simulink model "simulator_prototype_v2"  (R2021b)
(part 10 of 13)

t6667 = ct{1873};
t6668 = ct{1874};
t6669 = ct{1875};
t667 = ct{1876};
t6671 = ct{1877};
t6672 = ct{1878};
t6673 = ct{1879};
t6678 = ct{1880};
t6679 = ct{1881};
t668 = ct{1882};
t6680 = ct{1883};
t6681 = ct{1884};
t6687 = ct{1885};
t6688 = ct{1886};
t669 = ct{1887};
t6690 = ct{1888};
t6692 = ct{1889};
t6693 = ct{1890};
t670 = ct{1891};
t6714 = ct{1892};
t6715 = ct{1893};
t6731 = ct{1894};
t6732 = ct{1895};
t674 = ct{1896};
t6745 = ct{1897};
t6747 = ct{1898};
t6750 = ct{1899};
t6751 = ct{1900};
t677 = ct{1901};
t6788 = ct{1902};
t6789 = ct{1903};
t6804 = ct{1904};
t6808 = ct{1905};
t6810 = ct{1906};
t6811 = ct{1907};
t682 = ct{1908};
t6831 = ct{1909};
t6833 = ct{1910};
t684 = ct{1911};
t685 = ct{1912};
t6858 = ct{1913};
t6859 = ct{1914};
t686 = ct{1915};
t6860 = ct{1916};
t6861 = ct{1917};
t6868 = ct{1918};
t6869 = ct{1919};
t687 = ct{1920};
t6877 = ct{1921};
t6881 = ct{1922};
t6882 = ct{1923};
t6883 = ct{1924};
t6894 = ct{1925};
t6896 = ct{1926};
t6897 = ct{1927};
t6901 = ct{1928};
t6902 = ct{1929};
t6903 = ct{1930};
t6905 = ct{1931};
t6906 = ct{1932};
t6913 = ct{1933};
t6916 = ct{1934};
t6918 = ct{1935};
t6919 = ct{1936};
t6920 = ct{1937};
t6921 = ct{1938};
t6922 = ct{1939};
t6923 = ct{1940};
t6924 = ct{1941};
t6941 = ct{1942};
t6962 = ct{1943};
t6963 = ct{1944};
t6965 = ct{1945};
t6966 = ct{1946};
t6968 = ct{1947};
t6974 = ct{1948};
t6976 = ct{1949};
t6978 = ct{1950};
t6979 = ct{1951};
t6980 = ct{1952};
t6981 = ct{1953};
t6984 = ct{1954};
t6987 = ct{1955};
t6994 = ct{1956};
t7003 = ct{1957};
t7005 = ct{1958};
t7007 = ct{1959};
t7010 = ct{1960};
t7011 = ct{1961};
t7014 = ct{1962};
t7016 = ct{1963};
t7019 = ct{1964};
t7020 = ct{1965};
t7021 = ct{1966};
t7028 = ct{1967};
t7029 = ct{1968};
t7035 = ct{1969};
t7041 = ct{1970};
t7042 = ct{1971};
t7043 = ct{1972};
t7054 = ct{1973};
t7055 = ct{1974};
t7057 = ct{1975};
t7059 = ct{1976};
t707 = ct{1977};
t708 = ct{1978};
t7080 = ct{1979};
t7083 = ct{1980};
t7086 = ct{1981};
t7088 = ct{1982};
t7092 = ct{1983};
t7095 = ct{1984};
t7098 = ct{1985};
t71 = ct{1986};
t710 = ct{1987};
t7100 = ct{1988};
t7101 = ct{1989};
t7120 = ct{1990};
t7123 = ct{1991};
t7126 = ct{1992};
t7127 = ct{1993};
t7134 = ct{1994};
t7137 = ct{1995};
t7138 = ct{1996};
t7148 = ct{1997};
t715 = ct{1998};
t7150 = ct{1999};
t7159 = ct{2000};
t716 = ct{2001};
t7160 = ct{2002};
t7162 = ct{2003};
t7164 = ct{2004};
t7166 = ct{2005};
t7168 = ct{2006};
t7169 = ct{2007};
t7170 = ct{2008};
t7171 = ct{2009};
t7195 = ct{2010};
t7197 = ct{2011};
t7199 = ct{2012};
t7203 = ct{2013};
t7204 = ct{2014};
t7205 = ct{2015};
t7208 = ct{2016};
t721 = ct{2017};
t7210 = ct{2018};
t7211 = ct{2019};
t7212 = ct{2020};
t7213 = ct{2021};
t722 = ct{2022};
t7223 = ct{2023};
t7225 = ct{2024};
t7232 = ct{2025};
t7233 = ct{2026};
t724 = ct{2027};
t7246 = ct{2028};
t725 = ct{2029};
t7253 = ct{2030};
t7256 = ct{2031};
t7260 = ct{2032};
t7277 = ct{2033};
t7278 = ct{2034};
t7281 = ct{2035};
t7283 = ct{2036};
t7286 = ct{2037};
t7287 = ct{2038};
t7292 = ct{2039};
t7294 = ct{2040};
t7297 = ct{2041};
t7298 = ct{2042};
t73 = ct{2043};
t7300 = ct{2044};
t7301 = ct{2045};
t7304 = ct{2046};
t7309 = ct{2047};
t7310 = ct{2048};
t7311 = ct{2049};
t7315 = ct{2050};
t7319 = ct{2051};
t7322 = ct{2052};
t7323 = ct{2053};
t7335 = ct{2054};
t7337 = ct{2055};
t7339 = ct{2056};
t7340 = ct{2057};
t7344 = ct{2058};
t7345 = ct{2059};
t7348 = ct{2060};
t7349 = ct{2061};
t7358 = ct{2062};
t7360 = ct{2063};
t7364 = ct{2064};
t7365 = ct{2065};
t7366 = ct{2066};
t7376 = ct{2067};
t7379 = ct{2068};
t7380 = ct{2069};
t7385 = ct{2070};
t7387 = ct{2071};
t7388 = ct{2072};
t7401 = ct{2073};
t7402 = ct{2074};
t7403 = ct{2075};
t7404 = ct{2076};
t7405 = ct{2077};
t7406 = ct{2078};
t7410 = ct{2079};
t7411 = ct{2080};
t7412 = ct{2081};
t7413 = ct{2082};
t7416 = ct{2083};
t7417 = ct{2084};
t7435 = ct{2085};
t7436 = ct{2086};
t7458 = ct{2087};
t7459 = ct{2088};
t7468 = ct{2089};
t7479 = ct{2090};
t749 = ct{2091};
t7501 = ct{2092};
t7514 = ct{2093};
t7531 = ct{2094};
t7553 = ct{2095};
t7554 = ct{2096};
t7555 = ct{2097};
t7560 = ct{2098};
t7561 = ct{2099};
t762 = ct{2100};
t7624 = ct{2101};
t7626 = ct{2102};
t7641 = ct{2103};
t7658 = ct{2104};
t7659 = ct{2105};
t768 = ct{2106};
t7692 = ct{2107};
t7737 = ct{2108};
t777 = ct{2109};
t7784 = ct{2110};
t7789 = ct{2111};
t7790 = ct{2112};
t7827 = ct{2113};
t7828 = ct{2114};
t792 = ct{2115};
t793 = ct{2116};
t8 = ct{2117};
t801 = ct{2118};
t802 = ct{2119};
t808 = ct{2120};
t813 = ct{2121};
t819 = ct{2122};
t821 = ct{2123};
t850 = ct{2124};
t855 = ct{2125};
t874 = ct{2126};
t878 = ct{2127};
t9 = ct{2128};
t941 = ct{2129};
t948 = ct{2130};
t951 = ct{2131};
t97 = ct{2132};
t5423 = t3732+t3736+t4184+t4191;
t5428 = -t5427;
t5430 = t5427./2.0;
t5492 = -t5490;
t5496 = t5490./2.0;
t5547 = t5546./2.0;
t5582 = -t5580;
t5584 = t5580./2.0;
t5643 = -t5642;
t5671 = -t5669;
t5715 = -t5713;
t5767 = t4356+t5365;
t5771 = t4358+t5367;
t5791 = t4406+t5380;
t5820 = -t5819;
t5859 = t56+t73+t5856;
t5860 = t71+t97+t5856;
t5870 = -t5869;
t5882 = -t5881;
t5957 = -t5956;
t5958 = t329+t346+t5911;
t5962 = t354+t387+t5911;
t5977 = -t5976;
t5987 = -t5986;
t6010 = -t6009;
t6032 = t4727+t5706;
t6085 = -t6083;
t6086 = t6083./2.0;
t6088 = t6084./2.0;
t6108 = t4364+t5232+t5236;
t6112 = t6111./2.0;
t6121 = t6120./2.0;
t6139 = -t6137;
t6141 = t6140./2.0;
t6147 = -t6099.*(t1477-t2502);
t6149 = t6145./2.0;
t6150 = t3055.*t6100;
t6151 = t6099.*(t1477-t2502);
t6194 = t6193./2.0;
t6198 = -t6197;
t6200 = t6197./2.0;
t6202 = t6199./2.0;
t6218 = -t6215;
t6238 = -t6237;
t6253 = -t6251;
t6264 = t188.*t6242.*8.595599785252598e-1;
t6266 = -t6263;
t6268 = t50.*t189.*t6242.*9.543032792050485e-17;
t6280 = t640+t668+t669+t677+t1604+t1605+t1607+t1628+t2302+t2670+t2680+t2693+t2700+t3283+t3298+t3314+t3610+t3617+t3624+t3637+t4081+t4082;
t6289 = -t6287;
t6297 = t5856.*(t2694-t2701+t3036-t3043).*(t1513+t1879+t2598+t2820+t2834+t3117+t3118).*3.633675e-3;
t6302 = t201.*t6276.*6.246723209935546e-3;
t6319 = -t6318;
t6321 = t50.*t202.*t6276.*6.935255936130809e-19;
t6326 = t4019.*t6099;
t6330 = -t6100.*(t3242-t3554);
t6332 = t4031.*t6099;
t6333 = t4026.*t6100;
t6341 = t6337.*(-1.0./2.0);
t6344 = t6337./2.0;
t6346 = t6338./2.0;
t6357 = -t6356;
t6359 = t682+t715+t716+t725+t1741+t1742+t1750+t1754+t2401+t2697+t2712+t2715+t2721+t3334+t3346+t3367+t3656+t3660+t3664+t3678+t4135+t4136;
t6361 = t6360./2.0;
t6368 = -t6367;
t6371 = t3396.*t6244;
t6409 = (t5911.*(t2674-t2676+t3022-t3027).*(t1488+t1874+t2519+t2740+t2747+t3096+t3097))./2.0;
t6415 = -t6413;
t6427 = -t6384.*(t1477-t2502);
t6429 = t3055.*t6387;
t6433 = t6384.*(t1477-t2502).*(-1.0./2.0);
t6435 = (t6384.*(t1477-t2502))./2.0;
t6466 = -t6465;
t6467 = t6464./2.0;
t6469 = (t3217.*t6406)./2.0;
t6472 = -t6470;
t6489 = t4952+t4957+t4958+t4963;
t6490 = t4953+t4955+t4959+t4961;
t6493 = (t3502.*t6406)./2.0;
t6529 = t4019.*t6384;
t6532 = -t6387.*(t3242-t3554);
t6534 = t4026.*t6387;
t6535 = t6387.*(t3242-t3554);
t6536 = t4031.*t6384;
t6539 = (t3910.*t6406)./2.0;
t6548 = t4573.*t6244;
t6551 = -t6244.*(t3563-t4051);
t6567 = -t6566;
t6568 = t6566./2.0;
t6575 = t6573./2.0;
t6584 = t3690+t3699+t4854+t4857+t4860+t4870;
t6586 = t3696+t3697+t4852+t4859+t4864+t4866;
t6597 = -t6593;
t6647 = t5045+t6267;
t6664 = t6663./2.0;
t6670 = -t6669;
t6674 = t3771+t3784+t4973+t4976+t4984+t4994;
t6675 = t3774+t3777+t4970+t4979+t4987+t4989;
t6676 = t3774+t3779+t4965+t4979+t4987+t4992;
t6677 = t3772+t3788+t4971+t4974+t4985+t4997;
t6682 = t5062+t6310;
t6691 = -t6690;
t6696 = t5117+t5121+t5128+t5137;
t6697 = t5109+t5124+t5131+t5136;
t6698 = t5116+t5118+t5129+t5139;
t6699 = t5112+t5124+t5131+t5133;
t6704 = t21.*t2363.*t6681;
t6716 = t3003.*t6681;
t6733 = t3055.*t6681;
t6734 = -t6681.*(t1477-t2502);
t6735 = t6681.*(t1477-t2502).*(-1.0./2.0);
t6806 = -t21.*t6681.*(t1896-t3239);
t6807 = t21.*t3547.*t6681;
t6815 = -t6811;
t6829 = t5231+t5233+t5237+t5238;
t6836 = (t5857.*t5911)./2.0;
t6839 = (t5856.*t5946)./2.0;
t6870 = -t6869;
t6871 = t4019.*t6681;
t6872 = -t6681.*(t3242-t3554);
t6873 = t4026.*t6681;
t6874 = t6681.*(t3242-t3554);
t6875 = t4031.*t6681;
t6878 = -t6877;
t6879 = t3217.*(-t5231+t5235+t4604.*(t2813-t2835+t12.*(t1456-t2355).*1.02e-6+t17.*(t1456-t2355).*9.0e-8)+t4163.*(t3563-t4051)).*(-1.0./2.0);
t6880 = (t3217.*(-t5231+t5235+t4604.*(t2813-t2835+t12.*(t1456-t2355).*1.02e-6+t17.*(t1456-t2355).*9.0e-8)+t4163.*(t3563-t4051)))./2.0;
t6899 = t3502.*(-t5231+t5235+t4604.*(t2813-t2835+t12.*(t1456-t2355).*1.02e-6+t17.*(t1456-t2355).*9.0e-8)+t4163.*(t3563-t4051)).*(-1.0./2.0);
t6900 = (t3502.*(-t5231+t5235+t4604.*(t2813-t2835+t12.*(t1456-t2355).*1.02e-6+t17.*(t1456-t2355).*9.0e-8)+t4163.*(t3563-t4051)))./2.0;
t6904 = -t6903;
t6915 = t4361+t4368+t4935+t4936+t5031+t5032;
t6917 = t3908+t4321+t5021+t5023+t5056+t5057;
t6925 = t3910.*(-t5231+t5235+t4604.*(t2813-t2835+t12.*(t1456-t2355).*1.02e-6+t17.*(t1456-t2355).*9.0e-8)+t4163.*(t3563-t4051)).*(-1.0./2.0);
t6926 = (t3910.*(-t5231+t5235+t4604.*(t2813-t2835+t12.*(t1456-t2355).*1.02e-6+t17.*(t1456-t2355).*9.0e-8)+t4163.*(t3563-t4051)))./2.0;
t6942 = t3991.*(-t5231+t5235+t4604.*(t2813-t2835+t12.*(t1456-t2355).*1.02e-6+t17.*(t1456-t2355).*9.0e-8)+t4163.*(t3563-t4051)).*(-1.0./2.0);
t6969 = -t6968;
t6990 = t3848+t3850+t5156+t5169+t5184+t5188;
t6991 = t3845+t3857+t5162+t5164+t5183+t5192;
t6992 = t3843+t3862+t5163+t5167+t5182+t5189;
t6993 = t3850+t3855+t5159+t5169+t5184+t5187;
t6997 = t4872.*t6681;
t6998 = -t6681.*(t4165+t27.*(t1959-t3313+t38.*t1022.*(t855-t878).*2.196325630278387e-1));
t7008 = (t3217.*t6963)./2.0;
t7040 = (t3502.*t6963)./2.0;
t7058 = -t7057;
t7067 = -t3395.*(t3846-t5169-t5184+t5185+t3055.*(t2337+t12.*(t1456-t2355)).*9.3e-7+t4553.*(t3242-t3554).*9.3e-7);
t7070 = -t3396.*(t3840+t3862-t5164+t5167-t5183+t5189);
t7073 = t3395.*(t3846-t5169-t5184+t5185+t3055.*(t2337+t12.*(t1456-t2355)).*9.3e-7+t4553.*(t3242-t3554).*9.3e-7).*(-1.0./2.0);
t7075 = t3396.*(t3840+t3862-t5164+t5167-t5183+t5189);
t7090 = (t3910.*t6963)./2.0;
t7181 = -t4573.*(t3840+t3862-t5164+t5167-t5183+t5189);
t7184 = -t4577.*(t3846-t5169-t5184+t5185+t3055.*(t2337+t12.*(t1456-t2355)).*9.3e-7+t4553.*(t3242-t3554).*9.3e-7);
t7188 = -t4604.*(t3846-t5169-t5184+t5185+t3055.*(t2337+t12.*(t1456-t2355)).*9.3e-7+t4553.*(t3242-t3554).*9.3e-7);
t7191 = (t3563-t4051).*(t3840+t3862-t5164+t5167-t5183+t5189);
t7196 = t7195./2.0;
t7209 = -t7208;
t7214 = -t7212;
t7224 = -t7223;
t7226 = -t7225;
t7265 = t5856.*(t4853.*(t1896-t3239).*7.26735e-3+t2363.*(t684+t685-t710+t724+t1686-t1690+t1700+t1701+t2371+t2698+t2707-t2716+t2719+t3329-t3337-t3351-t3641+t3643+t3655-t3659+t4114+t4115).*7.26735e-3).*(-1.0./2.0);
t7271 = t5911.*(t4814.*(t1861-t3221)+t2297.*(t642+t643-t667+t674+t1587+t1606+t1608+t1609+t2295+t2671+t2683+t2684-t2695+t3279+t3297-t3303+t3597+t3603+t3609-t3614+t4053+t4054)).*(-1.0./2.0);
t7279 = t7278./2.0;
t7291 = t4345+t5051+t5151+t5152+t5661+t5663;
t7307 = t3489+t3498+t3783+t3785+t4692+t4694+t4698+t4700+t4967+t4977+t4991+t4993;
t7308 = t3492+t3495+t3775+t3794+t4691+t4696+t4697+t4702+t4969+t4972+t4986+t4998;
t7377 = t7376.*(-1.0./2.0);
t7378 = t7376./2.0;
t7382 = t3706+t3709+t3844+t3863+t4889+t4901+t4908+t4914+t5154+t5158+t5186+t5193;
t7383 = t3705+t3710+t3851+t3856+t4888+t4898+t4907+t4913+t5153+t5166+t5190+t5191;
t7389 = -t7388;
et244 = t3704+t3707-t3863+t4904+t4912-t5154+t5155-t5186+t3370.*(t1477-t2502).*9.3e-7+t4031.*(t3512-t4006).*9.0e-8+t12.*t3980.*(t3242-t3554).*9.0e-8;
et245 = t17.*t3980.*(t3242-t3554).*9.3e-7;
t7394 = -t3395.*(et244+et245);
t7395 = -t3396.*(t3703+t3708-t3856+t4903+t4911-t5153+t5161-t5190+t12.*t4887+t3370.*(t1477-t2502).*9.0e-8+t4031.*(t3512-t4006).*1.02e-6+t17.*t3980.*(t3242-t3554).*9.0e-8);
et246 = t3704+t3707-t3863+t4904+t4912-t5154+t5155-t5186+t3370.*(t1477-t2502).*9.3e-7+t4031.*(t3512-t4006).*9.0e-8+t12.*t3980.*(t3242-t3554).*9.0e-8;
et247 = t17.*t3980.*(t3242-t3554).*9.3e-7;
t7396 = t3395.*(et246+et247).*(-1.0./2.0);
t7397 = t3396.*(t3703+t3708-t3856+t4903+t4911-t5153+t5161-t5190+t12.*t4887+t3370.*(t1477-t2502).*9.0e-8+t4031.*(t3512-t4006).*1.02e-6+t17.*t3980.*(t3242-t3554).*9.0e-8);
t7407 = t5983+t6148+t6578;
t7422 = -t4573.*(t3703+t3708-t3856+t4903+t4911-t5153+t5161-t5190+t12.*t4887+t3370.*(t1477-t2502).*9.0e-8+t4031.*(t3512-t4006).*1.02e-6+t17.*t3980.*(t3242-t3554).*9.0e-8);
et248 = t3704+t3707-t3863+t4904+t4912-t5154+t5155-t5186+t3370.*(t1477-t2502).*9.3e-7+t4031.*(t3512-t4006).*9.0e-8+t12.*t3980.*(t3242-t3554).*9.0e-8;
et249 = t17.*t3980.*(t3242-t3554).*9.3e-7;
t7423 = -t4577.*(et248+et249);
et250 = t3704+t3707-t3863+t4904+t4912-t5154+t5155-t5186+t3370.*(t1477-t2502).*9.3e-7+t4031.*(t3512-t4006).*9.0e-8+t12.*t3980.*(t3242-t3554).*9.0e-8;
et251 = t17.*t3980.*(t3242-t3554).*9.3e-7;
t7424 = -t4604.*(et250+et251);
t7425 = (t3563-t4051).*(t3703+t3708-t3856+t4903+t4911-t5153+t5161-t5190+t12.*t4887+t3370.*(t1477-t2502).*9.0e-8+t4031.*(t3512-t4006).*1.02e-6+t17.*t3980.*(t3242-t3554).*9.0e-8);
t7432 = t6035+t6325+t6668;
t7433 = t6038+t6331+t6667;
t7437 = -t7436;
t7462 = t5012+t5254+t6254+t7137;
t7471 = t3055.*t7468;
t7473 = t5033+t5281+t6294+t7169;
t7477 = t3541+t3549+t3552+t3558+t5123+t5125+t5130+t5138+t5441+t5442+t5444+t5448;
t7478 = t3545+t3546+t3551+t3561+t5120+t5127+t5134+t5135+t5440+t5443+t5445+t5446;
t7481 = t6196+t6430+t6901;
t7482 = t2307.*(-t6196+t6428+t3055.*(-t4494-t4495+t4799+t4823+t3976.*(t2694-t2701+t3036-t3043).*4.0e-8+t3980.*(t2694-t2701+t3036-t3043).*2.4e-7)).*(-1.0./2.0);
t7483 = -t7468.*(t3242-t3554);
t7484 = t4026.*t7468;
t7485 = t7468.*(t3242-t3554);
t7520 = t3713+t3752+t3795+t3796+t5206+t5216+t5221+t5222+t5501+t5512+t5516+t5517;
t7521 = t3728+t3738+t3786+t3802+t5207+t5211+t5220+t5223+t5506+t5507+t5513+t5520;
t7532 = t7531./2.0;
et252 = t3395;
et253 = -t3728+t3729+t3782+t3800+t5208-t5220+t5503+t5504-t5513-t5520+t4553.*(t1005+t20.*(t1941-t3315+t39.*t1022.*(t855-t878).*2.196325630278387e-1)).*9.0e-8+t4151.*(t3512-t4006).*9.0e-8;
et254 = -1.0;
t7533 = et252.*et253.*et254;
et255 = t3395;
et256 = -t3728+t3729+t3782+t3800+t5208-t5220+t5503+t5504-t5513-t5520+t4553.*(t1005+t20.*(t1941-t3315+t39.*t1022.*(t855-t878).*2.196325630278387e-1)).*9.0e-8+t4151.*(t3512-t4006).*9.0e-8;
t7534 = et255.*et256;
t7535 = -t3396.*(-t3713+t3747+t3791+t3793+t5212-t5221+t5500+t5510-t5516-t5517+t4553.*(t1005+t20.*(t1941-t3315+t39.*t1022.*(t855-t878).*2.196325630278387e-1)).*1.02e-6+t4151.*(t3512-t4006).*1.02e-6);
et257 = t3396.*(-t3713+t3747+t3791+t3793+t5212-t5221+t5500+t5510-t5516-t5517+t4553.*(t1005+t20.*(t1941-t3315+t39.*t1022.*(t855-t878).*2.196325630278387e-1)).*1.02e-6+t4151.*(t3512-t4006).*1.02e-6);
et258 = -1.0./2.0;
t7538 = et257.*et258;
t7539 = t6286+t6530+t6981;
t7556 = -t7554;
t7562 = t3503.*(t6287+t4031.*(t4795+t4801+t4808+t3976.*(t2694-t2701+t3036-t3043).*5.7e-7)+t4026.*(-t4494-t4495+t4799+t4823+t3976.*(t2694-t2701+t3036-t3043).*4.0e-8+t3980.*(t2694-t2701+t3036-t3043).*2.4e-7)).*(-1.0./2.0);
t7569 = -t4573.*(-t3713+t3747+t3791+t3793+t5212-t5221+t5500+t5510-t5516-t5517+t4553.*(t1005+t20.*(t1941-t3315+t39.*t1022.*(t855-t878).*2.196325630278387e-1)).*1.02e-6+t4151.*(t3512-t4006).*1.02e-6);
et259 = t4577;
et260 = -t3728+t3729+t3782+t3800+t5208-t5220+t5503+t5504-t5513-t5520+t4553.*(t1005+t20.*(t1941-t3315+t39.*t1022.*(t855-t878).*2.196325630278387e-1)).*9.0e-8+t4151.*(t3512-t4006).*9.0e-8;
et261 = -1.0;
t7570 = et259.*et260.*et261;
t7571 = t4573.*(-t3713+t3747+t3791+t3793+t5212-t5221+t5500+t5510-t5516-t5517+t4553.*(t1005+t20.*(t1941-t3315+t39.*t1022.*(t855-t878).*2.196325630278387e-1)).*1.02e-6+t4151.*(t3512-t4006).*1.02e-6);
et262 = t4577;
et263 = -t3728+t3729+t3782+t3800+t5208-t5220+t5503+t5504-t5513-t5520+t4553.*(t1005+t20.*(t1941-t3315+t39.*t1022.*(t855-t878).*2.196325630278387e-1)).*9.0e-8+t4151.*(t3512-t4006).*9.0e-8;
t7572 = et262.*et263;
et264 = t4604;
et265 = -t3728+t3729+t3782+t3800+t5208-t5220+t5503+t5504-t5513-t5520+t4553.*(t1005+t20.*(t1941-t3315+t39.*t1022.*(t855-t878).*2.196325630278387e-1)).*9.0e-8+t4151.*(t3512-t4006).*9.0e-8;
et266 = -1.0;
t7573 = et264.*et265.*et266;
et267 = t3563-t4051;
et268 = -t3713+t3747+t3791+t3793+t5212-t5221+t5500+t5510-t5516-t5517+t4553.*(t1005+t20.*(t1941-t3315+t39.*t1022.*(t855-t878).*2.196325630278387e-1)).*1.02e-6+t4151.*(t3512-t4006).*1.02e-6;
t7574 = et267.*et268;
t7590 = t5509+t5511+t5515+t5521+t5600+t5601+t5605+t5611;
t7591 = t5505+t5514+t5518+t5519+t5597+t5606+t5608+t5609;
t7592 = -t3395.*(t5508-t5515+t5598+t5599-t5605-t5611+t4920.*(t3985+t12.*(t1861-t3221)).*9.3e-7+t4915.*(t3512-t4006).*9.0e-8);
t7593 = -t3396.*(t5502-t5518+t5596+t5602-t5608-t5609+t4920.*(t3985+t12.*(t1861-t3221)).*9.0e-8+t4915.*(t3512-t4006).*1.02e-6);
t7594 = t3395.*(t5508-t5515+t5598+t5599-t5605-t5611+t4920.*(t3985+t12.*(t1861-t3221)).*9.3e-7+t4915.*(t3512-t4006).*9.0e-8).*(-1.0./2.0);
t7595 = t3396.*(t5502-t5518+t5596+t5602-t5608-t5609+t4920.*(t3985+t12.*(t1861-t3221)).*9.0e-8+t4915.*(t3512-t4006).*1.02e-6);
t7612 = (t5946.*t7479)./2.0;
t7614 = (t5949.*t7479)./2.0;
t7620 = -t4573.*(t5502-t5518+t5596+t5602-t5608-t5609+t4920.*(t3985+t12.*(t1861-t3221)).*9.0e-8+t4915.*(t3512-t4006).*1.02e-6);
t7621 = -t4577.*(t5508-t5515+t5598+t5599-t5605-t5611+t4920.*(t3985+t12.*(t1861-t3221)).*9.3e-7+t4915.*(t3512-t4006).*9.0e-8);
t7622 = t4573.*(t5502-t5518+t5596+t5602-t5608-t5609+t4920.*(t3985+t12.*(t1861-t3221)).*9.0e-8+t4915.*(t3512-t4006).*1.02e-6);
t7623 = t4577.*(t5508-t5515+t5598+t5599-t5605-t5611+t4920.*(t3985+t12.*(t1861-t3221)).*9.3e-7+t4915.*(t3512-t4006).*9.0e-8);
t7625 = -t4604.*(t5508-t5515+t5598+t5599-t5605-t5611+t4920.*(t3985+t12.*(t1861-t3221)).*9.3e-7+t4915.*(t3512-t4006).*9.0e-8);
t7627 = (t3563-t4051).*(t5502-t5518+t5596+t5602-t5608-t5609+t4920.*(t3985+t12.*(t1861-t3221)).*9.0e-8+t4915.*(t3512-t4006).*1.02e-6);
t7643 = t3824+t3830+t3832+t3833+t5472+t5473+t5475+t5478+t5623+t5625+t5630+t5635;
t7644 = t3826+t3827+t3828+t3835+t5470+t5474+t5476+t5477+t5619+t5629+t5633+t5634;
t7685 = t7479.*(t4853.*(t1896-t3239).*7.26735e-3+t2363.*(t684+t685-t710+t724+t1686-t1690+t1700+t1701+t2371+t2698+t2707-t2716+t2719+t3329-t3337-t3351-t3641+t3643+t3655-t3659+t4114+t4115).*7.26735e-3).*(-1.0./2.0);
t7686 = (t7479.*(t4853.*(t1896-t3239).*7.26735e-3+t2363.*(t684+t685-t710+t724+t1686-t1690+t1700+t1701+t2371+t2698+t2707-t2716+t2719+t3329-t3337-t3351-t3641+t3643+t3655-t3659+t4114+t4115).*7.26735e-3))./2.0;
t7715 = t5863+t5971+t6034+t6216+t6411+t6604;
t7804 = t6113+t6211+t6285+t6487+t6714+t6921;
t7805 = t6114+t6213+t6288+t6488+t6715+t6922;
t7839 = ((t1861-t3221).*(-t6135+t6402-t7020+t7208+t7337+t21.*t6681.*(t1896-t3239)))./2.0;
t7841 = ((t2674-t2676+t3022-t3027).*(-t6135+t6402-t7020+t7208+t7337+t21.*t6681.*(t1896-t3239)))./2.0;
et269 = -t7387+t7553+t6058.*(t1005+t20.*(t1941-t3315+t39.*t1022.*(t855-t878).*2.196325630278387e-1))+t6681.*(t4165+t27.*(t1959-t3313+t38.*t1022.*(t855-t878).*2.196325630278387e-1))+t7292.*(t1896-t3239);
et270 = t4874.*(t3435-t3448+t4615+t4619+t3976.*(t1896-t3239).*5.7e-7+t3980.*(t1896-t3239).*4.0e-8);
t7919 = t3216.*(et269+et270).*(-1.0./2.0);
et271 = -t7387+t7553+t6058.*(t1005+t20.*(t1941-t3315+t39.*t1022.*(t855-t878).*2.196325630278387e-1))+t6681.*(t4165+t27.*(t1959-t3313+t38.*t1022.*(t855-t878).*2.196325630278387e-1))+t7292.*(t1896-t3239);
et272 = t4874.*(t3435-t3448+t4615+t4619+t3976.*(t1896-t3239).*5.7e-7+t3980.*(t1896-t3239).*4.0e-8);
t7920 = (t3216.*(et271+et272))./2.0;
et273 = -t7387+t7553+t6058.*(t1005+t20.*(t1941-t3315+t39.*t1022.*(t855-t878).*2.196325630278387e-1))+t6681.*(t4165+t27.*(t1959-t3313+t38.*t1022.*(t855-t878).*2.196325630278387e-1))+t7292.*(t1896-t3239);
et274 = t4874.*(t3435-t3448+t4615+t4619+t3976.*(t1896-t3239).*5.7e-7+t3980.*(t1896-t3239).*4.0e-8);
t7922 = ((et273+et274).*(t1861-t3221))./2.0;
t7938 = t6199+t6422+t6896+t7385+t7435+t7641;
t7946 = t6414+t6659+t7101+t7402+t7458+t7658;
t5409 = t50.*t189.*t5377.*9.543032792050485e-17;
t5417 = t2297.*t5377;
t5432 = t50.*t202.*t5398.*6.935255936130809e-19;
t5454 = t2363.*t5398.*7.26735e-3;
t5969 = t3934.*t5377.*(t1513+t1879+t2598+t2820+t2834+t3117+t3118).*(-3.633675e-3);
t5970 = t3934.*t5377.*(t1513+t1879+t2598+t2820+t2834+t3117+t3118).*3.633675e-3;
t5994 = t3910.*t5423.*(t1488+t1874+t2519+t2740+t2747+t3096+t3097).*(-1.0./2.0);
t5995 = (t3910.*t5423.*(t1488+t1874+t2519+t2740+t2747+t3096+t3097))./2.0;
t6087 = -t6086;
t6122 = -t6121;
t6152 = -t6149;
t6153 = t6151.*(-1.0./2.0);
t6156 = t6150./2.0;
t6160 = t5767.*(t2694-t2701+t3036-t3043).*(t1513+t1879+t2598+t2820+t2834+t3117+t3118).*3.633675e-3;
t6163 = t3934.*t5771.*(t1513+t1879+t2598+t2820+t2834+t3117+t3118).*(-3.633675e-3);
t6176 = t3910.*t5791.*(t1488+t1874+t2519+t2740+t2747+t3096+t3097).*(-1.0./2.0);
t6177 = t3934.*t3951.*t5859.*3.633675e-3;
t6178 = (t3910.*t5791.*(t1488+t1874+t2519+t2740+t2747+t3096+t3097))./2.0;
t6181 = t3934.*t3951.*t5860.*3.633675e-3;
t6188 = t3934.*t4018.*t5859.*3.633675e-3;
t6189 = t3934.*t4018.*t5860.*3.633675e-3;
t6195 = -t6194;
t6201 = -t6200;
t6204 = -t6202;
t6209 = t3934.*t4187.*t5859.*3.633675e-3;
t6210 = t3934.*t4187.*t5860.*3.633675e-3;
t6265 = -t6264;
t6269 = -t6268;
t6295 = (t3910.*t3925.*t5958)./2.0;
t6298 = -t6297;
t6299 = (t3910.*t3925.*t5962)./2.0;
t6309 = (t3910.*t3975.*t5958)./2.0;
t6312 = (t3910.*t3975.*t5962)./2.0;
t6322 = -t6321;
t6323 = t5859.*(t2694-t2701+t3036-t3043).*(t1513+t1879+t2598+t2820+t2834+t3117+t3118).*3.633675e-3;
t6328 = -t6326;
t6355 = (t3910.*t4146.*t5958)./2.0;
t6358 = (t3910.*t4146.*t5962)./2.0;
t6362 = -t6361;
t6363 = t2297.*t6280;
t6364 = t2307.*t6280;
t6365 = t2338.*t6280;
t6372 = -t6371;
t6373 = t6371./2.0;
t6391 = t2363.*t6359.*7.26735e-3;
t6392 = t2388.*t6359.*7.26735e-3;
t6393 = t2419.*t6359.*7.26735e-3;
t6410 = -t6409;
t6421 = (t5958.*(t2674-t2676+t3022-t3027).*(t1488+t1874+t2519+t2740+t2747+t3096+t3097))./2.0;
t6434 = -t6429;
t6436 = t6429./2.0;
t6449 = (t5369.*t5859)./2.0;
t6452 = (t5369.*t5860)./2.0;
t6458 = (t5373.*t5859)./2.0;
t6459 = (t5373.*t5860)./2.0;
t6468 = -t6467;
t6494 = -t6493;
t6499 = (t5423.*t5859)./2.0;
t6500 = (t5423.*t5860)./2.0;
t6504 = (t5275.*t5958)./2.0;
t6506 = (t5275.*t5962)./2.0;
t6521 = (t5317.*t5958)./2.0;
t6522 = (t5317.*t5962)./2.0;
t6540 = -t6539;
t6545 = (t5377.*t5958)./2.0;
t6546 = (t5377.*t5962)./2.0;
t6552 = t3395.*t6489;
t6553 = t3396.*t6490;
t6583 = t3693+t3695+t4851+t4858+t4865+t4868;
t6585 = t3692+t3699+t4854+t4856+t4862+t4870;
t6609 = t28.*t3055.*t6584;
t6610 = t22.*t3055.*t6586;
t6616 = t3143.*t6584;
t6617 = t3142.*t6586;
t6626 = t3257.*t6586;
t6627 = -t6584.*(t2527-t3009);
t6629 = t6584.*(t2527-t3009).*(-1.0./2.0);
t6631 = t3395.*t6584;
t6633 = t3396.*t6584;
t6636 = t3395.*t6586;
t6638 = t3396.*t6586;
t6648 = (t5791.*t5859)./2.0;
t6649 = (t5791.*t5860)./2.0;
t6683 = t4573.*t6490;
t6684 = t4577.*t6489;
t6685 = t4604.*t6489;
t6686 = -t6490.*(t3563-t4051);
t6700 = (t5767.*t5946)./2.0;
t6702 = (t5767.*t5949)./2.0;
t6705 = t6704./2.0;
t6706 = (t5771.*t5958)./2.0;
t6708 = (t5771.*t5962)./2.0;
t6717 = t6716./2.0;
t6718 = -t28.*t6584.*(t3242-t3554);
t6719 = t28.*t4026.*t6584;
t6720 = t28.*t6584.*(t3242-t3554);
t6721 = -t22.*t6586.*(t3242-t3554);
t6722 = t22.*t4026.*t6586;
t6723 = t22.*t6586.*(t3242-t3554);
t6724 = t28.*t3055.*t6674;
t6725 = t22.*t3055.*t6675;
t6740 = t3142.*t6675;
t6741 = t3143.*t6674;
t6752 = t3257.*t6675;
t6753 = -t6674.*(t2527-t3009);
t6756 = t6674.*(t2527-t3009);
t6758 = t4289.*t6584;
t6761 = t4290.*t6586;
t6762 = t4291.*t6584;
t6765 = t4292.*t6586;
t6766 = t22.*t3055.*t6699;
t6767 = t28.*t3055.*t6696;
t6772 = t3395.*t6674;
t6773 = t3395.*t6675;
t6774 = t3395.*t6676;
t6775 = t3396.*t6674;
t6776 = t3396.*t6675;
t6777 = t3396.*t6677;
t6791 = t3142.*t6699;
t6794 = t3143.*t6696;
t6801 = t3257.*t6699;
t6802 = -t6696.*(t2527-t3009);
t6805 = t6696.*(t2527-t3009).*(-1.0./2.0);
t6812 = t3395.*t6696;
t6813 = t3395.*t6697;
t6814 = t3395.*t6699;
t6816 = t3396.*t6696;
t6818 = t3396.*t6698;
t6819 = t3396.*t6699;
t6837 = (t5859.*t5904)./2.0;
t6840 = (t5855.*t5958)./2.0;
t6842 = t4573.*t6584;
t6845 = t4577.*t6584;
t6846 = t4573.*t6586;
t6847 = t4577.*t6586;
t6850 = t4604.*t6584;
t6851 = -t6584.*(t3563-t4051);
t6852 = t4604.*t6586;
t6854 = -t6586.*(t3563-t4051);
t6862 = -t28.*t6674.*(t3242-t3554);
t6863 = -t22.*t6675.*(t3242-t3554);
t6864 = t28.*t4026.*t6674;
t6865 = t22.*t4026.*t6675;
t6876 = -t6875;
t6884 = t4289.*t6674;
t6886 = t4290.*t6675;
t6887 = t4291.*t6674;
t6888 = t4292.*t6675;
t6890 = -t22.*t6699.*(t3242-t3554);
t6891 = -t28.*t6696.*(t3242-t3554);
t6892 = t22.*t4026.*t6699;
t6893 = t28.*t4026.*t6696;
t6907 = t4289.*t6696;
t6909 = t4290.*t6699;
t6910 = t4291.*t6696;
t6911 = t4292.*t6699;
t6927 = t4573.*t6674;
t6928 = t4573.*t6675;
t6929 = t4573.*t6677;
t6930 = t4577.*t6674;
t6932 = t4577.*t6675;
t6933 = t4577.*t6676;
t6934 = t4604.*t6674;
t6935 = t4604.*t6675;
t6936 = t4604.*t6676;
t6937 = -t6674.*(t3563-t4051);
t6938 = -t6675.*(t3563-t4051);
t6939 = -t6677.*(t3563-t4051);
t6940 = t6674.*(t3563-t4051);
t6944 = t4573.*t6696;
t6945 = t4573.*t6698;
t6946 = t4573.*t6699;
t6947 = t3951.*t6647.*(t2694-t2701+t3036-t3043).*(-3.633675e-3);
t6948 = t4577.*t6696;
t6949 = t4577.*t6697;
t6951 = t4577.*t6699;
t6952 = t4604.*t6696;
t6953 = t4604.*t6697;
t6954 = t4604.*t6699;
t6955 = -t6696.*(t3563-t4051);
t6956 = -t6698.*(t3563-t4051);
t6957 = -t6699.*(t3563-t4051);
t6958 = t6696.*(t3563-t4051);
t6964 = (t3217.*t6915)./2.0;
t6970 = t4187.*t6647.*(t2694-t2701+t3036-t3043).*(-3.633675e-3);
t6971 = t4187.*t6647.*(t2694-t2701+t3036-t3043).*3.633675e-3;
t6972 = (t3217.*t6917)./2.0;
t6982 = t3925.*t6682.*(t2674-t2676+t3022-t3027).*(-1.0./2.0);
t6983 = (t3925.*t6682.*(t2674-t2676+t3022-t3027))./2.0;
t6985 = (t3502.*t6915)./2.0;
t6995 = (t3502.*t6917)./2.0;
t6999 = t4146.*t6682.*(t2674-t2676+t3022-t3027).*(-1.0./2.0);
t7000 = (t4146.*t6682.*(t2674-t2676+t3022-t3027))./2.0;
t7009 = -t7008;
t7022 = t28.*t3055.*t6992;
t7023 = t22.*t3055.*t6993;
t7030 = (t3910.*t6915)./2.0;
t7032 = t3142.*t6993;
t7033 = t3143.*t6992;
t7044 = t5348.*t6584;
t7045 = t5350.*t6584;
t7046 = t6586.*(t4893-t28.*(t1005+t20.*(t1941-t3315+t39.*t1022.*(t855-t878).*2.196325630278387e-1)));
t7048 = (t3991.*t6915)./2.0;
t7050 = -t6586.*(t4171-t4896);
t7051 = (t3910.*t6917)./2.0;
t7060 = t3257.*t6993;
t7061 = -t6992.*(t2527-t3009);
t7063 = t6992.*(t2527-t3009).*(-1.0./2.0);
t7064 = (t3991.*t6917)./2.0;
t7068 = t3395.*t6992;
t7069 = t3395.*t6993;
t7071 = t3396.*t6992;
t7074 = t3396.*t6993;
t7077 = t7075.*(-1.0./2.0);
t7079 = t7075./2.0;
t7091 = -t7090;
et275 = t3582.*1.33637554986e-4+t3716-t3717+t27.*(t1896-t3239).*4.36041e-5;
et276 = t27.*t28.*(t1896-t3239).*7.26350557185e-5;
t7099 = t6647.*(et275+et276).*(-1.0./2.0);
t7104 = -t28.*t6992.*(t3242-t3554);
t7105 = -t22.*t6993.*(t3242-t3554);
t7106 = t28.*t4026.*t6992;
t7107 = t22.*t4026.*t6993;
t7110 = t6682.*(t3524.*1.838876e-2-t3591+t3592+t16.*(t1861-t3221).*(3.0./5.0e+2)+t16.*t17.*(t1861-t3221).*9.99471e-3).*(-1.0./2.0);
t7111 = t6647.*(t3359-t3670+t22.*(t3242-t3554).*1.33637554986e-4+t28.*(t3242-t3554).*7.26350557185e-5).*(-1.0./2.0);
t7118 = (t5313.*t6682)./2.0;
t7119 = t6675.*(t4893-t28.*(t1005+t20.*(t1941-t3315+t39.*t1022.*(t855-t878).*2.196325630278387e-1)));
t7121 = t5348.*t6674;
t7122 = t5350.*t6674;
t7124 = -t6675.*(t4171-t4896);
t7128 = t4289.*t6992;
t7129 = t4290.*t6993;
t7130 = t4291.*t6992;
t7133 = t4292.*t6993;
tau_c = ft_15({dq1,dq2,dq3,dq4,dq5,dq6,t10,t1005,t1022,t1089,t11,t1104,t1105,t1108,t1115,t1121,t1158,t1159,t1196,t12,t1205,t1210,t1212,t1217,t1218,t123,t1237,t1238,t1288,t1289,t13,t1302,t1303,t1319,t1320,t1336,t1348,t1350,t1351,t1360,t1369,t1378,t1396,t14,t140,t1425,t1435,t1456,t1477,t1488,t15,t1513,t1539,t1554,t1577,t1578,t1586,t1587,t16,t1600,t1606,t1608,t1609,t1629,t1637,t1640,t1641,t1659,t1661,t1666,t1667,t1683,t1686,t1690,t1692,t17,t1700,t1701,t1705,t1712,t1758,t1759,t1775,t1776,t18,t1861,t1874,t1879,t188,t1881,t189,t1896,t19,t1901,t1941,t1959,t1973,t1993,t1994,t20,t201,t202,t2023,t2053,t2060,t2089,t2090,t2098,t2099,t21,t2117,t2120,t2122,t2123,t2139,t2140,t2147,t2152,t2154,t2155,t2159,t2165,t2174,t2183,t2187,t2193,t2194,t2195,t2199,t22,t2203,t2215,t2219,t2222,t2223,t2239,t2240,t2256,t2257,t2292,t2295,t2297,t2303,t2306,t2307,t2308,t2317,t2337,t2338,t2339,t2355,t236,t2361,t2362,t2363,t2367,t2368,t237,t2371,t2378,t238,t2388,t2399,t24,t241,t2414,t2419,t25,t2502,t2510,t2519,t2527,t2530,t2555,t2556,t2572,t2583,t2598,t26,t2605,t2606,t2612,t2613,t2618,t2619,t262,t264,t2651,t2652,t2671,t2674,t2676,t2683,t2684,t2689,t2694,t2695,t2698,t27,t2701,t2707,t2716,t2719,t2740,t2747,t2748,t2749,t2754,t2773,t2781,t2788,t28,t2801,t2804,t2813,t2814,t2820,t2831,t2834,t2835,t2838,t2850,t2851,t29,t2953,t2965,t2966,t2975,t2979,t2990,t2991,t2994,t30,t3009,t3015,t3022,t3027,t3030,t3036,t3043,t3047,t3055,t3057,t3058,t3064,t3068,t3072,t3080,t3096,t3097,t31,t3109,t3117,t3118,t3121,t3122,t3126,t3129,t313,t3131,t3132,t3133,t314,t3145,t3148,t3157,t3158,t3171,t3193,t3194,t3195,t32,t3200,t3201,t3205,t3208,t3209,t321,t3211,t3213,t3216,t3217,t3221,t3235,t3236,t3237,t3238,t3239,t3242,t3276,t3277,t3279,t3290,t3297,t3299,t33,t3303,t3312,t3313,t3315,t3318,t332,t3322,t3324,t3328,t3329,t3337,t3340,t3344,t335,t3351,t3359,t3369,t3370,t3386,t3395,t3396,t34,t3405,t3409,t3415,t3416,t3420,t3423,t3428,t3431,t3432,t3434,t3435,t3446,t3448,t3463,t3468,t3471,t3474,t3480,t3482,t3483,t3488,t3490,t3496,t3499,t35,t350,t3500,t3502,t3503,t3512,t3517,t3524,t3543,t3547,t3554,t3563,t3566,t3582,t3588,t3590,t3591,t3592,t3597,t36,t3603,t3609,t3611,t3614,t3638,t3639,t3640,t3641,t3642,t3643,t3649,t3655,t3658,t3659,t366,t3670,t3688,t3689,t3703,t3704,t3707,t3708,t3712,t3716,t3717,t3739,t3746,t3755,t3765,t3766,t3770,t3781,t3789,t3790,t3792,t3797,t3798,t38,t3801,t3804,t3805,t3808,t3809,t3810,t3817,t3818,t3820,t3821,t3823,t3840,t3846,t3856,t3862,t3863,t3876,t3877,t3878,t3879,t3880,t3890,t3891,t3893,t3895,t3896,t3897,t3898,t39,t3901,t3902,t3903,t3906,t3910,t3913,t3915,t3924,t3925,t3926,t3931,t3934,t3937,t3943,t3951,t3961,t3967,t3968,t3974,t3975,t3976,t3980,t3985,t3991,t3993,t4001,t4006,t4008,t4018,t4019,t4026,t4030,t4031,t4032,t4035,t4039,t4041,t4045,t4047,t4049,t4051,t4053,t4054,t4065,t410,t4100,t4109,t4110,t4114,t4115,t4118,t4144,t4146,t4147,t4153,t4154,t4157,t4158,t4165,t4171,t4172,t4187,t4190,t4193,t4198,t42,t4201,t4205,t4208,t4213,t4215,t4236,t4240,t4244,t4260,t4261,t4263,t4270,t4272,t4273,t4274,t4275,t4281,t4282,t4286,t4287,t4288,t4299,t43,t4300,t4301,t4303,t4308,t4310,t4313,t4314,t4318,t4324,t4325,t4326,t4330,t4332,t4334,t4337,t4339,t4341,t4342,t4343,t4346,t4352,t4359,t4371,t4372,t4373,t4375,t4413,t4415,t4416,t4417,t4458,t4459,t4461,t4464,t4468,t4470,t4476,t4486,t4488,t4489,t4493,t4494,t4495,t4501,t4502,t4504,t4515,t4518,t4520,t4522,t4537,t4545,t4553,t4559,t4562,t4563,t4567,t4570,t4573,t4576,t4577,t4582,t4583,t4594,t46,t4603,t4604,t4606,t4615,t4617,t4618,t4619,t4623,t4634,t4635,t4639,t4644,t4645,t4651,t4652,t4658,t4663,t4665,t4673,t4675,t4676,t4677,t4678,t4680,t4683,t47,t4703,t4704,t4705,t4708,t4709,t4713,t4716,t4719,t4722,t4724,t4725,t4728,t4730,t4741,t4744,t4746,t4751,t4757,t4760,t4761,t4762,t4763,t4795,t4799,t4801,t4808,t4809,t4814,t4823,t4828,t4833,t4835,t4838,t4843,t4844,t4846,t4847,t4850,t4853,t4863,t4867,t4872,t4874,t4876,t4879,t4880,t4887,t4893,t4895,t4896,t4902,t4903,t4904,t4905,t4906,t4911,t4912,t4915,t4920,t4923,t4924,t4925,t4927,t4928,t4950,t4978,t4981,t4982,t4983,t4990,t4995,t4996,t4999,t50,t5001,t5003,t5004,t5005,t5007,t5009,t5010,t5011,t5013,t5014,t5016,t5025,t5026,t5027,t5028,t5034,t5035,t5036,t5037,t5038,t5041,t5042,t5043,t5046,t5049,t5063,t5080,t5082,t5083,t5084,t5085,t5086,t5087,t5088,t5089,t5090,t5091,t5093,t5096,t5097,t5098,t5103,t5105,t5106,t5108,t5113,t5119,t5126,t5141,t5142,t5153,t5154,t5155,t5161,t5164,t5167,t5169,t5183,t5184,t5185,t5186,t5189,t5190,t5194,t5197,t5198,t5199,t5200,t5201,t5202,t5205,t5213,t5214,t5234,t5236,t5240,t5243,t5246,t5247,t5248,t5249,t5251,t5255,t5256,t5257,t5258,t5259,t5262,t5264,t5265,t5275,t5278,t5279,t5280,t5283,t5286,t5287,t5291,t5296,t5297,t5301,t5302,t5303,t5304,t5305,t5306,t5308,t5309,t5312,t5313,t5317,t5328,t5331,t5332,t5333,t5336,t5337,t5340,t5341,t5343,t5344,t5345,t5346,t5348,t5350,t5352,t5353,t5356,t5358,t5359,t5361,t5362,t5363,t5369,t5370,t5372,t5373,t5374,t5376,t5377,t5381,t5382,t5383,t5384,t5385,t5386,t5387,t5389,t5390,t5391,t5392,t5393,t5395,t5399,t5400,t5401,t5402,t5403,t5404,t5405,t5409,t5410,t5411,t5412,t5413,t5415,t5416,t5417,t5419,t5421,t5422,t5423,t5425,t5428,t5430,t5432,t5433,t5434,t5436,t5437,t5438,t5439,t5449,t5451,t5452,t5453,t5454,t5455,t5456,t5457,t5458,t5459,t5460,t5464,t5465,t5466,t5467,t5468,t5480,t5481,t5483,t5486,t5487,t5488,t5489,t5490,t5491,t5492,t5493,t5494,t5495,t5496,t5497,t5499,t5508,t5515,t5523,t5535,t5536,t5537,t5538,t5539,t5542,t5543,t5544,t5545,t5546,t5547,t5548,t5549,t5550,t5551,t5552,t5553,t5554,t5555,t5556,t5557,t5558,t5560,t5563,t5564,t5565,t5567,t5568,t5569,t5570,t5572,t5573,t5574,t5575,t5576,t5577,t5578,t5579,t5580,t5581,t5582,t5583,t5584,t5585,t5586,t5587,t5588,t5589,t5590,t5591,t5592,t5593,t5594,t5598,t5599,t56,t5603,t5604,t5605,t5607,t5611,t5612,t5613,t5614,t5615,t5616,t5618,t5622,t5624,t5626,t5628,t5631,t5632,t5636,t5637,t5638,t5641,t5642,t5643,t5645,t5646,t5647,t5649,t5650,t5651,t5652,t5653,t5655,t5658,t5659,t5669,t5670,t5671,t5672,t5673,t5675,t5677,t5678,t5679,t5680,t5681,t5682,t5683,t5684,t5685,t5686,t5687,t5688,t5689,t5690,t5691,t5694,t5695,t5698,t5699,t5709,t5710,t5711,t5712,t5713,t5714,t5715,t5716,t5717,t5718,t5720,t5721,t5722,t5723,t5724,t5725,t5730,t5731,t5734,t5735,t5738,t5739,t5741,t5742,t5745,t5747,t5751,t5753,t5754,t5756,t5758,t5759,t5760,t5761,t5762,t5763,t5764,t5765,t5766,t5767,t5768,t5769,t5770,t5771,t5772,t5773,t5774,t5775,t5776,t5777,t5778,t5779,t5781,t5782,t5783,t5784,t5787,t5788,t5790,t5791,t5792,t5793,t5794,t5795,t5796,t5798,t5799,t5801,t5802,t5804,t5809,t5810,t5813,t5814,t5816,t5817,t5819,t5820,t5821,t5825,t5826,t5827,t5828,t5829,t5831,t5832,t5833,t5835,t5836,t5837,t5838,t5839,t5840,t5842,t5844,t5845,t5846,t5849,t5851,t5852,t5853,t5855,t5856,t5857,t5858,t5859,t5860,t5864,t5867,t5868,t5869,t5870,t5871,t5872,t5874,t5875,t5876,t5877,t5878,t5879,t5880,t5881,t5882,t5884,t5886,t5888,t5890,t5891,t5892,t5893,t5894,t5896,t5897,t5898,t5899,t5900,t5901,t5902,t5904,t5905,t5906,t5907,t5908,t5909,t5910,t5911,t5912,t5913,t5914,t5915,t5916,t5917,t5918,t5919,t5920,t5922,t5923,t5924,t5925,t5926,t5927,t5928,t5930,t5931,t5933,t5934,t5935,t5937,t5938,t5939,t5941,t5942,t5943,t5945,t5946,t5947,t5948,t5949,t5950,t5951,t5954,t5955,t5956,t5957,t5958,t5959,t5960,t5962,t5963,t5965,t5966,t5967,t5968,t5969,t5970,t5973,t5974,t5975,t5976,t5977,t5978,t5979,t5980,t5981,t5982,t5984,t5985,t5986,t5988,t5990,t5992,t5993,t5994,t5995,t5997,t5999,t60,t6000,t6001,t6004,t6005,t6006,t6007,t6008,t6009,t6010,t6011,t6013,t6014,t6015,t6017,t6018,t6019,t6020,t6021,t6022,t6023,t6024,t6026,t6027,t6028,t6029,t6031,t6032,t6037,t6039,t6041,t6043,t6045,t6046,t6047,t6050,t6052,t6053,t6054,t6055,t6058,t6059,t6060,t6062,t6064,t6065,t6066,t6067,t6074,t6076,t6079,t6080,t6081,t6082,t6083,t6084,t6085,t6086,t6087,t6088,t6091,t6093,t6094,t6095,t6096,t6098,t6100,t6102,t6106,t6107,t6109,t6110,t6111,t6112,t6115,t6116,t6119,t6120,t6121,t6125,t6129,t6131,t6133,t6134,t6135,t6136,t6137,t6138,t6139,t6140,t6141,t6143,t6144,t6145,t6149,t6150,t6151,t6152,t6153,t6156,t6159,t6160,t6162,t6164,t6166,t6168,t6169,t6170,t6171,t6172,t6173,t6174,t6175,t6177,t6178,t6180,t6181,t6183,t6184,t6185,t6186,t6187,t6188,t6189,t6190,t6191,t6192,t6193,t6194,t6195,t6196,t6198,t6200,t6201,t6202,t6205,t6206,t6207,t6208,t6209,t6210,t6217,t6218,t6219,t6223,t6225,t6226,t6227,t6228,t6231,t6232,t6233,t6234,t6237,t6238,t6239,t6240,t6241,t6244,t6250,t6251,t6252,t6253,t6255,t6256,t6257,t6262,t6263,t6265,t6266,t6269,t6270,t6271,t6272,t6275,t6281,t6282,t6283,t6284,t6287,t6289,t6290,t6291,t6292,t6293,t6295,t6297,t6298,t6299,t6302,t6303,t6304,t6306,t6307,t6308,t6309,t6311,t6312,t6313,t6314,t6316,t6317,t6319,t6322,t6323,t6324,t6326,t6327,t6328,t6329,t6330,t6332,t6333,t6334,t6337,t6338,t6339,t6341,t6342,t6343,t6345,t6346,t6347,t6348,t6354,t6355,t6357,t6358,t6360,t6361,t6362,t6363,t6364,t6365,t6366,t6367,t6368,t6369,t6371,t6372,t6373,t6375,t6376,t6377,t6379,t6384,t6391,t6392,t6393,t6394,t6396,t6398,t6402,t6404,t6405,t6407,t6408,t6409,t6410,t6412,t6413,t6415,t6417,t6418,t6419,t642,t6420,t6421,t6423,t6425,t6426,t6427,t6428,t6429,t643,t6431,t6432,t6433,t6434,t6435,t6436,t6438,t6439,t6440,t6441,t6442,t6443,t6444,t6445,t6446,t6447,t6449,t6452,t6455,t6457,t6458,t6459,t6460,t6461,t6462,t6463,t6464,t6465,t6466,t6467,t6468,t6469,t6471,t6472,t6473,t6474,t6475,t6476,t6477,t6478,t6480,t6481,t6482,t6483,t6484,t649,t6490,t6491,t6493,t6496,t6498,t6499,t6500,t6501,t6502,t6503,t6504,t6506,t6508,t6509,t6510,t6511,t6512,t6513,t6514,t6515,t6517,t6518,t6519,t6520,t6521,t6522,t6523,t6524,t6525,t6526,t6527,t6528,t6529,t6531,t6534,t6535,t6536,t6537,t6538,t6539,t6540,t6542,t6544,t6545,t6546,t6547,t6548,t6549,t6550,t6551,t6552,t6553,t6559,t6560,t6561,t6562,t6564,t6565,t6567,t6568,t6569,t6570,t6571,t6572,t6573,t6574,t6575,t6576,t6579,t6580,t6582,t6583,t6584,t6585,t6588,t6589,t6591,t6592,t6593,t6594,t6595,t6596,t6597,t6598,t6599,t6600,t6601,t6602,t6605,t6606,t6607,t6608,t6609,t6610,t6616,t6617,t6622,t6623,t6624,t6625,t6626,t6627,t6629,t6631,t6633,t6636,t6638,t6645,t6646,t6647,t6648,t6649,t6651,t6652,t6654,t6656,t6657,t6658,t6660,t6663,t6664,t6665,t667,t6670,t6671,t6672,t6673,t6674,t6675,t6678,t6679,t6680,t6681,t6682,t6683,t6684,t6685,t6686,t6687,t6688,t6690,t6691,t6692,t6693,t6696,t6699,t670,t6700,t6702,t6704,t6705,t6706,t6708,t6716,t6717,t6719,t6720,t6722,t6723,t6724,t6725,t6731,t6732,t6733,t6734,t674,t6740,t6741,t6745,t6747,t6750,t6751,t6752,t6756,t6758,t6761,t6762,t6765,t6766,t6767,t6772,t6773,t6774,t6775,t6776,t6777,t6788,t6789,t6791,t6794,t6801,t6802,t6804,t6806,t6807,t6808,t6810,t6812,t6813,t6814,t6815,t6816,t6818,t6819,t6831,t6833,t6836,t6837,t6839,t684,t6840,t6842,t6845,t6846,t6847,t685,t6850,t6851,t6852,t6854,t6858,t6859,t686,t6860,t6861,t6862,t6863,t6864,t6865,t6868,t687,t6870,t6871,t6872,t6873,t6874,t6875,t6876,t6877,t6878,t6879,t6880,t6881,t6882,t6883,t6884,t6886,t6887,t6888,t6890,t6891,t6892,t6893,t6894,t6897,t6900,t6902,t6903,t6904,t6905,t6906,t6907,t6909,t6910,t6911,t6913,t6916,t6918,t6919,t6920,t6923,t6924,t6925,t6926,t6927,t6928,t6929,t6930,t6932,t6933,t6934,t6935,t6936,t6938,t6939,t6940,t6941,t6942,t6944,t6945,t6946,t6948,t6949,t6951,t6952,t6953,t6954,t6956,t6957,t6958,t6962,t6964,t6965,t6966,t6968,t6971,t6972,t6974,t6976,t6978,t6979,t6980,t6983,t6984,t6985,t6987,t6992,t6993,t6994,t6995,t6997,t6998,t7000,t7003,t7005,t7007,t7009,t7010,t7011,t7014,t7016,t7019,t7020,t7021,t7022,t7023,t7028,t7029,t7030,t7032,t7033,t7035,t7040,t7041,t7042,t7043,t7044,t7045,t7046,t7048,t7050,t7051,t7054,t7055,t7057,t7059,t7060,t7061,t7063,t7064,t7067,t7068,t7069,t707,t7071,t7073,t7074,t7075,t7079,t708,t7080,t7083,t7086,t7088,t7090,t7092,t7095,t7098,t710,t7100,t7101,t7104,t7105,t7106,t7107,t7111,t7118,t7119,t7120,t7121,t7122,t7123,t7124,t7126,t7127,t7128,t7129,t7130,t7133,t7134,t7138,t7148,t7150,t7159,t7160,t7162,t7164,t7166,t7168,t7170,t7171,t7181,t7184,t7188,t7191,t7195,t7196,t7197,t7199,t7203,t7204,t7205,t7208,t7209,t721,t7210,t7211,t7213,t7214,t722,t7224,t7226,t7232,t7233,t724,t7246,t7253,t7256,t7260,t7265,t7271,t7277,t7278,t7279,t7281,t7283,t7286,t7287,t7291,t7292,t7294,t7297,t7298,t7300,t7301,t7304,t7307,t7308,t7309,t7310,t7311,t7315,t7319,t7322,t7323,t7335,t7337,t7339,t7340,t7344,t7345,t7348,t7349,t7358,t7360,t7364,t7365,t7366,t7376,t7378,t7379,t7380,t7385,t7387,t7388,t7389,t7394,t7396,t7397,t7401,t7402,t7403,t7404,t7405,t7406,t7407,t7410,t7411,t7412,t7413,t7416,t7417,t7422,t7423,t7424,t7425,t7432,t7433,t7436,t7458,t7459,t7462,t7471,t7473,t7477,t7478,t7479,t7482,t7483,t7484,t7485,t749,t7501,t7514,t7531,t7532,t7534,t7535,t7538,t7553,t7554,t7555,t7556,t7560,t7561,t7562,t7571,t7572,t7573,t7574,t7592,t7595,t7612,t7614,t762,t7622,t7623,t7624,t7625,t7626,t7627,t7641,t7643,t7644,t7658,t7659,t768,t7686,t7692,t7715,t7737,t777,t7784,t7789,t7790,t7804,t7805,t7827,t7828,t7839,t7841,t7919,t792,t7920,t7922,t793,t7938,t8,t801,t802,t808,t813,t819,t821,t850,t855,t874,t878,t9,t941,t948,t951});
end
function tau_c = ft_15(ct)
dq1 = ct{1};
dq2 = ct{2};
dq3 = ct{3};
dq4 = ct{4};
dq5 = ct{5};
dq6 = ct{6};
t10 = ct{7};
t1005 = ct{8};
t1022 = ct{9};
t1089 = ct{10};
t11 = ct{11};
t1104 = ct{12};
t1105 = ct{13};
t1108 = ct{14};
t1115 = ct{15};
t1121 = ct{16};
t1158 = ct{17};
t1159 = ct{18};
t1196 = ct{19};
t12 = ct{20};
t1205 = ct{21};
t1210 = ct{22};
t1212 = ct{23};
t1217 = ct{24};
t1218 = ct{25};
t123 = ct{26};
t1237 = ct{27};
t1238 = ct{28};
t1288 = ct{29};
t1289 = ct{30};
t13 = ct{31};
t1302 = ct{32};
t1303 = ct{33};
t1319 = ct{34};
t1320 = ct{35};
t1336 = ct{36};
t1348 = ct{37};
t1350 = ct{38};
t1351 = ct{39};
t1360 = ct{40};
t1369 = ct{41};
t1378 = ct{42};
t1396 = ct{43};
t14 = ct{44};
t140 = ct{45};
t1425 = ct{46};
t1435 = ct{47};
t1456 = ct{48};
t1477 = ct{49};
t1488 = ct{50};
t15 = ct{51};
t1513 = ct{52};
t1539 = ct{53};
t1554 = ct{54};
t1577 = ct{55};
t1578 = ct{56};
t1586 = ct{57};
t1587 = ct{58};
t16 = ct{59};
t1600 = ct{60};
t1606 = ct{61};
t1608 = ct{62};
t1609 = ct{63};
t1629 = ct{64};
t1637 = ct{65};
t1640 = ct{66};
t1641 = ct{67};
t1659 = ct{68};
t1661 = ct{69};
t1666 = ct{70};
t1667 = ct{71};
t1683 = ct{72};
t1686 = ct{73};
t1690 = ct{74};
t1692 = ct{75};
t17 = ct{76};
t1700 = ct{77};
t1701 = ct{78};
t1705 = ct{79};
t1712 = ct{80};
t1758 = ct{81};
t1759 = ct{82};
t1775 = ct{83};
t1776 = ct{84};
t18 = ct{85};
t1861 = ct{86};
t1874 = ct{87};
t1879 = ct{88};
t188 = ct{89};
t1881 = ct{90};
t189 = ct{91};
t1896 = ct{92};
t19 = ct{93};
t1901 = ct{94};
t1941 = ct{95};
t1959 = ct{96};
t1973 = ct{97};
t1993 = ct{98};
t1994 = ct{99};
t20 = ct{100};
t201 = ct{101};
t202 = ct{102};
t2023 = ct{103};
t2053 = ct{104};
t2060 = ct{105};
t2089 = ct{106};
t2090 = ct{107};
t2098 = ct{108};
t2099 = ct{109};
t21 = ct{110};
t2117 = ct{111};
t2120 = ct{112};
t2122 = ct{113};
t2123 = ct{114};
t2139 = ct{115};
t2140 = ct{116};
t2147 = ct{117};
t2152 = ct{118};
t2154 = ct{119};
t2155 = ct{120};
t2159 = ct{121};
t2165 = ct{122};
t2174 = ct{123};
t2183 = ct{124};
t2187 = ct{125};
t2193 = ct{126};
t2194 = ct{127};
t2195 = ct{128};
t2199 = ct{129};
t22 = ct{130};
t2203 = ct{131};
t2215 = ct{132};
t2219 = ct{133};
t2222 = ct{134};
t2223 = ct{135};
t2239 = ct{136};
t2240 = ct{137};
t2256 = ct{138};
t2257 = ct{139};
t2292 = ct{140};
t2295 = ct{141};
t2297 = ct{142};
t2303 = ct{143};
t2306 = ct{144};
t2307 = ct{145};
t2308 = ct{146};
t2317 = ct{147};
t2337 = ct{148};
t2338 = ct{149};
t2339 = ct{150};
t2355 = ct{151};
t236 = ct{152};
t2361 = ct{153};
t2362 = ct{154};
t2363 = ct{155};
t2367 = ct{156};
t2368 = ct{157};
t237 = ct{158};
t2371 = ct{159};
t2378 = ct{160};
t238 = ct{161};
t2388 = ct{162};
t2399 = ct{163};
t24 = ct{164};
t241 = ct{165};
t2414 = ct{166};
t2419 = ct{167};
t25 = ct{168};
t2502 = ct{169};
t2510 = ct{170};
t2519 = ct{171};
t2527 = ct{172};
t2530 = ct{173};
t2555 = ct{174};
t2556 = ct{175};
t2572 = ct{176};
t2583 = ct{177};
t2598 = ct{178};
t26 = ct{179};
t2605 = ct{180};
t2606 = ct{181};
t2612 = ct{182};
t2613 = ct{183};
t2618 = ct{184};
t2619 = ct{185};
t262 = ct{186};
t264 = ct{187};
t2651 = ct{188};
t2652 = ct{189};
t2671 = ct{190};
t2674 = ct{191};
t2676 = ct{192};
t2683 = ct{193};
t2684 = ct{194};
t2689 = ct{195};
t2694 = ct{196};
t2695 = ct{197};
t2698 = ct{198};
t27 = ct{199};
t2701 = ct{200};
t2707 = ct{201};
t2716 = ct{202};
t2719 = ct{203};
t2740 = ct{204};
t2747 = ct{205};
t2748 = ct{206};
t2749 = ct{207};
t2754 = ct{208};
t2773 = ct{209};
t2781 = ct{210};
t2788 = ct{211};
t28 = ct{212};
t2801 = ct{213};
t2804 = ct{214};
t2813 = ct{215};
t2814 = ct{216};
t2820 = ct{217};
t2831 = ct{218};
t2834 = ct{219};
t2835 = ct{220};
t2838 = ct{221};
t2850 = ct{222};
t2851 = ct{223};
t29 = ct{224};
t2953 = ct{225};
t2965 = ct{226};
t2966 = ct{227};
t2975 = ct{228};
t2979 = ct{229};
t2990 = ct{230};
t2991 = ct{231};
t2994 = ct{232};
t30 = ct{233};
t3009 = ct{234};
t3015 = ct{235};
t3022 = ct{236};
t3027 = ct{237};
t3030 = ct{238};
t3036 = ct{239};
t3043 = ct{240};
t3047 = ct{241};
t3055 = ct{242};
t3057 = ct{243};
t3058 = ct{244};
t3064 = ct{245};
t3068 = ct{246};
t3072 = ct{247};
t3080 = ct{248};
t3096 = ct{249};
t3097 = ct{250};
t31 = ct{251};
t3109 = ct{252};
t3117 = ct{253};
t3118 = ct{254};
t3121 = ct{255};
t3122 = ct{256};
t3126 = ct{257};
t3129 = ct{258};
t313 = ct{259};
t3131 = ct{260};
t3132 = ct{261};
t3133 = ct{262};
t314 = ct{263};
t3145 = ct{264};
t3148 = ct{265};
t3157 = ct{266};
t3158 = ct{267};
t3171 = ct{268};
t3193 = ct{269};
t3194 = ct{270};
t3195 = ct{271};
t32 = ct{272};
t3200 = ct{273};
t3201 = ct{274};
t3205 = ct{275};
t3208 = ct{276};
t3209 = ct{277};
t321 = ct{278};
t3211 = ct{279};
t3213 = ct{280};
t3216 = ct{281};
t3217 = ct{282};
t3221 = ct{283};
t3235 = ct{284};
t3236 = ct{285};
t3237 = ct{286};
t3238 = ct{287};
t3239 = ct{288};
t3242 = ct{289};
t3276 = ct{290};
t3277 = ct{291};
t3279 = ct{292};
t3290 = ct{293};
t3297 = ct{294};
t3299 = ct{295};
t33 = ct{296};
t3303 = ct{297};
t3312 = ct{298};
t3313 = ct{299};
t3315 = ct{300};
t3318 = ct{301};
t332 = ct{302};
t3322 = ct{303};
t3324 = ct{304};
t3328 = ct{305};
t3329 = ct{306};
t3337 = ct{307};
t3340 = ct{308};
t3344 = ct{309};
t335 = ct{310};
t3351 = ct{311};
t3359 = ct{312};
t3369 = ct{313};
t3370 = ct{314};
t3386 = ct{315};
t3395 = ct{316};
t3396 = ct{317};
t34 = ct{318};
t3405 = ct{319};
t3409 = ct{320};
t3415 = ct{321};
t3416 = ct{322};
t3420 = ct{323};
t3423 = ct{324};
t3428 = ct{325};
t3431 = ct{326};
t3432 = ct{327};
t3434 = ct{328};
t3435 = ct{329};
t3446 = ct{330};
t3448 = ct{331};
t3463 = ct{332};
t3468 = ct{333};
t3471 = ct{334};
t3474 = ct{335};
t3480 = ct{336};
t3482 = ct{337};
t3483 = ct{338};
t3488 = ct{339};
t3490 = ct{340};
t3496 = ct{341};
t3499 = ct{342};
t35 = ct{343};
t350 = ct{344};
t3500 = ct{345};
t3502 = ct{346};
t3503 = ct{347};
t3512 = ct{348};
t3517 = ct{349};
t3524 = ct{350};
t3543 = ct{351};
t3547 = ct{352};
t3554 = ct{353};
t3563 = ct{354};
t3566 = ct{355};
t3582 = ct{356};
t3588 = ct{357};
t3590 = ct{358};
t3591 = ct{359};
t3592 = ct{360};
t3597 = ct{361};
t36 = ct{362};
t3603 = ct{363};
t3609 = ct{364};
t3611 = ct{365};
t3614 = ct{366};
t3638 = ct{367};
t3639 = ct{368};
t3640 = ct{369};
t3641 = ct{370};
t3642 = ct{371};
t3643 = ct{372};
t3649 = ct{373};
t3655 = ct{374};
t3658 = ct{375};
t3659 = ct{376};
t366 = ct{377};
t3670 = ct{378};
t3688 = ct{379};
t3689 = ct{380};
t3703 = ct{381};
t3704 = ct{382};
t3707 = ct{383};
t3708 = ct{384};
t3712 = ct{385};
t3716 = ct{386};
t3717 = ct{387};
t3739 = ct{388};
t3746 = ct{389};
t3755 = ct{390};
t3765 = ct{391};
t3766 = ct{392};
t3770 = ct{393};
t3781 = ct{394};
t3789 = ct{395};
t3790 = ct{396};
t3792 = ct{397};
t3797 = ct{398};
t3798 = ct{399};
t38 = ct{400};
t3801 = ct{401};
t3804 = ct{402};
t3805 = ct{403};
t3808 = ct{404};
t3809 = ct{405};
t3810 = ct{406};
t3817 = ct{407};
t3818 = ct{408};
t3820 = ct{409};
t3821 = ct{410};
t3823 = ct{411};
t3840 = ct{412};
t3846 = ct{413};
t3856 = ct{414};
t3862 = ct{415};
t3863 = ct{416};
t3876 = ct{417};
t3877 = ct{418};
t3878 = ct{419};
t3879 = ct{420};
t3880 = ct{421};
t3890 = ct{422};
t3891 = ct{423};
t3893 = ct{424};
t3895 = ct{425};
t3896 = ct{426};
t3897 = ct{427};
t3898 = ct{428};
t39 = ct{429};
t3901 = ct{430};
t3902 = ct{431};
t3903 = ct{432};
t3906 = ct{433};
t3910 = ct{434};
t3913 = ct{435};
t3915 = ct{436};
t3924 = ct{437};
t3925 = ct{438};
t3926 = ct{439};
t3931 = ct{440};
t3934 = ct{441};
t3937 = ct{442};
t3943 = ct{443};
t3951 = ct{444};
t3961 = ct{445};
t3967 = ct{446};
t3968 = ct{447};
t3974 = ct{448};
t3975 = ct{449};
t3976 = ct{450};
t3980 = ct{451};
t3985 = ct{452};
t3991 = ct{453};
t3993 = ct{454};
t4001 = ct{455};
t4006 = ct{456};
t4008 = ct{457};
t4018 = ct{458};
t4019 = ct{459};
t4026 = ct{460};
t4030 = ct{461};
t4031 = ct{462};
t4032 = ct{463};
t4035 = ct{464};
t4039 = ct{465};
t4041 = ct{466};
t4045 = ct{467};
t4047 = ct{468};
t4049 = ct{469};
t4051 = ct{470};
t4053 = ct{471};
t4054 = ct{472};
t4065 = ct{473};
t410 = ct{474};
t4100 = ct{475};
t4109 = ct{476};
t4110 = ct{477};
t4114 = ct{478};
t4115 = ct{479};
t4118 = ct{480};
t4144 = ct{481};
t4146 = ct{482};
t4147 = ct{483};
t4153 = ct{484};
t4154 = ct{485};
t4157 = ct{486};
t4158 = ct{487};
t4165 = ct{488};
t4171 = ct{489};
t4172 = ct{490};
t4187 = ct{491};
t4190 = ct{492};
t4193 = ct{493};
t4198 = ct{494};
t42 = ct{495};
t4201 = ct{496};
t4205 = ct{497};
t4208 = ct{498};
t4213 = ct{499};
t4215 = ct{500};
t4236 = ct{501};
t4240 = ct{502};
t4244 = ct{503};
t4260 = ct{504};
t4261 = ct{505};
t4263 = ct{506};
t4270 = ct{507};
t4272 = ct{508};
t4273 = ct{509};
t4274 = ct{510};
t4275 = ct{511};
t4281 = ct{512};
t4282 = ct{513};
t4286 = ct{514};
t4287 = ct{515};
t4288 = ct{516};
t4299 = ct{517};
t43 = ct{518};
t4300 = ct{519};
t4301 = ct{520};
t4303 = ct{521};
t4308 = ct{522};
t4310 = ct{523};
t4313 = ct{524};
t4314 = ct{525};
t4318 = ct{526};
t4324 = ct{527};
t4325 = ct{528};
t4326 = ct{529};
t4330 = ct{530};
t4332 = ct{531};
t4334 = ct{532};
t4337 = ct{533};
t4339 = ct{534};
t4341 = ct{535};
t4342 = ct{536};
t4343 = ct{537};
t4346 = ct{538};
t4352 = ct{539};
t4359 = ct{540};
t4371 = ct{541};
t4372 = ct{542};
t4373 = ct{543};
t4375 = ct{544};
t4413 = ct{545};
t4415 = ct{546};
t4416 = ct{547};
t4417 = ct{548};
t4458 = ct{549};
t4459 = ct{550};
t4461 = ct{551};
t4464 = ct{552};
t4468 = ct{553};
t4470 = ct{554};
t4476 = ct{555};
t4486 = ct{556};
t4488 = ct{557};
t4489 = ct{558};
t4493 = ct{559};
t4494 = ct{560};
t4495 = ct{561};
t4501 = ct{562};
t4502 = ct{563};
t4504 = ct{564};
t4515 = ct{565};
t4518 = ct{566};
t4520 = ct{567};
t4522 = ct{568};
t4537 = ct{569};
t4545 = ct{570};
t4553 = ct{571};
t4559 = ct{572};
t4562 = ct{573};
t4563 = ct{574};
t4567 = ct{575};
t4570 = ct{576};
t4573 = ct{577};
t4576 = ct{578};
t4577 = ct{579};
t4582 = ct{580};
t4583 = ct{581};
t4594 = ct{582};
t46 = ct{583};
t4603 = ct{584};
t4604 = ct{585};
t4606 = ct{586};
t4615 = ct{587};
t4617 = ct{588};
t4618 = ct{589};
t4619 = ct{590};
t4623 = ct{591};
t4634 = ct{592};
t4635 = ct{593};
t4639 = ct{594};
t4644 = ct{595};
t4645 = ct{596};
t4651 = ct{597};
t4652 = ct{598};
t4658 = ct{599};
t4663 = ct{600};
t4665 = ct{601};
t4673 = ct{602};
t4675 = ct{603};
t4676 = ct{604};
t4677 = ct{605};
t4678 = ct{606};
t4680 = ct{607};
t4683 = ct{608};
t47 = ct{609};
t4703 = ct{610};
t4704 = ct{611};
t4705 = ct{612};
t4708 = ct{613};
t4709 = ct{614};
t4713 = ct{615};
t4716 = ct{616};
t4719 = ct{617};
t4722 = ct{618};
t4724 = ct{619};
t4725 = ct{620};
t4728 = ct{621};
t4730 = ct{622};
t4741 = ct{623};
t4744 = ct{624};
t4746 = ct{625};
t4751 = ct{626};
t4757 = ct{627};
t4760 = ct{628};
t4761 = ct{629};
t4762 = ct{630};
t4763 = ct{631};
t4795 = ct{632};
t4799 = ct{633};
t4801 = ct{634};
t4808 = ct{635};
t4809 = ct{636};
t4814 = ct{637};
t4823 = ct{638};
t4828 = ct{639};
t4833 = ct{640};
t4835 = ct{641};
t4838 = ct{642};
t4843 = ct{643};
t4844 = ct{644};
t4846 = ct{645};
t4847 = ct{646};
t4850 = ct{647};
t4853 = ct{648};
t4863 = ct{649};
t4867 = ct{650};
t4872 = ct{651};
t4874 = ct{652};
t4876 = ct{653};
t4879 = ct{654};
t4880 = ct{655};
t4887 = ct{656};
t4893 = ct{657};
t4895 = ct{658};
t4896 = ct{659};
t4902 = ct{660};
t4903 = ct{661};
t4904 = ct{662};
t4905 = ct{663};
t4906 = ct{664};
t4911 = ct{665};
t4912 = ct{666};
t4915 = ct{667};
t4920 = ct{668};
t4923 = ct{669};
t4924 = ct{670};
t4925 = ct{671};
t4927 = ct{672};
t4928 = ct{673};
t4950 = ct{674};
t4978 = ct{675};
t4981 = ct{676};
t4982 = ct{677};
t4983 = ct{678};
t4990 = ct{679};
t4995 = ct{680};
t4996 = ct{681};
t4999 = ct{682};
t50 = ct{683};
t5001 = ct{684};
t5003 = ct{685};
t5004 = ct{686};
t5005 = ct{687};
t5007 = ct{688};
t5009 = ct{689};
t5010 = ct{690};
t5011 = ct{691};
t5013 = ct{692};
t5014 = ct{693};
t5016 = ct{694};
t5025 = ct{695};
t5026 = ct{696};
t5027 = ct{697};
t5028 = ct{698};
t5034 = ct{699};
t5035 = ct{700};
t5036 = ct{701};
t5037 = ct{702};
t5038 = ct{703};
t5041 = ct{704};
t5042 = ct{705};
t5043 = ct{706};
t5046 = ct{707};
t5049 = ct{708};
t5063 = ct{709};
t5080 = ct{710};
t5082 = ct{711};
t5083 = ct{712};
t5084 = ct{713};
t5085 = ct{714};
t5086 = ct{715};
t5087 = ct{716};
t5088 = ct{717};
t5089 = ct{718};
t5090 = ct{719};
t5091 = ct{720};
t5093 = ct{721};
t5096 = ct{722};
t5097 = ct{723};
t5098 = ct{724};
t5103 = ct{725};
t5105 = ct{726};
t5106 = ct{727};
t5108 = ct{728};
t5113 = ct{729};
t5119 = ct{730};
t5126 = ct{731};
t5141 = ct{732};
t5142 = ct{733};
t5153 = ct{734};
t5154 = ct{735};
t5155 = ct{736};
t5161 = ct{737};
t5164 = ct{738};
t5167 = ct{739};
t5169 = ct{740};
t5183 = ct{741};
t5184 = ct{742};
t5185 = ct{743};
t5186 = ct{744};
t5189 = ct{745};
t5190 = ct{746};
t5194 = ct{747};
t5197 = ct{748};
t5198 = ct{749};
t5199 = ct{750};
t5200 = ct{751};
t5201 = ct{752};
t5202 = ct{753};
t5205 = ct{754};
t5213 = ct{755};
t5214 = ct{756};
t5234 = ct{757};
t5236 = ct{758};
t5240 = ct{759};
t5243 = ct{760};
t5246 = ct{761};
t5247 = ct{762};
t5248 = ct{763};
t5249 = ct{764};
t5251 = ct{765};
t5255 = ct{766};
t5256 = ct{767};
t5257 = ct{768};
t5258 = ct{769};
t5259 = ct{770};
t5262 = ct{771};
t5264 = ct{772};
t5265 = ct{773};
t5275 = ct{774};
t5278 = ct{775};
t5279 = ct{776};
t5280 = ct{777};
t5283 = ct{778};
t5286 = ct{779};
t5287 = ct{780};
t5291 = ct{781};
t5296 = ct{782};
t5297 = ct{783};
t5301 = ct{784};
t5302 = ct{785};
t5303 = ct{786};
t5304 = ct{787};
t5305 = ct{788};
t5306 = ct{789};
t5308 = ct{790};
t5309 = ct{791};
t5312 = ct{792};
t5313 = ct{793};
t5317 = ct{794};
t5328 = ct{795};
t5331 = ct{796};
t5332 = ct{797};
t5333 = ct{798};
t5336 = ct{799};
t5337 = ct{800};
t5340 = ct{801};
t5341 = ct{802};
t5343 = ct{803};
t5344 = ct{804};
t5345 = ct{805};
t5346 = ct{806};
t5348 = ct{807};
t5350 = ct{808};
t5352 = ct{809};
t5353 = ct{810};
t5356 = ct{811};
t5358 = ct{812};
t5359 = ct{813};
t5361 = ct{814};
t5362 = ct{815};
t5363 = ct{816};
t5369 = ct{817};
t5370 = ct{818};
t5372 = ct{819};
t5373 = ct{820};
t5374 = ct{821};
t5376 = ct{822};
t5377 = ct{823};
t5381 = ct{824};
t5382 = ct{825};
t5383 = ct{826};
t5384 = ct{827};
t5385 = ct{828};
t5386 = ct{829};
t5387 = ct{830};
t5389 = ct{831};
t5390 = ct{832};
t5391 = ct{833};
t5392 = ct{834};
t5393 = ct{835};
t5395 = ct{836};
t5399 = ct{837};
t5400 = ct{838};
t5401 = ct{839};
t5402 = ct{840};
t5403 = ct{841};
t5404 = ct{842};
t5405 = ct{843};
t5409 = ct{844};
t5410 = ct{845};
t5411 = ct{846};
t5412 = ct{847};
t5413 = ct{848};
t5415 = ct{849};
t5416 = ct{850};
t5417 = ct{851};
t5419 = ct{852};
t5421 = ct{853};
t5422 = ct{854};
t5423 = ct{855};
t5425 = ct{856};
t5428 = ct{857};
t5430 = ct{858};
t5432 = ct{859};
t5433 = ct{860};
t5434 = ct{861};
t5436 = ct{862};
t5437 = ct{863};
t5438 = ct{864};
t5439 = ct{865};
t5449 = ct{866};
t5451 = ct{867};
t5452 = ct{868};
t5453 = ct{869};
t5454 = ct{870};
t5455 = ct{871};
t5456 = ct{872};
t5457 = ct{873};
t5458 = ct{874};
t5459 = ct{875};
t5460 = ct{876};
t5464 = ct{877};
t5465 = ct{878};
t5466 = ct{879};
t5467 = ct{880};
t5468 = ct{881};
t5480 = ct{882};
t5481 = ct{883};
t5483 = ct{884};
t5486 = ct{885};
t5487 = ct{886};
t5488 = ct{887};
t5489 = ct{888};
t5490 = ct{889};
t5491 = ct{890};
t5492 = ct{891};
t5493 = ct{892};
t5494 = ct{893};
t5495 = ct{894};
t5496 = ct{895};
t5497 = ct{896};
t5499 = ct{897};
t5508 = ct{898};
t5515 = ct{899};
t5523 = ct{900};
t5535 = ct{901};
t5536 = ct{902};
t5537 = ct{903};
t5538 = ct{904};
t5539 = ct{905};
t5542 = ct{906};
t5543 = ct{907};
t5544 = ct{908};
t5545 = ct{909};
t5546 = ct{910};
t5547 = ct{911};
t5548 = ct{912};
t5549 = ct{913};
t5550 = ct{914};
t5551 = ct{915};
t5552 = ct{916};
t5553 = ct{917};
t5554 = ct{918};
t5555 = ct{919};
t5556 = ct{920};
t5557 = ct{921};
t5558 = ct{922};
t5560 = ct{923};
t5563 = ct{924};
t5564 = ct{925};
t5565 = ct{926};
t5567 = ct{927};
t5568 = ct{928};
t5569 = ct{929};
t5570 = ct{930};
t5572 = ct{931};
t5573 = ct{932};
t5574 = ct{933};
t5575 = ct{934};
t5576 = ct{935};
t5577 = ct{936};
t5578 = ct{937};
t5579 = ct{938};
t5580 = ct{939};
t5581 = ct{940};
t5582 = ct{941};
t5583 = ct{942};
t5584 = ct{943};
t5585 = ct{944};
t5586 = ct{945};
t5587 = ct{946};
t5588 = ct{947};
t5589 = ct{948};
t5590 = ct{949};
t5591 = ct{950};
t5592 = ct{951};
t5593 = ct{952};
t5594 = ct{953};
t5598 = ct{954};
t5599 = ct{955};
t56 = ct{956};
t5603 = ct{957};
t5604 = ct{958};
t5605 = ct{959};
t5607 = ct{960};
t5611 = ct{961};
t5612 = ct{962};
t5613 = ct{963};
t5614 = ct{964};
t5615 = ct{965};
t5616 = ct{966};
t5618 = ct{967};
t5622 = ct{968};
t5624 = ct{969};
t5626 = ct{970};
t5628 = ct{971};
t5631 = ct{972};
t5632 = ct{973};
t5636 = ct{974};
t5637 = ct{975};
t5638 = ct{976};
t5641 = ct{977};
t5642 = ct{978};
t5643 = ct{979};
t5645 = ct{980};
t5646 = ct{981};
t5647 = ct{982};
t5649 = ct{983};
t5650 = ct{984};
t5651 = ct{985};
t5652 = ct{986};
t5653 = ct{987};
t5655 = ct{988};
t5658 = ct{989};
t5659 = ct{990};
t5669 = ct{991};
t5670 = ct{992};
t5671 = ct{993};
t5672 = ct{994};
t5673 = ct{995};
t5675 = ct{996};
t5677 = ct{997};
t5678 = ct{998};
t5679 = ct{999};
t5680 = ct{1000};
t5681 = ct{1001};
t5682 = ct{1002};
t5683 = ct{1003};
t5684 = ct{1004};
t5685 = ct{1005};
t5686 = ct{1006};
t5687 = ct{1007};
t5688 = ct{1008};
t5689 = ct{1009};
t5690 = ct{1010};
t5691 = ct{1011};
t5694 = ct{1012};
t5695 = ct{1013};
t5698 = ct{1014};
t5699 = ct{1015};
t5709 = ct{1016};
t5710 = ct{1017};
t5711 = ct{1018};
t5712 = ct{1019};
t5713 = ct{1020};
t5714 = ct{1021};
t5715 = ct{1022};
t5716 = ct{1023};
t5717 = ct{1024};
t5718 = ct{1025};
t5720 = ct{1026};
t5721 = ct{1027};
t5722 = ct{1028};
t5723 = ct{1029};
t5724 = ct{1030};
t5725 = ct{1031};
t5730 = ct{1032};
t5731 = ct{1033};
t5734 = ct{1034};
t5735 = ct{1035};
t5738 = ct{1036};
t5739 = ct{1037};
t5741 = ct{1038};
t5742 = ct{1039};
t5745 = ct{1040};
t5747 = ct{1041};
t5751 = ct{1042};
t5753 = ct{1043};
t5754 = ct{1044};
t5756 = ct{1045};
t5758 = ct{1046};
t5759 = ct{1047};
t5760 = ct{1048};
t5761 = ct{1049};
t5762 = ct{1050};
t5763 = ct{1051};
t5764 = ct{1052};
t5765 = ct{1053};
t5766 = ct{1054};
t5767 = ct{1055};
t5768 = ct{1056};
t5769 = ct{1057};
t5770 = ct{1058};
t5771 = ct{1059};
t5772 = ct{1060};
t5773 = ct{1061};
t5774 = ct{1062};
t5775 = ct{1063};
t5776 = ct{1064};
t5777 = ct{1065};
t5778 = ct{1066};
t5779 = ct{1067};
t5781 = ct{1068};
t5782 = ct{1069};
t5783 = ct{1070};
t5784 = ct{1071};
t5787 = ct{1072};
t5788 = ct{1073};
t5790 = ct{1074};
t5791 = ct{1075};
t5792 = ct{1076};
t5793 = ct{1077};
t5794 = ct{1078};
t5795 = ct{1079};
t5796 = ct{1080};
t5798 = ct{1081};
t5799 = ct{1082};
t5801 = ct{1083};
t5802 = ct{1084};
t5804 = ct{1085};
t5809 = ct{1086};
t5810 = ct{1087};
t5813 = ct{1088};
t5814 = ct{1089};
t5816 = ct{1090};
t5817 = ct{1091};
t5819 = ct{1092};
t5820 = ct{1093};
t5821 = ct{1094};
t5825 = ct{1095};
t5826 = ct{1096};
t5827 = ct{1097};
t5828 = ct{1098};
t5829 = ct{1099};
t5831 = ct{1100};
t5832 = ct{1101};
t5833 = ct{1102};
t5835 = ct{1103};
t5836 = ct{1104};
t5837 = ct{1105};
t5838 = ct{1106};
t5839 = ct{1107};
t5840 = ct{1108};
t5842 = ct{1109};
t5844 = ct{1110};
t5845 = ct{1111};
t5846 = ct{1112};
t5849 = ct{1113};
t5851 = ct{1114};
t5852 = ct{1115};
t5853 = ct{1116};
t5855 = ct{1117};
t5856 = ct{1118};
t5857 = ct{1119};
t5858 = ct{1120};
t5859 = ct{1121};
t5860 = ct{1122};
t5864 = ct{1123};
t5867 = ct{1124};
t5868 = ct{1125};
t5869 = ct{1126};
t5870 = ct{1127};
t5871 = ct{1128};
t5872 = ct{1129};
t5874 = ct{1130};
t5875 = ct{1131};
t5876 = ct{1132};
t5877 = ct{1133};
t5878 = ct{1134};
t5879 = ct{1135};
t5880 = ct{1136};
t5881 = ct{1137};
t5882 = ct{1138};
t5884 = ct{1139};
t5886 = ct{1140};
t5888 = ct{1141};
t5890 = ct{1142};
t5891 = ct{1143};
t5892 = ct{1144};
t5893 = ct{1145};
t5894 = ct{1146};
t5896 = ct{1147};
t5897 = ct{1148};
t5898 = ct{1149};
t5899 = ct{1150};
t5900 = ct{1151};
t5901 = ct{1152};
t5902 = ct{1153};
t5904 = ct{1154};
t5905 = ct{1155};
t5906 = ct{1156};
t5907 = ct{1157};
t5908 = ct{1158};
t5909 = ct{1159};
t5910 = ct{1160};
t5911 = ct{1161};
t5912 = ct{1162};
t5913 = ct{1163};
t5914 = ct{1164};
t5915 = ct{1165};
t5916 = ct{1166};
t5917 = ct{1167};
t5918 = ct{1168};
t5919 = ct{1169};
t5920 = ct{1170};
t5922 = ct{1171};
t5923 = ct{1172};
t5924 = ct{1173};
t5925 = ct{1174};
t5926 = ct{1175};
t5927 = ct{1176};
t5928 = ct{1177};
t5930 = ct{1178};
t5931 = ct{1179};
t5933 = ct{1180};
t5934 = ct{1181};
t5935 = ct{1182};
t5937 = ct{1183};
t5938 = ct{1184};
t5939 = ct{1185};
t5941 = ct{1186};
t5942 = ct{1187};
t5943 = ct{1188};
t5945 = ct{1189};
t5946 = ct{1190};
t5947 = ct{1191};
t5948 = ct{1192};
t5949 = ct{1193};
t5950 = ct{1194};
t5951 = ct{1195};
t5954 = ct{1196};
t5955 = ct{1197};
t5956 = ct{1198};
t5957 = ct{1199};
t5958 = ct{1200};
t5959 = ct{1201};
t5960 = ct{1202};
t5962 = ct{1203};
t5963 = ct{1204};
t5965 = ct{1205};
t5966 = ct{1206};
t5967 = ct{1207};
t5968 = ct{1208};
t5969 = ct{1209};
t5970 = ct{1210};
t5973 = ct{1211};
t5974 = ct{1212};
t5975 = ct{1213};
t5976 = ct{1214};
t5977 = ct{1215};
t5978 = ct{1216};
t5979 = ct{1217};
t5980 = ct{1218};
t5981 = ct{1219};
t5982 = ct{1220};
t5984 = ct{1221};
t5985 = ct{1222};
t5986 = ct{1223};
t5988 = ct{1224};
t5990 = ct{1225};
t5992 = ct{1226};
t5993 = ct{1227};
t5994 = ct{1228};
t5995 = ct{1229};
t5997 = ct{1230};
t5999 = ct{1231};
t60 = ct{1232};
t6000 = ct{1233};
t6001 = ct{1234};
t6004 = ct{1235};
t6005 = ct{1236};
t6006 = ct{1237};
t6007 = ct{1238};
t6008 = ct{1239};
t6009 = ct{1240};
t6010 = ct{1241};
t6011 = ct{1242};
t6013 = ct{1243};
t6014 = ct{1244};
t6015 = ct{1245};
t6017 = ct{1246};
t6018 = ct{1247};
t6019 = ct{1248};
t6020 = ct{1249};
t6021 = ct{1250};
t6022 = ct{1251};
t6023 = ct{1252};
t6024 = ct{1253};
t6026 = ct{1254};
t6027 = ct{1255};
t6028 = ct{1256};
t6029 = ct{1257};
t6031 = ct{1258};
t6032 = ct{1259};
t6037 = ct{1260};
t6039 = ct{1261};
t6041 = ct{1262};
t6043 = ct{1263};
t6045 = ct{1264};
t6046 = ct{1265};
t6047 = ct{1266};
t6050 = ct{1267};
t6052 = ct{1268};
t6053 = ct{1269};
t6054 = ct{1270};
t6055 = ct{1271};
t6058 = ct{1272};
t6059 = ct{1273};
t6060 = ct{1274};
t6062 = ct{1275};
t6064 = ct{1276};
t6065 = ct{1277};
t6066 = ct{1278};
t6067 = ct{1279};
t6074 = ct{1280};
t6076 = ct{1281};
t6079 = ct{1282};
t6080 = ct{1283};
t6081 = ct{1284};
t6082 = ct{1285};
t6083 = ct{1286};
t6084 = ct{1287};
t6085 = ct{1288};
t6086 = ct{1289};
t6087 = ct{1290};
t6088 = ct{1291};
t6091 = ct{1292};
t6093 = ct{1293};
t6094 = ct{1294};
t6095 = ct{1295};
t6096 = ct{1296};
t6098 = ct{1297};
t6100 = ct{1298};
t6102 = ct{1299};
t6106 = ct{1300};
t6107 = ct{1301};
t6109 = ct{1302};
t6110 = ct{1303};
t6111 = ct{1304};
t6112 = ct{1305};
t6115 = ct{1306};
t6116 = ct{1307};
t6119 = ct{1308};
t6120 = ct{1309};
t6121 = ct{1310};
t6125 = ct{1311};
t6129 = ct{1312};
t6131 = ct{1313};
t6133 = ct{1314};
t6134 = ct{1315};
t6135 = ct{1316};
t6136 = ct{1317};
t6137 = ct{1318};
t6138 = ct{1319};
t6139 = ct{1320};
t6140 = ct{1321};
t6141 = ct{1322};
t6143 = ct{1323};
t6144 = ct{1324};
t6145 = ct{1325};
t6149 = ct{1326};
t6150 = ct{1327};
t6151 = ct{1328};
t6152 = ct{1329};
t6153 = ct{1330};
t6156 = ct{1331};
t6159 = ct{1332};
t6160 = ct{1333};
t6162 = ct{1334};
t6164 = ct{1335};
t6166 = ct{1336};
t6168 = ct{1337};
t6169 = ct{1338};
t6170 = ct{1339};
t6171 = ct{1340};
t6172 = ct{1341};
t6173 = ct{1342};
t6174 = ct{1343};
t6175 = ct{1344};
t6177 = ct{1345};
t6178 = ct{1346};
t6180 = ct{1347};
t6181 = ct{1348};
t6183 = ct{1349};
t6184 = ct{1350};
t6185 = ct{1351};
t6186 = ct{1352};
t6187 = ct{1353};
t6188 = ct{1354};
t6189 = ct{1355};
t6190 = ct{1356};
t6191 = ct{1357};
t6192 = ct{1358};
t6193 = ct{1359};
t6194 = ct{1360};
t6195 = ct{1361};
t6196 = ct{1362};
t6198 = ct{1363};
t6200 = ct{1364};
t6201 = ct{1365};
t6202 = ct{1366};
t6205 = ct{1367};
t6206 = ct{1368};
t6207 = ct{1369};
t6208 = ct{1370};
t6209 = ct{1371};
t6210 = ct{1372};
t6217 = ct{1373};
t6218 = ct{1374};
t6219 = ct{1375};
t6223 = ct{1376};
t6225 = ct{1377};
t6226 = ct{1378};
t6227 = ct{1379};
t6228 = ct{1380};
t6231 = ct{1381};
t6232 = ct{1382};
t6233 = ct{1383};
t6234 = ct{1384};
t6237 = ct{1385};
t6238 = ct{1386};
t6239 = ct{1387};
t6240 = ct{1388};
t6241 = ct{1389};
t6244 = ct{1390};
t6250 = ct{1391};
t6251 = ct{1392};
t6252 = ct{1393};
t6253 = ct{1394};
t6255 = ct{1395};
t6256 = ct{1396};
t6257 = ct{1397};
t6262 = ct{1398};
t6263 = ct{1399};
t6265 = ct{1400};
t6266 = ct{1401};
t6269 = ct{1402};
t6270 = ct{1403};
t6271 = ct{1404};
t6272 = ct{1405};
t6275 = ct{1406};
t6281 = ct{1407};
t6282 = ct{1408};
t6283 = ct{1409};
t6284 = ct{1410};
t6287 = ct{1411};
t6289 = ct{1412};
t6290 = ct{1413};
t6291 = ct{1414};
t6292 = ct{1415};
t6293 = ct{1416};
t6295 = ct{1417};
t6297 = ct{1418};
t6298 = ct{1419};
t6299 = ct{1420};
t6302 = ct{1421};
t6303 = ct{1422};
t6304 = ct{1423};
t6306 = ct{1424};
t6307 = ct{1425};
t6308 = ct{1426};
t6309 = ct{1427};
t6311 = ct{1428};
t6312 = ct{1429};
t6313 = ct{1430};
t6314 = ct{1431};
t6316 = ct{1432};
t6317 = ct{1433};
t6319 = ct{1434};
t6322 = ct{1435};
t6323 = ct{1436};
t6324 = ct{1437};
t6326 = ct{1438};
t6327 = ct{1439};
t6328 = ct{1440};
t6329 = ct{1441};
t6330 = ct{1442};
t6332 = ct{1443};
t6333 = ct{1444};
t6334 = ct{1445};
t6337 = ct{1446};
t6338 = ct{1447};
t6339 = ct{1448};
t6341 = ct{1449};
t6342 = ct{1450};
t6343 = ct{1451};
t6345 = ct{1452};
t6346 = ct{1453};
t6347 = ct{1454};
t6348 = ct{1455};
t6354 = ct{1456};
t6355 = ct{1457};
t6357 = ct{1458};
t6358 = ct{1459};
t6360 = ct{1460};
t6361 = ct{1461};
t6362 = ct{1462};
t6363 = ct{1463};
t6364 = ct{1464};
t6365 = ct{1465};
t6366 = ct{1466};
t6367 = ct{1467};
t6368 = ct{1468};
t6369 = ct{1469};
t6371 = ct{1470};
t6372 = ct{1471};
t6373 = ct{1472};
t6375 = ct{1473};
t6376 = ct{1474};
t6377 = ct{1475};
t6379 = ct{1476};
t6384 = ct{1477};
t6391 = ct{1478};
t6392 = ct{1479};
t6393 = ct{1480};
t6394 = ct{1481};
t6396 = ct{1482};
t6398 = ct{1483};
t6402 = ct{1484};
t6404 = ct{1485};
t6405 = ct{1486};
t6407 = ct{1487};
t6408 = ct{1488};
t6409 = ct{1489};
t6410 = ct{1490};
t6412 = ct{1491};
t6413 = ct{1492};
t6415 = ct{1493};
t6417 = ct{1494};
t6418 = ct{1495};
t6419 = ct{1496};
t642 = ct{1497};
t6420 = ct{1498};
t6421 = ct{1499};
t6423 = ct{1500};
t6425 = ct{1501};
t6426 = ct{1502};
t6427 = ct{1503};
t6428 = ct{1504};
t6429 = ct{1505};
t643 = ct{1506};
t6431 = ct{1507};
t6432 = ct{1508};
t6433 = ct{1509};
t6434 = ct{1510};
t6435 = ct{1511};
t6436 = ct{1512};
t6438 = ct{1513};
t6439 = ct{1514};
t6440 = ct{1515};
t6441 = ct{1516};
t6442 = ct{1517};
t6443 = ct{1518};
t6444 = ct{1519};
t6445 = ct{1520};
t6446 = ct{1521};
t6447 = ct{1522};
t6449 = ct{1523};
t6452 = ct{1524};
t6455 = ct{1525};
t6457 = ct{1526};
t6458 = ct{1527};
t6459 = ct{1528};
t6460 = ct{1529};
t6461 = ct{1530};
t6462 = ct{1531};
t6463 = ct{1532};
t6464 = ct{1533};
t6465 = ct{1534};
t6466 = ct{1535};
t6467 = ct{1536};
t6468 = ct{1537};
t6469 = ct{1538};
t6471 = ct{1539};
t6472 = ct{1540};
t6473 = ct{1541};
t6474 = ct{1542};
t6475 = ct{1543};
t6476 = ct{1544};
t6477 = ct{1545};
t6478 = ct{1546};
t6480 = ct{1547};
t6481 = ct{1548};
t6482 = ct{1549};
t6483 = ct{1550};
t6484 = ct{1551};
t649 = ct{1552};
t6490 = ct{1553};
t6491 = ct{1554};
t6493 = ct{1555};
t6496 = ct{1556};
t6498 = ct{1557};
t6499 = ct{1558};
t6500 = ct{1559};
t6501 = ct{1560};
t6502 = ct{1561};
t6503 = ct{1562};
t6504 = ct{1563};
t6506 = ct{1564};
t6508 = ct{1565};
t6509 = ct{1566};
t6510 = ct{1567};
t6511 = ct{1568};
t6512 = ct{1569};
t6513 = ct{1570};
t6514 = ct{1571};
t6515 = ct{1572};
t6517 = ct{1573};
t6518 = ct{1574};
t6519 = ct{1575};
t6520 = ct{1576};
t6521 = ct{1577};
t6522 = ct{1578};
t6523 = ct{1579};
t6524 = ct{1580};
t6525 = ct{1581};
t6526 = ct{1582};
t6527 = ct{1583};
t6528 = ct{1584};
t6529 = ct{1585};
t6531 = ct{1586};
t6534 = ct{1587};
t6535 = ct{1588};
t6536 = ct{1589};
t6537 = ct{1590};
t6538 = ct{1591};
t6539 = ct{1592};
t6540 = ct{1593};
t6542 = ct{1594};
t6544 = ct{1595};
t6545 = ct{1596};
t6546 = ct{1597};
t6547 = ct{1598};
t6548 = ct{1599};
t6549 = ct{1600};
t6550 = ct{1601};
t6551 = ct{1602};
t6552 = ct{1603};
t6553 = ct{1604};
t6559 = ct{1605};
t6560 = ct{1606};
t6561 = ct{1607};
t6562 = ct{1608};
t6564 = ct{1609};
t6565 = ct{1610};
t6567 = ct{1611};
t6568 = ct{1612};
t6569 = ct{1613};
t6570 = ct{1614};
t6571 = ct{1615};
t6572 = ct{1616};
t6573 = ct{1617};
t6574 = ct{1618};
t6575 = ct{1619};
t6576 = ct{1620};
t6579 = ct{1621};
t6580 = ct{1622};
t6582 = ct{1623};
t6583 = ct{1624};
t6584 = ct{1625};
t6585 = ct{1626};
t6588 = ct{1627};
t6589 = ct{1628};
t6591 = ct{1629};
t6592 = ct{1630};
t6593 = ct{1631};
t6594 = ct{1632};
t6595 = ct{1633};
t6596 = ct{1634};
t6597 = ct{1635};
t6598 = ct{1636};
t6599 = ct{1637};
t6600 = ct{1638};
t6601 = ct{1639};
t6602 = ct{1640};
t6605 = ct{1641};
t6606 = ct{1642};
t6607 = ct{1643};
t6608 = ct{1644};
t6609 = ct{1645};
t6610 = ct{1646};
t6616 = ct{1647};
t6617 = ct{1648};
t6622 = ct{1649};
t6623 = ct{1650};
t6624 = ct{1651};
t6625 = ct{1652};
t6626 = ct{1653};
t6627 = ct{1654};
t6629 = ct{1655};
t6631 = ct{1656};
t6633 = ct{1657};
t6636 = ct{1658};
t6638 = ct{1659};
t6645 = ct{1660};
t6646 = ct{1661};
t6647 = ct{1662};
t6648 = ct{1663};
t6649 = ct{1664};
t6651 = ct{1665};
t6652 = ct{1666};
t6654 = ct{1667};
t6656 = ct{1668};
t6657 = ct{1669};
t6658 = ct{1670};
t6660 = ct{1671};
t6663 = ct{1672};
t6664 = ct{1673};
t6665 = ct{1674};
t667 = ct{1675};
t6670 = ct{1676};
t6671 = ct{1677};
t6672 = ct{1678};
t6673 = ct{1679};
t6674 = ct{1680};
t6675 = ct{1681};
t6678 = ct{1682};
t6679 = ct{1683};
t6680 = ct{1684};
t6681 = ct{1685};
t6682 = ct{1686};
t6683 = ct{1687};
t6684 = ct{1688};
t6685 = ct{1689};
t6686 = ct{1690};
t6687 = ct{1691};
t6688 = ct{1692};
t6690 = ct{1693};
t6691 = ct{1694};
t6692 = ct{1695};
t6693 = ct{1696};
t6696 = ct{1697};
t6699 = ct{1698};
t670 = ct{1699};
t6700 = ct{1700};
t6702 = ct{1701};
t6704 = ct{1702};
t6705 = ct{1703};
t6706 = ct{1704};
t6708 = ct{1705};
t6716 = ct{1706};
t6717 = ct{1707};
t6719 = ct{1708};
t6720 = ct{1709};
t6722 = ct{1710};
t6723 = ct{1711};
t6724 = ct{1712};
t6725 = ct{1713};
t6731 = ct{1714};
t6732 = ct{1715};
t6733 = ct{1716};
t6734 = ct{1717};
t674 = ct{1718};
t6740 = ct{1719};
t6741 = ct{1720};
t6745 = ct{1721};
t6747 = ct{1722};
t6750 = ct{1723};
t6751 = ct{1724};
t6752 = ct{1725};
t6756 = ct{1726};
t6758 = ct{1727};
t6761 = ct{1728};
t6762 = ct{1729};
t6765 = ct{1730};
t6766 = ct{1731};
t6767 = ct{1732};
t6772 = ct{1733};
t6773 = ct{1734};
t6774 = ct{1735};
t6775 = ct{1736};
t6776 = ct{1737};
t6777 = ct{1738};
t6788 = ct{1739};
t6789 = ct{1740};
t6791 = ct{1741};
t6794 = ct{1742};
t6801 = ct{1743};
t6802 = ct{1744};
t6804 = ct{1745};
t6806 = ct{1746};
t6807 = ct{1747};
t6808 = ct{1748};
t6810 = ct{1749};
t6812 = ct{1750};
t6813 = ct{1751};
t6814 = ct{1752};
t6815 = ct{1753};
t6816 = ct{1754};
t6818 = ct{1755};
t6819 = ct{1756};
t6831 = ct{1757};
t6833 = ct{1758};
t6836 = ct{1759};
t6837 = ct{1760};
t6839 = ct{1761};
t684 = ct{1762};
t6840 = ct{1763};
t6842 = ct{1764};
t6845 = ct{1765};
t6846 = ct{1766};
t6847 = ct{1767};
t685 = ct{1768};
t6850 = ct{1769};
t6851 = ct{1770};
t6852 = ct{1771};
t6854 = ct{1772};
t6858 = ct{1773};
t6859 = ct{1774};
t686 = ct{1775};
t6860 = ct{1776};
t6861 = ct{1777};
t6862 = ct{1778};
t6863 = ct{1779};
t6864 = ct{1780};
t6865 = ct{1781};
t6868 = ct{1782};
t687 = ct{1783};
t6870 = ct{1784};
t6871 = ct{1785};
t6872 = ct{1786};
t6873 = ct{1787};
t6874 = ct{1788};
t6875 = ct{1789};
t6876 = ct{1790};
t6877 = ct{1791};
t6878 = ct{1792};
t6879 = ct{1793};
t6880 = ct{1794};
t6881 = ct{1795};
t6882 = ct{1796};
t6883 = ct{1797};
t6884 = ct{1798};
t6886 = ct{1799};
t6887 = ct{1800};
t6888 = ct{1801};
t6890 = ct{1802};
t6891 = ct{1803};
t6892 = ct{1804};
t6893 = ct{1805};
t6894 = ct{1806};
t6897 = ct{1807};
t6900 = ct{1808};
t6902 = ct{1809};
t6903 = ct{1810};
t6904 = ct{1811};
t6905 = ct{1812};
t6906 = ct{1813};
t6907 = ct{1814};
t6909 = ct{1815};
t6910 = ct{1816};
t6911 = ct{1817};
t6913 = ct{1818};
t6916 = ct{1819};
t6918 = ct{1820};
t6919 = ct{1821};
t6920 = ct{1822};
t6923 = ct{1823};
t6924 = ct{1824};
t6925 = ct{1825};
t6926 = ct{1826};
t6927 = ct{1827};
t6928 = ct{1828};
t6929 = ct{1829};
t6930 = ct{1830};
t6932 = ct{1831};
t6933 = ct{1832};
t6934 = ct{1833};
t6935 = ct{1834};
t6936 = ct{1835};
t6938 = ct{1836};
t6939 = ct{1837};
t6940 = ct{1838};
t6941 = ct{1839};
t6942 = ct{1840};
t6944 = ct{1841};
t6945 = ct{1842};
t6946 = ct{1843};
t6948 = ct{1844};
t6949 = ct{1845};
t6951 = ct{1846};
t6952 = ct{1847};
t6953 = ct{1848};
t6954 = ct{1849};
t6956 = ct{1850};
t6957 = ct{1851};
t6958 = ct{1852};
t6962 = ct{1853};
t6964 = ct{1854};
t6965 = ct{1855};
t6966 = ct{1856};
t6968 = ct{1857};
t6971 = ct{1858};
t6972 = ct{1859};
t6974 = ct{1860};
t6976 = ct{1861};
t6978 = ct{1862};
t6979 = ct{1863};
t6980 = ct{1864};
t6983 = ct{1865};
t6984 = ct{1866};
t6985 = ct{1867};
t6987 = ct{1868};
t6992 = ct{1869};
t6993 = ct{1870};
t6994 = ct{1871};
t6995 = ct{1872};
t6997 = ct{1873};
t6998 = ct{1874};
t7000 = ct{1875};
t7003 = ct{1876};
t7005 = ct{1877};
t7007 = ct{1878};
t7009 = ct{1879};
t7010 = ct{1880};
t7011 = ct{1881};
t7014 = ct{1882};
t7016 = ct{1883};
t7019 = ct{1884};
t7020 = ct{1885};
t7021 = ct{1886};
t7022 = ct{1887};
t7023 = ct{1888};
t7028 = ct{1889};
t7029 = ct{1890};
t7030 = ct{1891};
t7032 = ct{1892};
t7033 = ct{1893};
t7035 = ct{1894};
t7040 = ct{1895};
t7041 = ct{1896};
t7042 = ct{1897};
t7043 = ct{1898};
t7044 = ct{1899};
t7045 = ct{1900};
t7046 = ct{1901};
t7048 = ct{1902};
t7050 = ct{1903};
t7051 = ct{1904};
t7054 = ct{1905};
t7055 = ct{1906};
t7057 = ct{1907};
t7059 = ct{1908};
t7060 = ct{1909};
t7061 = ct{1910};
t7063 = ct{1911};
t7064 = ct{1912};
t7067 = ct{1913};
t7068 = ct{1914};
t7069 = ct{1915};
t707 = ct{1916};
t7071 = ct{1917};
t7073 = ct{1918};
t7074 = ct{1919};
t7075 = ct{1920};
t7079 = ct{1921};
t708 = ct{1922};
t7080 = ct{1923};
t7083 = ct{1924};
t7086 = ct{1925};
t7088 = ct{1926};
t7090 = ct{1927};
t7092 = ct{1928};
t7095 = ct{1929};
t7098 = ct{1930};
t710 = ct{1931};
t7100 = ct{1932};
t7101 = ct{1933};
t7104 = ct{1934};
t7105 = ct{1935};
t7106 = ct{1936};
t7107 = ct{1937};
t7111 = ct{1938};
t7118 = ct{1939};
t7119 = ct{1940};
t7120 = ct{1941};
t7121 = ct{1942};
t7122 = ct{1943};
t7123 = ct{1944};
t7124 = ct{1945};
t7126 = ct{1946};
t7127 = ct{1947};
t7128 = ct{1948};
t7129 = ct{1949};
t7130 = ct{1950};
t7133 = ct{1951};
t7134 = ct{1952};
t7138 = ct{1953};
t7148 = ct{1954};
t7150 = ct{1955};
t7159 = ct{1956};
t7160 = ct{1957};
t7162 = ct{1958};
t7164 = ct{1959};
t7166 = ct{1960};
t7168 = ct{1961};
t7170 = ct{1962};
t7171 = ct{1963};
t7181 = ct{1964};
t7184 = ct{1965};
t7188 = ct{1966};
t7191 = ct{1967};
t7195 = ct{1968};
t7196 = ct{1969};
t7197 = ct{1970};
t7199 = ct{1971};
t7203 = ct{1972};
t7204 = ct{1973};
t7205 = ct{1974};
t7208 = ct{1975};
t7209 = ct{1976};
t721 = ct{1977};
t7210 = ct{1978};
t7211 = ct{1979};
t7213 = ct{1980};
t7214 = ct{1981};
t722 = ct{1982};
t7224 = ct{1983};
t7226 = ct{1984};
t7232 = ct{1985};
t7233 = ct{1986};
t724 = ct{1987};
t7246 = ct{1988};
t7253 = ct{1989};
t7256 = ct{1990};
t7260 = ct{1991};
t7265 = ct{1992};
t7271 = ct{1993};
t7277 = ct{1994};
t7278 = ct{1995};
t7279 = ct{1996};
t7281 = ct{1997};
t7283 = ct{1998};
t7286 = ct{1999};
t7287 = ct{2000};
t7291 = ct{2001};
t7292 = ct{2002};
t7294 = ct{2003};
t7297 = ct{2004};
t7298 = ct{2005};
t7300 = ct{2006};
t7301 = ct{2007};
t7304 = ct{2008};
t7307 = ct{2009};
t7308 = ct{2010};
t7309 = ct{2011};
t7310 = ct{2012};
t7311 = ct{2013};
t7315 = ct{2014};
t7319 = ct{2015};
t7322 = ct{2016};
t7323 = ct{2017};
t7335 = ct{2018};
t7337 = ct{2019};
t7339 = ct{2020};
t7340 = ct{2021};
t7344 = ct{2022};
t7345 = ct{2023};
t7348 = ct{2024};
t7349 = ct{2025};
t7358 = ct{2026};
t7360 = ct{2027};
t7364 = ct{2028};
t7365 = ct{2029};
t7366 = ct{2030};
t7376 = ct{2031};
t7378 = ct{2032};
t7379 = ct{2033};
t7380 = ct{2034};
t7385 = ct{2035};
t7387 = ct{2036};
t7388 = ct{2037};
t7389 = ct{2038};
t7394 = ct{2039};
t7396 = ct{2040};
t7397 = ct{2041};
t7401 = ct{2042};
t7402 = ct{2043};
t7403 = ct{2044};
t7404 = ct{2045};
t7405 = ct{2046};
t7406 = ct{2047};
t7407 = ct{2048};
t7410 = ct{2049};
t7411 = ct{2050};
t7412 = ct{2051};
t7413 = ct{2052};
t7416 = ct{2053};
t7417 = ct{2054};
t7422 = ct{2055};
t7423 = ct{2056};
t7424 = ct{2057};
t7425 = ct{2058};
t7432 = ct{2059};
t7433 = ct{2060};
t7436 = ct{2061};
t7458 = ct{2062};
t7459 = ct{2063};
t7462 = ct{2064};
t7471 = ct{2065};
t7473 = ct{2066};
t7477 = ct{2067};
t7478 = ct{2068};
t7479 = ct{2069};
t7482 = ct{2070};
t7483 = ct{2071};
t7484 = ct{2072};
t7485 = ct{2073};
t749 = ct{2074};
t7501 = ct{2075};
t7514 = ct{2076};
t7531 = ct{2077};
t7532 = ct{2078};
t7534 = ct{2079};
t7535 = ct{2080};
t7538 = ct{2081};
t7553 = ct{2082};
t7554 = ct{2083};
t7555 = ct{2084};
t7556 = ct{2085};
t7560 = ct{2086};
t7561 = ct{2087};
t7562 = ct{2088};
t7571 = ct{2089};
t7572 = ct{2090};
t7573 = ct{2091};
t7574 = ct{2092};
t7592 = ct{2093};
t7595 = ct{2094};
t7612 = ct{2095};
t7614 = ct{2096};
t762 = ct{2097};
t7622 = ct{2098};
t7623 = ct{2099};
t7624 = ct{2100};
t7625 = ct{2101};
t7626 = ct{2102};
t7627 = ct{2103};
t7641 = ct{2104};
t7643 = ct{2105};
t7644 = ct{2106};
t7658 = ct{2107};
t7659 = ct{2108};
t768 = ct{2109};
t7686 = ct{2110};
t7692 = ct{2111};
t7715 = ct{2112};
t7737 = ct{2113};
t777 = ct{2114};
t7784 = ct{2115};
t7789 = ct{2116};
t7790 = ct{2117};
t7804 = ct{2118};
t7805 = ct{2119};
t7827 = ct{2120};
t7828 = ct{2121};
t7839 = ct{2122};
t7841 = ct{2123};
t7919 = ct{2124};
t792 = ct{2125};
t7920 = ct{2126};
t7922 = ct{2127};
t793 = ct{2128};
t7938 = ct{2129};
t8 = ct{2130};
t801 = ct{2131};
t802 = ct{2132};
t808 = ct{2133};
t813 = ct{2134};
t819 = ct{2135};
t821 = ct{2136};
t850 = ct{2137};
t855 = ct{2138};
t874 = ct{2139};
t878 = ct{2140};
t9 = ct{2141};
t941 = ct{2142};
t948 = ct{2143};
t951 = ct{2144};
t7140 = t6647.*(t3566.*1.33637554986e-4+t4157-t4158+t28.*(t1896-t3239).*7.26350557185e-5).*(-1.0./2.0);
t7144 = t6699.*(t4893-t28.*(t1005+t20.*(t1941-t3315+t39.*t1022.*(t855-t878).*2.196325630278387e-1)));
t7145 = t5348.*t6696;
t7146 = t5350.*t6696;
t7147 = -t6699.*(t4171-t4896);
t7149 = t6682.*(-t4045+t4049+t12.*(t1861-t3221).*1.838876e-2+t17.*(t1861-t3221).*9.99471e-3).*(-1.0./2.0);
t7182 = t4573.*t6992;
t7183 = t4573.*t6993;
t7185 = t4577.*t6992;
t7187 = t4577.*t6993;
t7189 = t4604.*t6992;
t7190 = t4604.*t6993;
t7192 = -t6992.*(t3563-t4051);
t7193 = -t6993.*(t3563-t4051);
t7194 = t6992.*(t3563-t4051);
t7215 = (t5790.*t6647)./2.0;
t7217 = (t5767.*t6682)./2.0;
t7219 = (t5838.*t6647)./2.0;
t7221 = (t5810.*t6682)./2.0;
t7227 = t6647.*(t4673+t2363.*(t3566.*1.838876e-2+t4109-t4110+t28.*(t1896-t3239).*9.99471e-3).*7.26735e-3).*(-1.0./2.0);
t7228 = (t6647.*(t4673+t2363.*(t3566.*1.838876e-2+t4109-t4110+t28.*(t1896-t3239).*9.99471e-3).*7.26735e-3))./2.0;
t7229 = (t5859.*t6652)./2.0;
t7230 = (t5860.*t6652)./2.0;
t7234 = (t5958.*t6588)./2.0;
t7235 = (t5962.*t6588)./2.0;
t7236 = t6682.*(t5413+t4146.*(t1861-t3221)).*(-1.0./2.0);
t7237 = (t6682.*(t5413+t4146.*(t1861-t3221)))./2.0;
t7238 = t6993.*(t4893-t28.*(t1005+t20.*(t1941-t3315+t39.*t1022.*(t855-t878).*2.196325630278387e-1)));
t7239 = t5348.*t6992;
t7240 = t5350.*t6992;
t7241 = -t6993.*(t4171-t4896);
t7243 = (t5856.*t6682)./2.0;
t7247 = (t5859.*t6682)./2.0;
t7255 = (t5911.*t6647)./2.0;
t7261 = (t5958.*t6647)./2.0;
t7267 = t5859.*(t4853.*(t1896-t3239).*7.26735e-3+t2363.*(t684+t685-t710+t724+t1686-t1690+t1700+t1701+t2371+t2698+t2707-t2716+t2719+t3329-t3337-t3351-t3641+t3643+t3655-t3659+t4114+t4115).*7.26735e-3).*(-1.0./2.0);
t7268 = (t5859.*(t4853.*(t1896-t3239).*7.26735e-3+t2363.*(t684+t685-t710+t724+t1686-t1690+t1700+t1701+t2371+t2698+t2707-t2716+t2719+t3329-t3337-t3351-t3641+t3643+t3655-t3659+t4114+t4115).*7.26735e-3))./2.0;
t7273 = t5958.*(t4814.*(t1861-t3221)+t2297.*(t642+t643-t667+t674+t1587+t1606+t1608+t1609+t2295+t2671+t2683+t2684-t2695+t3279+t3297-t3303+t3597+t3603+t3609-t3614+t4053+t4054)).*(-1.0./2.0);
t7274 = (t5958.*(t4814.*(t1861-t3221)+t2297.*(t642+t643-t667+t674+t1587+t1606+t1608+t1609+t2295+t2671+t2683+t2684-t2695+t3279+t3297-t3303+t3597+t3603+t3609-t3614+t4053+t4054)))./2.0;
t7295 = (t3217.*t7291)./2.0;
t7302 = (t3502.*t7291)./2.0;
t7312 = (t3910.*t7291)./2.0;
t7316 = (t3991.*t7291)./2.0;
t7324 = t3395.*t7308;
t7325 = t3396.*t7307;
t7342 = (t6682.*(-t2308+t2378+t2510-t2530-t2975+t2979+t3926+t4144+t4190+t4193+t4863+t4867))./2.0;
t7350 = (t6647.*t6651)./2.0;
t7353 = t4573.*t7307;
t7354 = t4577.*t7308;
t7355 = t4604.*t7308;
t7356 = -t7307.*(t3563-t4051);
t7361 = t3789+t3790+t3792+t3804+t4978+t4983+t4995+t4996+t5003+t5004+t5009+t5010;
t7362 = t3781+t3797+t3798+t3801+t4981+t4982+t4990+t4999+t5001+t5005+t5007+t5011;
t7398 = t7397.*(-1.0./2.0);
t7399 = t7397./2.0;
t7408 = t188.*t7407.*4.297799892626299e-1;
t7409 = (t2338.*t7407)./2.0;
t7438 = t6082+t6339+t6733;
t7444 = (t3915.*t7432)./2.0;
t7445 = t7433.*(-t1901+t3122+t3277).*(-1.0./2.0);
t7446 = (t4118.*t7432)./2.0;
t7448 = t7433.*(t951+t10.*(-t1881+t3121+t3276)).*(-1.0./2.0);
t7472 = t7471./2.0;
t7474 = t5035+t5280+t6302+t7168;
t7475 = t6136+t6471+t6874;
t7476 = t6139+t6477+t6873;
t7486 = -t7484;
t7487 = t3500.*(t6872+t6058.*(t1896-t3239)+t4019.*(t3435-t3448+t4615+t4619+t3976.*(t1896-t3239).*5.7e-7+t3980.*(t1896-t3239).*4.0e-8)).*(-1.0./2.0);
t7488 = t3503.*(t6137-t6873+t4031.*(t3435-t3448+t4615+t4619+t3976.*(t1896-t3239).*5.7e-7+t3980.*(t1896-t3239).*4.0e-8)).*(-1.0./2.0);
t7489 = (t3503.*(t6137-t6873+t4031.*(t3435-t3448+t4615+t4619+t3976.*(t1896-t3239).*5.7e-7+t3980.*(t1896-t3239).*4.0e-8)))./2.0;
t7490 = t3395.*t7477;
t7492 = t3396.*t7478;
t7511 = t3915.*(t6872+t6058.*(t1896-t3239)+t4019.*(t3435-t3448+t4615+t4619+t3976.*(t1896-t3239).*5.7e-7+t3980.*(t1896-t3239).*4.0e-8)).*(-1.0./2.0);
t7512 = ((-t1901+t3122+t3277).*(t6137-t6873+t4031.*(t3435-t3448+t4615+t4619+t3976.*(t1896-t3239).*5.7e-7+t3980.*(t1896-t3239).*4.0e-8)))./2.0;
t7517 = t4118.*(t6872+t6058.*(t1896-t3239)+t4019.*(t3435-t3448+t4615+t4619+t3976.*(t1896-t3239).*5.7e-7+t3980.*(t1896-t3239).*4.0e-8)).*(-1.0./2.0);
t7518 = (t4118.*(t6872+t6058.*(t1896-t3239)+t4019.*(t3435-t3448+t4615+t4619+t3976.*(t1896-t3239).*5.7e-7+t3980.*(t1896-t3239).*4.0e-8)))./2.0;
t7519 = ((t951+t10.*(-t1881+t3121+t3276)).*(t6137-t6873+t4031.*(t3435-t3448+t4615+t4619+t3976.*(t1896-t3239).*5.7e-7+t3980.*(t1896-t3239).*4.0e-8)))./2.0;
t7525 = t4577.*t7477;
t7526 = t4573.*t7478;
t7527 = t4604.*t7477;
t7528 = -t7478.*(t3563-t4051);
t7536 = t7534.*(-1.0./2.0);
t7537 = t7534./2.0;
t7540 = t6289+t6537+t6980;
t7596 = t7595.*(-1.0./2.0);
t7597 = t7595./2.0;
t7598 = (t5946.*t7462)./2.0;
t7600 = (t5949.*t7462)./2.0;
t7606 = (t5857.*t7473)./2.0;
t7608 = (t5858.*t7473)./2.0;
t7610 = t5859.*(t5034-t5280-t6302+t7166).*(-1.0./2.0);
t7611 = t5860.*(t5034-t5280-t6302+t7166).*(-1.0./2.0);
t7613 = -t7612;
t7615 = -t7614;
t7638 = t5428+t6145+t6150+t6151+t6579;
t7652 = t3395.*t7643;
t7653 = t3396.*t7644;
t7662 = t4573.*t7644;
t7663 = t4577.*t7643;
t7666 = t4604.*t7643;
t7667 = -t7644.*(t3563-t4051);
t7668 = (t6682.*t7462)./2.0;
t7670 = (t6647.*t7473)./2.0;
t7672 = t7462.*(t4853.*(t1896-t3239).*7.26735e-3+t2363.*(t684+t685-t710+t724+t1686-t1690+t1700+t1701+t2371+t2698+t2707-t2716+t2719+t3329-t3337-t3351-t3641+t3643+t3655-t3659+t4114+t4115).*7.26735e-3).*(-1.0./2.0);
t7675 = t7473.*(t4814.*(t1861-t3221)+t2297.*(t642+t643-t667+t674+t1587+t1606+t1608+t1609+t2295+t2671+t2683+t2684-t2695+t3279+t3297-t3303+t3597+t3603+t3609-t3614+t4053+t4054)).*(-1.0./2.0);
t7676 = (t7473.*(t4814.*(t1861-t3221)+t2297.*(t642+t643-t667+t674+t1587+t1606+t1608+t1609+t2295+t2671+t2683+t2684-t2695+t3279+t3297-t3303+t3597+t3603+t3609-t3614+t4053+t4054)))./2.0;
t7677 = (t6682.*t7479)./2.0;
t7682 = t5552+t6329+t6332+t6333+t6670;
et277 = t5080-t7199+t4853.*(t1005+t20.*(t1941-t3315+t39.*t1022.*(t855-t878).*2.196325630278387e-1)).*7.26735e-3;
et278 = t2419.*(t684+t685-t710+t724+t1686-t1690+t1700+t1701+t2371+t2698+t2707-t2716+t2719+t3329-t3337-t3351-t3641+t3643+t3655-t3659+t4114+t4115).*7.26735e-3;
t7683 = t6647.*(et277+et278).*(-1.0./2.0);
t7688 = t5546+t6334+t6337+t6338+t6734;
t7689 = t3216.*(t6326-t6665+t5382.*(t1896-t3239)+t6098.*(t3242-t3554)+t6100.*(t3242-t3554)).*(-1.0./2.0);
t7690 = (t3216.*(t6326-t6665+t5382.*(t1896-t3239)+t6098.*(t3242-t3554)+t6100.*(t3242-t3554)))./2.0;
t7695 = ((t2674-t2676+t3022-t3027).*(t6326-t6665+t5382.*(t1896-t3239)+t6098.*(t3242-t3554)+t6100.*(t3242-t3554)))./2.0;
t7697 = t5814+t5852+t5984+t6120+t6232+t6567;
t7703 = t50.*t189.*(t5618+t6429-t6902+t3055.*(t4795+t4801+t4808+t3976.*(t2694-t2701+t3036-t3043).*5.7e-7)+t6384.*(t1477-t2502)).*(-4.771516396025243e-17);
t7704 = t5670+t6472+t6473+t6475+t6871;
t7716 = t5864+t5973+t6037+t6218+t6412+t6605;
t7724 = t5754+t6529+t6531+t6535+t6978;
t7725 = t5756+t6534+t6536+t6538+t6984;
t7791 = t6052+t6079+t6198+t6417+t6606+t6881;
t7801 = t3216.*(-t5828-t5829+t6593+t6596+t22.*t6699.*(t3242-t3554)+t28.*t6696.*(t3242-t3554)).*(-1.0./2.0);
t7809 = ((t2674-t2676+t3022-t3027).*(-t5828-t5829+t6593+t6596+t22.*t6699.*(t3242-t3554)+t28.*t6696.*(t3242-t3554)))./2.0;
t7811 = t3980.*(-t5828-t5829+t6593+t6596+t22.*t6699.*(t3242-t3554)+t28.*t6696.*(t3242-t3554)).*(-1.0./2.0);
t7812 = (t3980.*(-t5828-t5829+t6593+t6596+t22.*t6699.*(t3242-t3554)+t28.*t6696.*(t3242-t3554)))./2.0;
t7814 = t7804.*(t1861-t3221).*(-1.0./2.0);
t7815 = (t7804.*(t1861-t3221))./2.0;
t7816 = (t3502.*t7805)./2.0;
t7823 = t7804.*(t2674-t2676+t3022-t3027).*(-1.0./2.0);
t7824 = (t3910.*t7805)./2.0;
t7829 = t6085+t6282+t6704+t6974+t7126+t7322;
et279 = t6083+t6281-t6704+t7092.*(t1477-t2502)+t3055.*(t3131+t3132+t3171+t3446-t4281-t4282-t4301+t4303-t4308+t4310-t4583-t4594+t4623+t4639+t2388.*(t1456-t2355).*4.0e-8+(t3543.*(t1861-t3221))./1.0e+8+(t3500.*(t1896-t3239))./1.0e+8-t11.*t2297.*t2363.*2.4e-7);
et280 = t2363.*(t3157+t3158+t3386-t4299-t4300-t4562+t4567+t3543.*(t1861-t3221).*6.2e-7+t3500.*(t1896-t3239).*6.2e-7-(t11.*(t1861-t3221).*(t1896-t3239))./1.0e+8-(t11.*t2297.*t2363)./1.0e+8-(t11.*t3502.*t3547)./1.0e+8);
t7830 = t2297.*(et279+et280).*(-1.0./2.0);
t7837 = t6135+t6404+t6806+t7020+t7209+t7339;
t7838 = t6138+t6405+t6807+t7021+t7210+t7340;
t7867 = t5985+t6140+t6573+t7278+t7348+t7471;
et281 = t3704+t3707-t3863+t4904+t4912-t5154+t5155-t5186+t3370.*(t1477-t2502).*9.3e-7+t4031.*(t3512-t4006).*9.0e-8+t12.*t3980.*(t3242-t3554).*9.0e-8;
et282 = t17.*t3980.*(t3242-t3554).*9.3e-7;
et283 = t3216;
et284 = -t5939-t6747+t4577.*(et281+et282)+t4573.*(t3703+t3708-t3856+t4903+t4911-t5153+t5161-t5190+t12.*t4887+t3370.*(t1477-t2502).*9.0e-8+t4031.*(t3512-t4006).*1.02e-6+t17.*t3980.*(t3242-t3554).*9.0e-8)+t22.*t6993.*(t3242-t3554)+t28.*t6992.*(t3242-t3554);
et285 = -1.0./2.0;
t7884 = et283.*et284.*et285;
et286 = t3704+t3707-t3863+t4904+t4912-t5154+t5155-t5186+t3370.*(t1477-t2502).*9.3e-7+t4031.*(t3512-t4006).*9.0e-8+t12.*t3980.*(t3242-t3554).*9.0e-8;
et287 = t17.*t3980.*(t3242-t3554).*9.3e-7;
et288 = t3216;
et289 = -t5939-t6747+t4577.*(et286+et287)+t4573.*(t3703+t3708-t3856+t4903+t4911-t5153+t5161-t5190+t12.*t4887+t3370.*(t1477-t2502).*9.0e-8+t4031.*(t3512-t4006).*1.02e-6+t17.*t3980.*(t3242-t3554).*9.0e-8)+t22.*t6993.*(t3242-t3554)+t28.*t6992.*(t3242-t3554);
et290 = 1.0./2.0;
t7885 = et288.*et289.*et290;
et291 = t3704+t3707-t3863+t4904+t4912-t5154+t5155-t5186+t3370.*(t1477-t2502).*9.3e-7+t4031.*(t3512-t4006).*9.0e-8+t12.*t3980.*(t3242-t3554).*9.0e-8;
et292 = t17.*t3980.*(t3242-t3554).*9.3e-7;
et293 = t2674-t2676+t3022-t3027;
et294 = -t5939-t6747+t4577.*(et291+et292)+t4573.*(t3703+t3708-t3856+t4903+t4911-t5153+t5161-t5190+t12.*t4887+t3370.*(t1477-t2502).*9.0e-8+t4031.*(t3512-t4006).*1.02e-6+t17.*t3980.*(t3242-t3554).*9.0e-8)+t22.*t6993.*(t3242-t3554)+t28.*t6992.*(t3242-t3554);
et295 = 1.0./2.0;
t7888 = et293.*et294.*et295;
et296 = t3704+t3707-t3863+t4904+t4912-t5154+t5155-t5186+t3370.*(t1477-t2502).*9.3e-7+t4031.*(t3512-t4006).*9.0e-8+t12.*t3980.*(t3242-t3554).*9.0e-8;
et297 = t17.*t3980.*(t3242-t3554).*9.3e-7;
et298 = t3980;
et299 = -t5939-t6747+t4577.*(et296+et297)+t4573.*(t3703+t3708-t3856+t4903+t4911-t5153+t5161-t5190+t12.*t4887+t3370.*(t1477-t2502).*9.0e-8+t4031.*(t3512-t4006).*1.02e-6+t17.*t3980.*(t3242-t3554).*9.0e-8)+t22.*t6993.*(t3242-t3554)+t28.*t6992.*(t3242-t3554);
et300 = -1.0./2.0;
t7891 = et298.*et299.*et300;
t7893 = t6106+t6510+t6861+t7286+t7365+t7485;
t7895 = t3216.*(-t6510+t7364+t7483+t5918.*(t1005+t20.*(t1941-t3315+t39.*t1022.*(t855-t878).*2.196325630278387e-1))+t6549.*(t4165+t27.*(t1959-t3313+t38.*t1022.*(t855-t878).*2.196325630278387e-1))+t7277.*(t1896-t3239)).*(-1.0./2.0);
t7897 = ((t1861-t3221).*(-t6510+t7364+t7483+t5918.*(t1005+t20.*(t1941-t3315+t39.*t1022.*(t855-t878).*2.196325630278387e-1))+t6549.*(t4165+t27.*(t1959-t3313+t38.*t1022.*(t855-t878).*2.196325630278387e-1))+t7277.*(t1896-t3239)))./2.0;
t7899 = t6084+t6313+t6716+t7297+t7376+t7531;
t7915 = t6252+t6591+t6998+t7309+t7387+t7555;
t7916 = t6253+t6592+t6997+t7310+t7389+t7556;
t7921 = t3217.*(t6251-t6997-t7310+t7388+t7554+t4880.*(t3435-t3448+t4615+t4619+t3976.*(t1896-t3239).*5.7e-7+t3980.*(t1896-t3239).*4.0e-8)).*(-1.0./2.0);
t7923 = t3502.*(t6251-t6997-t7310+t7388+t7554+t4880.*(t3435-t3448+t4615+t4619+t3976.*(t1896-t3239).*5.7e-7+t3980.*(t1896-t3239).*4.0e-8)).*(-1.0./2.0);
t7947 = t6415+t6660+t7100+t7403+t7459+t7659;
t5418 = -t5417;
t5811 = t4459+t5409;
t5841 = t4493+t5432;
t5862 = t4676+t5454;
t6157 = -t6156;
t6161 = -t6160;
t6179 = -t6177;
t6182 = -t6181;
t6296 = -t6295;
t6300 = -t6299;
t6305 = (t3910.*(t4675-t5454).*(t1488+t1874+t2519+t2740+t2747+t3096+t3097))./2.0;
t6374 = -t6373;
t6395 = -t6393;
t6437 = -t6436;
t6450 = -t6449;
t6453 = -t6452;
t6505 = -t6504;
t6507 = -t6506;
t6554 = t6552./2.0;
t6556 = -t6553;
t6557 = t6553./2.0;
t6611 = t6609./2.0;
t6613 = t6610./2.0;
t6618 = -t6617;
t6619 = t6616./2.0;
t6620 = t6617./2.0;
t6628 = t6626./2.0;
t6630 = t3395.*t6583;
t6634 = -t6631;
t6637 = t3396.*t6585;
t6639 = t6633./2.0;
t6640 = t6636./2.0;
t6650 = t5046+t6269;
t6689 = t5063+t6322;
t6701 = -t6700;
t6703 = -t6702;
t6707 = -t6706;
t6709 = -t6708;
t6711 = t5113+t6363;
t6727 = t6724./2.0;
t6728 = t6725./2.0;
t6736 = t5859.*(t4675-t5454).*(-1.0./2.0);
t6737 = (t5859.*(t4675-t5454))./2.0;
t6738 = t5860.*(t4675-t5454).*(-1.0./2.0);
t6739 = (t5860.*(t4675-t5454))./2.0;
t6742 = t6740./2.0;
t6743 = -t6741;
t6744 = t6741./2.0;
t6754 = -t6752;
t6755 = t6752./2.0;
t6759 = t6756.*(-1.0./2.0);
t6760 = t6756./2.0;
t6763 = -t6761;
t6764 = -t6762;
t6768 = t6766./2.0;
t6769 = t6767./2.0;
t6778 = t6773./2.0;
t6779 = t6774./2.0;
t6780 = -t6776;
t6783 = t6775./2.0;
t6784 = -t6777;
t6786 = t6777./2.0;
t6793 = t5197+t6391;
t6795 = t6791./2.0;
t6796 = -t6794;
t6798 = t6794./2.0;
t6803 = t6801./2.0;
t6817 = -t6812;
t6820 = t6813./2.0;
t6821 = t6814./2.0;
t6823 = -t6818;
t6825 = t6816./2.0;
t6826 = t6818./2.0;
t6838 = -t6837;
t6841 = -t6840;
t6843 = t4577.*t6583;
t6844 = t4573.*t6585;
t6848 = t4604.*t6583;
t6849 = -t6847;
t6853 = -t6585.*(t3563-t4051);
t6855 = -t6852;
t6866 = -t6864;
t6867 = -t6865;
t6885 = -t6884;
t6889 = -t6888;
t6908 = -t6907;
t6912 = -t6911;
t6931 = -t6927;
t6950 = -t6944;
t6973 = -t6972;
t6986 = -t6985;
t6996 = -t6995;
t7024 = t7022./2.0;
t7025 = t7023./2.0;
t7031 = -t7030;
t7034 = t7032./2.0;
t7036 = -t7033;
t7038 = t7033./2.0;
t7047 = -t7045;
t7049 = -t7046;
t7052 = -t7051;
t7062 = t7060./2.0;
t7065 = -t7064;
t7072 = -t7068;
t7076 = t7069./2.0;
t7078 = t7071./2.0;
t7108 = -t7106;
t7109 = -t7107;
t7131 = -t7129;
t7132 = -t7130;
t7186 = -t7182;
t7248 = -t7247;
t7262 = -t7261;
t7285 = t4846+t5126+t5723+t6364;
t7289 = t4928+t5199+t5762+t6392;
t7303 = -t7302;
t7326 = t7324./2.0;
t7327 = -t7325;
t7328 = t7325./2.0;
t7336 = t3934.*(t4844+t5119-t5723-t6364).*(t1513+t1879+t2598+t2820+t2834+t3117+t3118).*3.633675e-3;
t7346 = (t3910.*(t4927+t5198-t5762-t6392).*(t1488+t1874+t2519+t2740+t2747+t3096+t3097))./2.0;
t7351 = -t7350;
t7367 = t3395.*t7362;
t7369 = t3396.*t7361;
t7390 = t4573.*t7361;
t7391 = t4577.*t7362;
t7392 = t4604.*t7362;
t7393 = -t7361.*(t3563-t4051);
t7414 = t5859.*(t4927+t5198-t5762-t6392).*(-1.0./2.0);
t7415 = t5860.*(t4927+t5198-t5762-t6392).*(-1.0./2.0);
t7418 = t5958.*(t4844+t5119-t5723-t6364).*(-1.0./2.0);
t7419 = (t5958.*(t4844+t5119-t5723-t6364))./2.0;
t7420 = t5962.*(t4844+t5119-t5723-t6364).*(-1.0./2.0);
t7421 = (t5962.*(t4844+t5119-t5723-t6364))./2.0;
t7439 = t188.*t7438.*4.297799892626299e-1;
t7441 = (t2307.*t7438)./2.0;
t7443 = (t2338.*t7438)./2.0;
t7447 = -t7446;
t7450 = t188.*(-t6772+t6776+t3055.*(-t3434+t4606+t3980.*(t1896-t3239).*1.02e-6)).*(-4.297799892626299e-1);
t7451 = t188.*(-t6772+t6776+t3055.*(-t3434+t4606+t3980.*(t1896-t3239).*1.02e-6)).*4.297799892626299e-1;
t7452 = t2307.*(-t6772+t6776+t3055.*(-t3434+t4606+t3980.*(t1896-t3239).*1.02e-6)).*(-1.0./2.0);
t7453 = t11.*t2297.*(-t6772+t6776+t3055.*(-t3434+t4606+t3980.*(t1896-t3239).*1.02e-6)).*(-1.0./2.0);
t7454 = (t2307.*(-t6772+t6776+t3055.*(-t3434+t4606+t3980.*(t1896-t3239).*1.02e-6)))./2.0;
t7455 = (t11.*t2297.*(-t6772+t6776+t3055.*(-t3434+t4606+t3980.*(t1896-t3239).*1.02e-6)))./2.0;
t7456 = t2338.*(-t6772+t6776+t3055.*(-t3434+t4606+t3980.*(t1896-t3239).*1.02e-6)).*(-1.0./2.0);
t7460 = t2994.*(-t6772+t6776+t3055.*(-t3434+t4606+t3980.*(t1896-t3239).*1.02e-6)).*(-1.0./2.0);
t7463 = t5013+t5255+t6265+t7138;
t7469 = t5712+t6845+t6846;
t7470 = t5710+t6850+t6854;
t7480 = t5049+t5312+t6365+t7160;
t7491 = t7490./2.0;
t7493 = -t7492;
t7494 = t7492./2.0;
t7523 = t5794+t6928+t6930;
t7524 = t5801+t6934+t6938;
t7544 = t5833+t6946+t6948;
t7548 = t5832+t6952+t6957;
t7599 = -t7598;
t7601 = -t7600;
t7607 = -t7606;
t7609 = -t7608;
t7630 = t5943+t7183+t7185;
t7631 = t5942+t7189+t7193;
t7639 = t50.*t189.*t7638.*4.771516396025243e-17;
t7654 = t7652./2.0;
t7655 = -t7653;
t7656 = t7653./2.0;
t7664 = -t7662;
t7665 = -t7663;
t7681 = t5551+t6327+t6328+t6330+t6665;
t7691 = (t3217.*t7682)./2.0;
t7696 = (t3910.*t7682)./2.0;
t7702 = t5622+t6426+t6427+t6434+t6902;
t7705 = t5671+t6474+t6476+t6478+t6876;
t7706 = t5489+t5492+t6191+t6193+t6609+t6610;
t7707 = t50.*t189.*(t5490+t6190-t6193-t6609-t6610+t5405.*(t1477-t2502)).*(-4.771516396025243e-17);
t7708 = t3047.*(t5490+t6190-t6193-t6609-t6610+t5405.*(t1477-t2502)).*(-1.0./2.0);
t7710 = t4520+t4522+t4537+t4545+t6496+t6499+t6542+t6545;
t7711 = t4520+t4522+t4537+t4545+t6498+t6500+t6542+t6545;
t7712 = t4520+t4522+t4537+t4545+t6496+t6499+t6544+t6546;
t7713 = t4520+t4522+t4537+t4545+t6498+t6500+t6544+t6546;
t7727 = (t3216.*t7724)./2.0;
t7730 = (t3217.*t7725)./2.0;
t7735 = t7724.*(t2674-t2676+t3022-t3027).*(-1.0./2.0);
t7736 = (t7724.*(t2674-t2676+t3022-t3027))./2.0;
t7738 = (t3910.*t7725)./2.0;
t7742 = t5582+t5583+t6375+t6379+t6724+t6725;
t7746 = t5709+t5711+t6439+t6441+t6720+t6723;
t7747 = t5715+t5716+t6443+t6444+t6719+t6722;
t7750 = t5681+t5683+t6463+t6464+t6766+t6767;
t7752 = t3217.*(t5713+t5714-t6443-t6719-t6722+t6102.*(t3563-t4051)).*(-1.0./2.0);
t7753 = t50.*t189.*(t6462-t6464-t6766-t6767+t3055.*(t4809+t3976.*(t2694-t2701+t3036-t3043).*1.02e-6)+t5572.*(t1477-t2502)).*(-4.771516396025243e-17);
t7754 = t50.*t189.*(t6462-t6464-t6766-t6767+t3055.*(t4809+t3976.*(t2694-t2701+t3036-t3043).*1.02e-6)+t5572.*(t1477-t2502)).*4.771516396025243e-17;
t7756 = t6935+t6936+t6939+t6940;
t7757 = t3047.*(t6462-t6464-t6766-t6767+t3055.*(t4809+t3976.*(t2694-t2701+t3036-t3043).*1.02e-6)+t5572.*(t1477-t2502)).*(-1.0./2.0);
t7763 = t3910.*(t5713+t5714-t6443-t6719-t6722+t6102.*(t3563-t4051)).*(-1.0./2.0);
t7767 = t3991.*(t5713+t5714-t6443-t6719-t6722+t6102.*(t3563-t4051)).*(-1.0./2.0);
t7773 = t6953+t6954+t6956+t6958;
t7792 = (t2297.*t7791)./2.0;
t7794 = t5795+t5799+t6559+t6560+t6862+t6863;
t7796 = t7067+t7069+t7071+t7075;
t7797 = t5828+t5829+t6597+t6598+t6890+t6891;
t7798 = t5831+t5837+t6599+t6600+t6892+t6893;
t7807 = t3502.*(t5637+t5773-t6685-t6910+t6911+t6490.*(t3563-t4051)).*(-1.0./2.0);
t7808 = (t3502.*(t5637+t5773-t6685-t6910+t6911+t6490.*(t3563-t4051)))./2.0;
t7817 = -t7816;
t7820 = t3910.*(t5637+t5773-t6685-t6910+t6911+t6490.*(t3563-t4051)).*(-1.0./2.0);
t7822 = t3991.*(t5637+t5773-t6685-t6910+t6911+t6490.*(t3563-t4051)).*(-1.0./2.0);
t7826 = t7188+t7190+t7191+t7194;
t7835 = t3416+t3765+t3766+t4030+t4039+t4041+t4270+t4272+t4318+t4372+t4373+t5997+t6000+t6043+t6046+t6455+t6458+t6519+t6521;
t7836 = t3416+t3765+t3766+t4030+t4039+t4041+t4270+t4272+t4318+t4372+t4373+t5999+t6001+t6045+t6047+t6457+t6459+t6520+t6522;
t7840 = (t3502.*t7838)./2.0;
t7842 = (t3910.*t7838)./2.0;
t7845 = ((t1861-t3221).*(t5691+t6884-t6886-t7353-t7354+t6065.*(t3242-t3554)))./2.0;
t7847 = t3502.*(t6263-t6887+t6888-t7355+t7307.*(t3563-t4051)+t21.*t3547.*(-t3434+t4606+t3980.*(t1896-t3239).*1.02e-6)).*(-1.0./2.0);
t7848 = ((t2674-t2676+t3022-t3027).*(t5691+t6884-t6886-t7353-t7354+t6065.*(t3242-t3554)))./2.0;
t7850 = t3910.*(t6263-t6887+t6888-t7355+t7307.*(t3563-t4051)+t21.*t3547.*(-t3434+t4606+t3980.*(t1896-t3239).*1.02e-6)).*(-1.0./2.0);
t7851 = t3980.*(t5691+t6884-t6886-t7353-t7354+t6065.*(t3242-t3554)).*(-1.0./2.0);
t7852 = t3991.*(t6263-t6887+t6888-t7355+t7307.*(t3563-t4051)+t21.*t3547.*(-t3434+t4606+t3980.*(t1896-t3239).*1.02e-6)).*(-1.0./2.0);
t7858 = t5845+t6624+t7022+t7023+t7394+t7397;
et301 = t50.*t189.*(t7022+t7023+t7394+t7397-t5792.*(t1477-t2502)-t3055.*(t4876+t4905+t4906+t3055.*(t1456-t2355).*1.02e-6+t3047.*(t1477-t2502).*1.02e-6+t3976.*(t3242-t3554).*1.02e-6));
et302 = 4.771516396025243e-17;
t7859 = et301.*et302;
t7860 = (t3047.*(t7022+t7023+t7394+t7397-t5792.*(t1477-t2502)-t3055.*(t4876+t4905+t4906+t3055.*(t1456-t2355).*1.02e-6+t3047.*(t1477-t2502).*1.02e-6+t3976.*(t3242-t3554).*1.02e-6)))./2.0;
t7868 = t50.*t189.*t7867.*4.771516396025243e-17;
t7869 = (t2297.*t7867)./2.0;
t7880 = t3126+t3193+t3194+t3209+t3463+t3480+t3490+t3588+t3820+t3821+t3891+t3895+t4205+t4337+t4342+t4413+t4417+t5588+t5591+t5718+t5721+t5906+t5912+t6007+t6009+t6446+t6449+t6502+t6504;
t7882 = t5939+t6747+t7104+t7105+t7422+t7423;
t7894 = t6107+t6511+t6860+t7287+t7366+t7486;
t7900 = t50.*t189.*t7899.*4.771516396025243e-17;
t7902 = (t2297.*t7899)./2.0;
t7909 = t5888+t6815+t7044+t7050+t7527+t7528;
t7924 = t5672+t6801+t6802+t7054+t7592+t7595;
t7925 = t5965+t6905+t7119+t7122+t7571+t7572;
t7926 = t5963+t6906+t7121+t7124+t7573+t7574;
t7939 = t6018+t7120+t7144+t7146+t7622+t7623;
t7940 = t6017+t7123+t7145+t7147+t7625+t7627;
t7948 = t5590+t5992+t5994+t6270+t6345+t6355+t6508+t6509+t6923+t6926+t7315+t7316;
t7949 = t5590+t5992+t5994+t6270+t6348+t6358+t6508+t6509+t6923+t6926+t7315+t7316;
t7951 = t6109+t7214+t7239+t7241+t7666+t7667;
t7952 = t3216.*(t7211-t7238-t7240+t7662+t7663+t5792.*(t4165+t27.*(t1959-t3313+t38.*t1022.*(t855-t878).*2.196325630278387e-1))).*(-1.0./2.0);
t7953 = (t3216.*(t7211-t7238-t7240+t7662+t7663+t5792.*(t4165+t27.*(t1959-t3313+t38.*t1022.*(t855-t878).*2.196325630278387e-1))))./2.0;
t7955 = ((t1861-t3221).*(t7211-t7238-t7240+t7662+t7663+t5792.*(t4165+t27.*(t1959-t3313+t38.*t1022.*(t855-t878).*2.196325630278387e-1))))./2.0;
t7957 = t3980.*(t7211-t7238-t7240+t7662+t7663+t5792.*(t4165+t27.*(t1959-t3313+t38.*t1022.*(t855-t878).*2.196325630278387e-1))).*(-1.0./2.0);
t7965 = t2965+t2966+t3195+t3205+t3318+t3324+t3474+t3496+t3688+t3689+t3770+t3823+t3906+t3967+t4244+t4286+t4458+t4461+t4486+t4488+t4663+t4665+t4704+t4708+t6131+t6134+t6164+t6168+t6656+t6658+t6678+t6680+t7226+t7230+t7233+t7235;
t7966 = t2965+t2966+t3195+t3205+t3318+t3324+t3474+t3496+t3688+t3689+t3770+t3823+t3906+t3967+t4244+t4286+t4458+t4461+t4486+t4488+t4677+t4680+t4728+t4730+t6129+t6133+t6162+t6166+t6654+t6657+t6673+t6679+t7224+t7229+t7232+t7234;
t7975 = t2965+t2966+t3195+t3205+t3318+t3324+t3474+t3496+t3688+t3689+t3770+t3823+t3906+t3967+t4244+t4286+t4458+t4461+t4486+t4488+t4677+t4680+t4704+t4708+t5655+t5659+t5675+t5677+t5920+t5923+t5935+t5948+t6129+t6133+t6164+t6168+t6293+t6298+t6317+t6323+t6654+t6657+t6678+t6680+t7224+t7229+t7233+t7235;
t7976 = t2965+t2966+t3195+t3205+t3318+t3324+t3474+t3496+t3688+t3689+t3770+t3823+t3906+t3967+t4244+t4286+t4458+t4461+t4486+t4488+t4663+t4665+t4728+t4730+t5776+t5778+t5787+t5788+t6020+t6021+t6027+t6029+t6131+t6134+t6162+t6166+t6408+t6410+t6420+t6421+t6656+t6658+t6673+t6679+t7226+t7230+t7232+t7234;
t5848 = t4651+t5418;
t6229 = t3934.*t5811.*(t1513+t1879+t2598+t2820+t2834+t3117+t3118).*(-3.633675e-3);
t6230 = t3934.*t5811.*(t1513+t1879+t2598+t2820+t2834+t3117+t3118).*3.633675e-3;
t6259 = t3910.*t5841.*(t1488+t1874+t2519+t2740+t2747+t3096+t3097).*(-1.0./2.0);
t6261 = (t3910.*t5841.*(t1488+t1874+t2519+t2740+t2747+t3096+t3097))./2.0;
t6555 = -t6554;
t6558 = -t6557;
t6612 = -t6611;
t6614 = -t6613;
t6621 = -t6620;
t6632 = -t6630;
t6635 = t6630./2.0;
t6641 = -t6639;
t6642 = -t6640;
t6643 = t6637./2.0;
t6694 = (t5841.*t5859)./2.0;
t6695 = (t5841.*t5860)./2.0;
t6729 = -t6727;
t6730 = -t6728;
t6746 = -t6744;
t6757 = -t6755;
t6770 = -t6768;
t6771 = -t6769;
t6781 = -t6778;
t6782 = -t6779;
t6785 = -t6783;
t6787 = -t6786;
t6792 = (t5811.*t5958)./2.0;
t6797 = -t6795;
t6799 = (t5811.*t5962)./2.0;
t6800 = -t6798;
t6822 = -t6820;
t6824 = -t6821;
t6827 = -t6825;
t6828 = -t6826;
t6959 = t3934.*t3951.*t6650.*3.633675e-3;
t6975 = t3934.*t4187.*t6650.*3.633675e-3;
t6989 = (t3910.*t3925.*t6689)./2.0;
t7001 = (t3910.*t4146.*t6689)./2.0;
t7012 = t3934.*t4018.*t6711.*3.633675e-3;
t7026 = t3934.*t4187.*t6711.*3.633675e-3;
t7037 = -t7034;
t7039 = -t7038;
t7066 = (t3910.*t3975.*t6793)./2.0;
t7084 = (t3910.*t4146.*t6793)./2.0;
t7102 = (t5369.*t6650)./2.0;
t7112 = (t5275.*t6689)./2.0;
t7114 = (t5373.*t6650)./2.0;
t7125 = (t5317.*t6689)./2.0;
t7142 = (t5423.*t6650)./2.0;
t7156 = (t5377.*t6689)./2.0;
t7161 = (t5369.*t6711)./2.0;
t7174 = (t5373.*t6711)./2.0;
t7176 = (t5275.*t6793)./2.0;
t7179 = (t5317.*t6793)./2.0;
t7200 = (t5423.*t6711)./2.0;
t7206 = (t5377.*t6793)./2.0;
t7216 = (t5791.*t6650)./2.0;
t7218 = (t5771.*t6689)./2.0;
t7220 = (t5841.*t6650)./2.0;
t7222 = (t5811.*t6689)./2.0;
t7231 = t6650.*(t4675-t5454).*(-1.0./2.0);
t7244 = (t5855.*t6689)./2.0;
t7249 = (t5841.*t6711)./2.0;
t7251 = (t5857.*t6689)./2.0;
t7254 = (t5811.*t6793)./2.0;
t7257 = (t5904.*t6650)./2.0;
t7259 = t6711.*(t4675-t5454).*(-1.0./2.0);
t7263 = (t5946.*t6650)./2.0;
t7266 = (t5855.*t6793)./2.0;
t7269 = (t5857.*t6793)./2.0;
t7272 = (t5904.*t6711)./2.0;
t7275 = (t5946.*t6711)./2.0;
t7329 = -t7328;
t7343 = (t6588.*t6689)./2.0;
t7347 = -t7346;
t7352 = (t6650.*t6652)./2.0;
t7359 = (t6588.*t6793)./2.0;
t7363 = (t6652.*t6711)./2.0;
t7368 = -t7367;
t7370 = t7367./2.0;
tau_c = ft_16({dq1,dq2,dq3,dq4,dq5,dq6,t10,t1005,t1022,t1089,t11,t1104,t1105,t1108,t1115,t1121,t1158,t1159,t1196,t12,t1205,t1210,t1212,t1217,t1218,t123,t1237,t1238,t1288,t1289,t13,t1302,t1303,t1319,t1320,t1336,t1348,t1350,t1351,t1360,t1369,t1378,t1396,t14,t140,t1425,t1435,t1456,t1477,t1488,t15,t1513,t1539,t1554,t1577,t1578,t1586,t1587,t16,t1600,t1606,t1608,t1609,t1629,t1637,t1640,t1641,t1659,t1661,t1666,t1667,t1683,t1686,t1690,t1692,t17,t1700,t1701,t1705,t1712,t1758,t1759,t1775,t1776,t18,t1861,t1874,t1879,t188,t1881,t189,t1896,t19,t1901,t1941,t1959,t1973,t1993,t1994,t20,t201,t202,t2023,t2053,t2060,t2089,t2090,t2098,t2099,t21,t2117,t2120,t2122,t2123,t2139,t2140,t2147,t2152,t2154,t2155,t2159,t2165,t2174,t2183,t2187,t2193,t2194,t2195,t2199,t22,t2203,t2215,t2219,t2222,t2223,t2239,t2240,t2256,t2257,t2292,t2295,t2297,t2303,t2306,t2307,t2317,t2337,t2338,t2339,t2355,t236,t2361,t2362,t2363,t2367,t2368,t237,t2371,t238,t2388,t2399,t24,t241,t2414,t2419,t25,t2502,t2519,t2527,t2555,t2556,t2572,t2583,t2598,t26,t2605,t2606,t2612,t2613,t2618,t2619,t262,t264,t2651,t2652,t2671,t2674,t2676,t2683,t2684,t2689,t2694,t2695,t2698,t27,t2701,t2707,t2716,t2719,t2740,t2747,t2748,t2749,t2754,t2773,t2781,t2788,t28,t2801,t2804,t2813,t2814,t2820,t2831,t2834,t2835,t2838,t2850,t2851,t29,t2953,t2965,t2966,t2990,t2991,t2994,t30,t3009,t3015,t3022,t3027,t3030,t3036,t3043,t3047,t3055,t3057,t3058,t3064,t3068,t3072,t3080,t3096,t3097,t31,t3109,t3117,t3118,t3121,t3122,t3126,t3129,t313,t3131,t3132,t3133,t314,t3145,t3148,t3157,t3158,t3171,t3193,t3194,t3195,t32,t3200,t3201,t3205,t3208,t3209,t321,t3211,t3213,t3216,t3217,t3221,t3235,t3236,t3237,t3238,t3239,t3242,t3276,t3277,t3279,t3290,t3297,t3299,t33,t3303,t3312,t3313,t3315,t3318,t332,t3322,t3324,t3328,t3329,t3337,t3340,t3344,t335,t3351,t3359,t3369,t3370,t3386,t3395,t3396,t34,t3405,t3409,t3415,t3416,t3420,t3423,t3428,t3431,t3432,t3434,t3435,t3446,t3448,t3463,t3468,t3471,t3474,t3480,t3482,t3483,t3488,t3490,t3496,t3499,t35,t350,t3500,t3502,t3503,t3512,t3517,t3524,t3543,t3547,t3554,t3563,t3566,t3582,t3588,t3590,t3591,t3592,t3597,t36,t3603,t3609,t3611,t3614,t3638,t3639,t3640,t3641,t3642,t3643,t3649,t3655,t3658,t3659,t366,t3670,t3688,t3689,t3703,t3704,t3707,t3708,t3712,t3716,t3717,t3739,t3746,t3755,t3765,t3766,t3770,t38,t3805,t3808,t3809,t3810,t3817,t3818,t3820,t3821,t3823,t3840,t3846,t3856,t3862,t3863,t3876,t3877,t3878,t3879,t3880,t3890,t3891,t3893,t3895,t3896,t3897,t3898,t39,t3901,t3902,t3903,t3906,t3910,t3913,t3915,t3924,t3925,t3931,t3934,t3937,t3943,t3951,t3961,t3967,t3968,t3974,t3975,t3976,t3980,t3985,t3991,t3993,t4001,t4006,t4008,t4018,t4019,t4026,t4030,t4031,t4032,t4035,t4039,t4041,t4045,t4047,t4049,t4051,t4053,t4054,t4065,t410,t4100,t4109,t4110,t4114,t4115,t4118,t4146,t4147,t4153,t4154,t4157,t4158,t4165,t4172,t4187,t4198,t42,t4201,t4205,t4208,t4213,t4215,t4236,t4240,t4244,t4260,t4261,t4263,t4270,t4272,t4273,t4274,t4275,t4281,t4282,t4286,t4287,t4288,t4299,t43,t4300,t4301,t4303,t4308,t4310,t4313,t4314,t4318,t4324,t4325,t4326,t4330,t4332,t4334,t4337,t4339,t4341,t4342,t4343,t4346,t4352,t4359,t4371,t4372,t4373,t4375,t4413,t4415,t4416,t4417,t4458,t4461,t4464,t4468,t4470,t4476,t4486,t4488,t4489,t4494,t4495,t4501,t4502,t4504,t4515,t4518,t4553,t4559,t4562,t4563,t4567,t4570,t4573,t4576,t4577,t4582,t4583,t4594,t46,t4603,t4604,t4606,t4615,t4617,t4618,t4619,t4623,t4634,t4635,t4639,t4644,t4645,t4652,t4658,t4663,t4665,t4673,t4675,t4677,t4678,t4680,t4683,t47,t4703,t4704,t4705,t4708,t4709,t4713,t4716,t4719,t4722,t4724,t4725,t4728,t4730,t4741,t4744,t4746,t4751,t4757,t4760,t4761,t4762,t4763,t4795,t4799,t4801,t4808,t4809,t4814,t4823,t4828,t4833,t4835,t4838,t4843,t4844,t4847,t4850,t4853,t4872,t4874,t4876,t4879,t4880,t4887,t4895,t4902,t4903,t4904,t4905,t4906,t4911,t4912,t4915,t4920,t4923,t4924,t4925,t4927,t4950,t50,t5014,t5016,t5025,t5026,t5027,t5028,t5034,t5036,t5037,t5038,t5041,t5042,t5043,t5080,t5082,t5083,t5084,t5085,t5086,t5087,t5088,t5089,t5090,t5091,t5093,t5096,t5097,t5098,t5103,t5105,t5106,t5108,t5119,t5141,t5142,t5153,t5154,t5155,t5161,t5164,t5167,t5169,t5183,t5184,t5185,t5186,t5189,t5190,t5194,t5198,t5200,t5201,t5202,t5205,t5213,t5214,t5234,t5236,t5240,t5243,t5246,t5247,t5248,t5249,t5251,t5256,t5257,t5258,t5259,t5262,t5264,t5265,t5278,t5279,t5280,t5283,t5286,t5287,t5291,t5296,t5297,t5301,t5302,t5303,t5304,t5305,t5306,t5308,t5309,t5313,t5328,t5331,t5332,t5333,t5336,t5337,t5340,t5341,t5343,t5344,t5345,t5346,t5352,t5353,t5356,t5358,t5359,t5361,t5362,t5363,t5370,t5372,t5374,t5376,t5381,t5382,t5383,t5384,t5385,t5386,t5387,t5389,t5390,t5391,t5392,t5393,t5395,t5399,t5400,t5401,t5402,t5403,t5404,t5405,t5410,t5411,t5412,t5415,t5416,t5419,t5421,t5422,t5425,t5430,t5433,t5434,t5436,t5437,t5438,t5439,t5449,t5451,t5452,t5453,t5454,t5455,t5456,t5457,t5458,t5459,t5460,t5464,t5465,t5466,t5467,t5468,t5480,t5481,t5483,t5486,t5487,t5488,t5490,t5491,t5493,t5494,t5495,t5496,t5497,t5499,t5508,t5515,t5523,t5535,t5536,t5537,t5538,t5539,t5542,t5543,t5544,t5545,t5547,t5548,t5549,t5550,t5553,t5554,t5555,t5556,t5557,t5558,t5560,t5563,t5564,t5565,t5567,t5568,t5569,t5570,t5572,t5573,t5574,t5575,t5576,t5577,t5578,t5579,t5580,t5581,t5584,t5585,t5586,t5587,t5589,t5590,t5592,t5593,t5594,t5598,t5599,t56,t5603,t5604,t5605,t5607,t5611,t5612,t5613,t5614,t5615,t5616,t5618,t5624,t5626,t5628,t5631,t5632,t5636,t5637,t5638,t5641,t5642,t5643,t5645,t5646,t5647,t5649,t5650,t5651,t5652,t5653,t5658,t5669,t5673,t5675,t5677,t5678,t5679,t5680,t5682,t5684,t5685,t5686,t5687,t5688,t5689,t5690,t5691,t5694,t5695,t5698,t5699,t5713,t5714,t5717,t5718,t5720,t5721,t5722,t5723,t5724,t5725,t5730,t5731,t5734,t5735,t5738,t5739,t5741,t5742,t5745,t5747,t5751,t5753,t5758,t5759,t5760,t5761,t5762,t5763,t5764,t5765,t5766,t5767,t5768,t5769,t5770,t5771,t5772,t5773,t5774,t5775,t5777,t5779,t5781,t5782,t5783,t5784,t5787,t5788,t5790,t5791,t5792,t5793,t5796,t5798,t5802,t5804,t5809,t5813,t5814,t5816,t5817,t5819,t5820,t5821,t5825,t5826,t5827,t5828,t5829,t5835,t5836,t5839,t5840,t5842,t5844,t5846,t5848,t5849,t5851,t5853,t5855,t5856,t5857,t5858,t5859,t5860,t5867,t5868,t5869,t5870,t5871,t5872,t5874,t5875,t5876,t5877,t5878,t5879,t5880,t5881,t5882,t5884,t5886,t5890,t5891,t5892,t5893,t5894,t5896,t5897,t5898,t5899,t5900,t5901,t5902,t5904,t5905,t5907,t5908,t5909,t5910,t5911,t5913,t5914,t5915,t5916,t5917,t5918,t5919,t5920,t5922,t5924,t5925,t5926,t5927,t5928,t5930,t5931,t5933,t5934,t5937,t5938,t5939,t5941,t5945,t5946,t5947,t5949,t5950,t5951,t5954,t5955,t5956,t5957,t5958,t5959,t5960,t5962,t5966,t5967,t5968,t5969,t5970,t5974,t5975,t5976,t5977,t5978,t5979,t5980,t5981,t5982,t5986,t5988,t5990,t5993,t5995,t5997,t5999,t60,t6000,t6001,t6004,t6005,t6006,t6007,t6008,t6009,t6010,t6011,t6013,t6014,t6015,t6019,t6020,t6022,t6023,t6024,t6026,t6028,t6031,t6032,t6039,t6041,t6043,t6045,t6046,t6047,t6050,t6053,t6054,t6055,t6058,t6059,t6060,t6062,t6064,t6065,t6066,t6067,t6074,t6076,t6080,t6081,t6083,t6086,t6087,t6088,t6091,t6093,t6094,t6095,t6096,t6098,t6100,t6102,t6110,t6111,t6112,t6115,t6116,t6119,t6121,t6125,t6129,t6131,t6133,t6134,t6135,t6137,t6141,t6143,t6144,t6149,t6151,t6152,t6153,t6156,t6157,t6159,t6160,t6162,t6164,t6166,t6168,t6169,t6170,t6171,t6172,t6173,t6174,t6175,t6177,t6178,t6179,t6180,t6182,t6183,t6184,t6185,t6186,t6187,t6188,t6189,t6190,t6192,t6193,t6194,t6195,t6196,t6200,t6201,t6202,t6205,t6206,t6207,t6208,t6209,t6210,t6217,t6219,t6223,t6225,t6226,t6227,t6228,t6230,t6231,t6233,t6234,t6237,t6238,t6239,t6240,t6241,t6244,t6250,t6251,t6255,t6256,t6257,t6261,t6262,t6263,t6266,t6270,t6271,t6272,t6275,t6281,t6283,t6284,t6287,t6290,t6291,t6292,t6295,t6296,t6297,t6299,t6300,t6302,t6303,t6304,t6305,t6306,t6307,t6308,t6309,t6311,t6312,t6314,t6316,t6319,t6323,t6324,t6326,t6341,t6342,t6343,t6346,t6347,t6354,t6355,t6357,t6358,t6360,t6361,t6362,t6364,t6366,t6367,t6368,t6369,t6371,t6372,t6373,t6376,t6377,t6379,t6384,t6392,t6394,t6395,t6396,t6398,t6402,t6407,t6409,t6413,t6418,t6419,t642,t6421,t6423,t6425,t6428,t6429,t643,t6431,t6432,t6433,t6435,t6436,t6437,t6438,t6440,t6442,t6443,t6445,t6447,t6450,t6452,t6453,t6455,t6457,t6458,t6459,t6460,t6461,t6462,t6464,t6465,t6466,t6467,t6468,t6469,t6476,t6478,t6480,t6481,t6482,t6483,t6484,t649,t6490,t6491,t6493,t6501,t6502,t6503,t6504,t6505,t6507,t6508,t6509,t6510,t6512,t6513,t6514,t6515,t6517,t6518,t6519,t6520,t6521,t6522,t6523,t6524,t6525,t6526,t6527,t6528,t6539,t6540,t6547,t6548,t6549,t6550,t6551,t6552,t6554,t6555,t6556,t6557,t6558,t6561,t6562,t6564,t6565,t6568,t6569,t6570,t6571,t6572,t6574,t6575,t6576,t6580,t6582,t6584,t6585,t6589,t6593,t6594,t6595,t6596,t6601,t6602,t6607,t6608,t6609,t6610,t6611,t6612,t6613,t6614,t6616,t6617,t6618,t6619,t6620,t6622,t6623,t6625,t6626,t6627,t6628,t6629,t6632,t6633,t6634,t6635,t6636,t6637,t6638,t6639,t6640,t6641,t6642,t6643,t6645,t6646,t6647,t6648,t6649,t6650,t6651,t6654,t6656,t6657,t6658,t6663,t6664,t6665,t667,t6671,t6672,t6673,t6674,t6675,t6678,t6679,t6680,t6681,t6682,t6683,t6684,t6685,t6686,t6687,t6688,t6689,t6690,t6691,t6692,t6693,t6694,t6695,t6696,t6699,t670,t6700,t6701,t6702,t6703,t6704,t6705,t6706,t6707,t6708,t6709,t6711,t6717,t6719,t6722,t6724,t6725,t6727,t6728,t6731,t6732,t6736,t6737,t6738,t6739,t674,t6740,t6742,t6743,t6744,t6745,t6746,t6747,t6750,t6751,t6754,t6756,t6757,t6758,t6760,t6762,t6763,t6764,t6765,t6766,t6767,t6768,t6769,t6770,t6771,t6772,t6773,t6774,t6775,t6776,t6778,t6779,t6780,t6781,t6782,t6783,t6784,t6785,t6786,t6787,t6788,t6789,t6791,t6792,t6793,t6795,t6796,t6797,t6798,t6799,t6800,t6803,t6804,t6808,t6810,t6813,t6814,t6816,t6817,t6819,t6820,t6821,t6822,t6823,t6824,t6825,t6826,t6827,t6828,t6831,t6833,t6836,t6838,t6839,t684,t6841,t6842,t6843,t6844,t6848,t6849,t685,t6851,t6852,t6853,t6855,t6858,t6859,t686,t6866,t6867,t6868,t687,t6870,t6872,t6873,t6875,t6877,t6878,t6879,t6880,t6882,t6883,t6884,t6885,t6886,t6887,t6888,t6889,t6894,t6897,t6900,t6902,t6903,t6904,t6908,t6909,t6910,t6911,t6912,t6913,t6916,t6918,t6919,t6920,t6924,t6925,t6929,t6931,t6932,t6933,t6941,t6942,t6945,t6949,t6950,t6951,t6959,t6962,t6964,t6965,t6966,t6968,t6971,t6972,t6975,t6976,t6979,t6983,t6985,t6987,t6989,t6992,t6993,t6994,t6995,t6996,t6997,t7000,t7001,t7003,t7005,t7007,t7009,t7010,t7011,t7012,t7014,t7016,t7019,t7020,t7022,t7023,t7024,t7025,t7026,t7028,t7029,t7030,t7031,t7032,t7033,t7034,t7035,t7036,t7037,t7038,t7039,t7040,t7041,t7042,t7043,t7047,t7048,t7049,t7051,t7052,t7055,t7057,t7059,t7060,t7061,t7062,t7063,t7064,t7066,t707,t7072,t7073,t7074,t7076,t7078,t7079,t708,t7080,t7083,t7084,t7086,t7088,t7090,t7092,t7095,t7098,t710,t7101,t7102,t7108,t7109,t7111,t7112,t7114,t7118,t7125,t7127,t7128,t7131,t7132,t7133,t7134,t7140,t7142,t7148,t7149,t7150,t7156,t7159,t7161,t7162,t7164,t7166,t7170,t7171,t7174,t7176,t7179,t7181,t7182,t7184,t7186,t7187,t7195,t7196,t7197,t7199,t7200,t7203,t7204,t7205,t7206,t7208,t721,t7211,t7213,t7215,t7216,t7217,t7218,t7219,t722,t7220,t7221,t7222,t7224,t7226,t7228,t7229,t7230,t7231,t7232,t7233,t7234,t7235,t7237,t7238,t724,t7240,t7243,t7244,t7246,t7248,t7249,t7251,t7253,t7254,t7255,t7256,t7257,t7260,t7261,t7262,t7263,t7265,t7266,t7267,t7268,t7269,t7271,t7272,t7273,t7274,t7275,t7277,t7279,t7281,t7283,t7292,t7294,t7295,t7298,t7300,t7301,t7302,t7303,t7304,t7307,t7310,t7311,t7312,t7315,t7316,t7319,t7323,t7324,t7326,t7327,t7328,t7329,t7335,t7336,t7337,t7342,t7343,t7344,t7345,t7346,t7347,t7349,t7351,t7352,t7353,t7354,t7355,t7356,t7358,t7359,t7360,t7363,t7364,t7367,t7368,t7369,t7370,t7378,t7379,t7380,t7385,t7387,t7388,t7390,t7391,t7392,t7393,t7394,t7396,t7397,t7398,t7399,t7401,t7402,t7404,t7405,t7406,t7407,t7408,t7409,t7410,t7411,t7412,t7413,t7414,t7415,t7416,t7417,t7419,t7420,t7421,t7424,t7425,t7432,t7433,t7436,t7439,t7441,t7443,t7444,t7446,t7447,t7448,t7450,t7451,t7453,t7454,t7456,t7458,t7462,t7463,t7469,t7470,t7472,t7473,t7479,t7480,t7482,t7483,t7487,t7489,t749,t7490,t7491,t7493,t7494,t7501,t7511,t7512,t7514,t7518,t7519,t7523,t7524,t7525,t7526,t7532,t7534,t7535,t7537,t7538,t7544,t7548,t7553,t7554,t7560,t7561,t7562,t7596,t7599,t7601,t7607,t7609,t7610,t7611,t7612,t7613,t7614,t7615,t762,t7624,t7626,t7630,t7631,t7638,t7639,t7641,t7652,t7654,t7655,t7656,t7658,t7662,t7663,t7664,t7665,t7668,t7670,t7672,t7675,t7676,t7677,t768,t7682,t7683,t7686,t7688,t7690,t7691,t7692,t7695,t7696,t7697,t7704,t7707,t7710,t7711,t7712,t7713,t7715,t7716,t7724,t7725,t7727,t7730,t7736,t7737,t7738,t7746,t7752,t7753,t7756,t7763,t777,t7773,t7784,t7789,t7790,t7791,t7792,t7796,t7798,t7804,t7805,t7807,t7808,t7809,t7811,t7814,t7815,t7816,t7817,t7820,t7822,t7823,t7824,t7826,t7827,t7828,t7830,t7835,t7836,t7838,t7839,t7840,t7841,t7842,t7845,t7847,t7848,t7850,t7859,t7860,t7868,t7869,t7880,t7885,t7888,t7891,t7894,t7895,t7897,t7900,t7902,t7909,t7919,t792,t7920,t7921,t7922,t7923,t7924,t7925,t7926,t793,t7938,t7939,t7940,t7948,t7949,t7951,t7952,t7953,t7955,t7957,t7965,t7966,t7975,t7976,t8,t801,t802,t808,t813,t819,t821,t850,t855,t874,t878,t9,t941,t948,t951});
end
function tau_c = ft_16(ct)
dq1 = ct{1};
dq2 = ct{2};
dq3 = ct{3};
dq4 = ct{4};
dq5 = ct{5};
dq6 = ct{6};
t10 = ct{7};
t1005 = ct{8};
t1022 = ct{9};
t1089 = ct{10};
t11 = ct{11};
t1104 = ct{12};
t1105 = ct{13};
t1108 = ct{14};
t1115 = ct{15};
t1121 = ct{16};
t1158 = ct{17};
t1159 = ct{18};
t1196 = ct{19};
t12 = ct{20};
t1205 = ct{21};
t1210 = ct{22};
t1212 = ct{23};
t1217 = ct{24};
t1218 = ct{25};
t123 = ct{26};
t1237 = ct{27};
t1238 = ct{28};
t1288 = ct{29};
t1289 = ct{30};
t13 = ct{31};
t1302 = ct{32};
t1303 = ct{33};
t1319 = ct{34};
t1320 = ct{35};
t1336 = ct{36};
t1348 = ct{37};
t1350 = ct{38};
t1351 = ct{39};
t1360 = ct{40};
t1369 = ct{41};
t1378 = ct{42};
t1396 = ct{43};
t14 = ct{44};
t140 = ct{45};
t1425 = ct{46};
t1435 = ct{47};
t1456 = ct{48};
t1477 = ct{49};
t1488 = ct{50};
t15 = ct{51};
t1513 = ct{52};
t1539 = ct{53};
t1554 = ct{54};
t1577 = ct{55};
t1578 = ct{56};
t1586 = ct{57};
t1587 = ct{58};
t16 = ct{59};
t1600 = ct{60};
t1606 = ct{61};
t1608 = ct{62};
t1609 = ct{63};
t1629 = ct{64};
t1637 = ct{65};
t1640 = ct{66};
t1641 = ct{67};
t1659 = ct{68};
t1661 = ct{69};
t1666 = ct{70};
t1667 = ct{71};
t1683 = ct{72};
t1686 = ct{73};
t1690 = ct{74};
t1692 = ct{75};
t17 = ct{76};
t1700 = ct{77};
t1701 = ct{78};
t1705 = ct{79};
t1712 = ct{80};
t1758 = ct{81};
t1759 = ct{82};
t1775 = ct{83};
t1776 = ct{84};
t18 = ct{85};
t1861 = ct{86};
t1874 = ct{87};
t1879 = ct{88};
t188 = ct{89};
t1881 = ct{90};
t189 = ct{91};
t1896 = ct{92};
t19 = ct{93};
t1901 = ct{94};
t1941 = ct{95};
t1959 = ct{96};
t1973 = ct{97};
t1993 = ct{98};
t1994 = ct{99};
t20 = ct{100};
t201 = ct{101};
t202 = ct{102};
t2023 = ct{103};
t2053 = ct{104};
t2060 = ct{105};
t2089 = ct{106};
t2090 = ct{107};
t2098 = ct{108};
t2099 = ct{109};
t21 = ct{110};
t2117 = ct{111};
t2120 = ct{112};
t2122 = ct{113};
t2123 = ct{114};
t2139 = ct{115};
t2140 = ct{116};
t2147 = ct{117};
t2152 = ct{118};
t2154 = ct{119};
t2155 = ct{120};
t2159 = ct{121};
t2165 = ct{122};
t2174 = ct{123};
t2183 = ct{124};
t2187 = ct{125};
t2193 = ct{126};
t2194 = ct{127};
t2195 = ct{128};
t2199 = ct{129};
t22 = ct{130};
t2203 = ct{131};
t2215 = ct{132};
t2219 = ct{133};
t2222 = ct{134};
t2223 = ct{135};
t2239 = ct{136};
t2240 = ct{137};
t2256 = ct{138};
t2257 = ct{139};
t2292 = ct{140};
t2295 = ct{141};
t2297 = ct{142};
t2303 = ct{143};
t2306 = ct{144};
t2307 = ct{145};
t2317 = ct{146};
t2337 = ct{147};
t2338 = ct{148};
t2339 = ct{149};
t2355 = ct{150};
t236 = ct{151};
t2361 = ct{152};
t2362 = ct{153};
t2363 = ct{154};
t2367 = ct{155};
t2368 = ct{156};
t237 = ct{157};
t2371 = ct{158};
t238 = ct{159};
t2388 = ct{160};
t2399 = ct{161};
t24 = ct{162};
t241 = ct{163};
t2414 = ct{164};
t2419 = ct{165};
t25 = ct{166};
t2502 = ct{167};
t2519 = ct{168};
t2527 = ct{169};
t2555 = ct{170};
t2556 = ct{171};
t2572 = ct{172};
t2583 = ct{173};
t2598 = ct{174};
t26 = ct{175};
t2605 = ct{176};
t2606 = ct{177};
t2612 = ct{178};
t2613 = ct{179};
t2618 = ct{180};
t2619 = ct{181};
t262 = ct{182};
t264 = ct{183};
t2651 = ct{184};
t2652 = ct{185};
t2671 = ct{186};
t2674 = ct{187};
t2676 = ct{188};
t2683 = ct{189};
t2684 = ct{190};
t2689 = ct{191};
t2694 = ct{192};
t2695 = ct{193};
t2698 = ct{194};
t27 = ct{195};
t2701 = ct{196};
t2707 = ct{197};
t2716 = ct{198};
t2719 = ct{199};
t2740 = ct{200};
t2747 = ct{201};
t2748 = ct{202};
t2749 = ct{203};
t2754 = ct{204};
t2773 = ct{205};
t2781 = ct{206};
t2788 = ct{207};
t28 = ct{208};
t2801 = ct{209};
t2804 = ct{210};
t2813 = ct{211};
t2814 = ct{212};
t2820 = ct{213};
t2831 = ct{214};
t2834 = ct{215};
t2835 = ct{216};
t2838 = ct{217};
t2850 = ct{218};
t2851 = ct{219};
t29 = ct{220};
t2953 = ct{221};
t2965 = ct{222};
t2966 = ct{223};
t2990 = ct{224};
t2991 = ct{225};
t2994 = ct{226};
t30 = ct{227};
t3009 = ct{228};
t3015 = ct{229};
t3022 = ct{230};
t3027 = ct{231};
t3030 = ct{232};
t3036 = ct{233};
t3043 = ct{234};
t3047 = ct{235};
t3055 = ct{236};
t3057 = ct{237};
t3058 = ct{238};
t3064 = ct{239};
t3068 = ct{240};
t3072 = ct{241};
t3080 = ct{242};
t3096 = ct{243};
t3097 = ct{244};
t31 = ct{245};
t3109 = ct{246};
t3117 = ct{247};
t3118 = ct{248};
t3121 = ct{249};
t3122 = ct{250};
t3126 = ct{251};
t3129 = ct{252};
t313 = ct{253};
t3131 = ct{254};
t3132 = ct{255};
t3133 = ct{256};
t314 = ct{257};
t3145 = ct{258};
t3148 = ct{259};
t3157 = ct{260};
t3158 = ct{261};
t3171 = ct{262};
t3193 = ct{263};
t3194 = ct{264};
t3195 = ct{265};
t32 = ct{266};
t3200 = ct{267};
t3201 = ct{268};
t3205 = ct{269};
t3208 = ct{270};
t3209 = ct{271};
t321 = ct{272};
t3211 = ct{273};
t3213 = ct{274};
t3216 = ct{275};
t3217 = ct{276};
t3221 = ct{277};
t3235 = ct{278};
t3236 = ct{279};
t3237 = ct{280};
t3238 = ct{281};
t3239 = ct{282};
t3242 = ct{283};
t3276 = ct{284};
t3277 = ct{285};
t3279 = ct{286};
t3290 = ct{287};
t3297 = ct{288};
t3299 = ct{289};
t33 = ct{290};
t3303 = ct{291};
t3312 = ct{292};
t3313 = ct{293};
t3315 = ct{294};
t3318 = ct{295};
t332 = ct{296};
t3322 = ct{297};
t3324 = ct{298};
t3328 = ct{299};
t3329 = ct{300};
t3337 = ct{301};
t3340 = ct{302};
t3344 = ct{303};
t335 = ct{304};
t3351 = ct{305};
t3359 = ct{306};
t3369 = ct{307};
t3370 = ct{308};
t3386 = ct{309};
t3395 = ct{310};
t3396 = ct{311};
t34 = ct{312};
t3405 = ct{313};
t3409 = ct{314};
t3415 = ct{315};
t3416 = ct{316};
t3420 = ct{317};
t3423 = ct{318};
t3428 = ct{319};
t3431 = ct{320};
t3432 = ct{321};
t3434 = ct{322};
t3435 = ct{323};
t3446 = ct{324};
t3448 = ct{325};
t3463 = ct{326};
t3468 = ct{327};
t3471 = ct{328};
t3474 = ct{329};
t3480 = ct{330};
t3482 = ct{331};
t3483 = ct{332};
t3488 = ct{333};
t3490 = ct{334};
t3496 = ct{335};
t3499 = ct{336};
t35 = ct{337};
t350 = ct{338};
t3500 = ct{339};
t3502 = ct{340};
t3503 = ct{341};
t3512 = ct{342};
t3517 = ct{343};
t3524 = ct{344};
t3543 = ct{345};
t3547 = ct{346};
t3554 = ct{347};
t3563 = ct{348};
t3566 = ct{349};
t3582 = ct{350};
t3588 = ct{351};
t3590 = ct{352};
t3591 = ct{353};
t3592 = ct{354};
t3597 = ct{355};
t36 = ct{356};
t3603 = ct{357};
t3609 = ct{358};
t3611 = ct{359};
t3614 = ct{360};
t3638 = ct{361};
t3639 = ct{362};
t3640 = ct{363};
t3641 = ct{364};
t3642 = ct{365};
t3643 = ct{366};
t3649 = ct{367};
t3655 = ct{368};
t3658 = ct{369};
t3659 = ct{370};
t366 = ct{371};
t3670 = ct{372};
t3688 = ct{373};
t3689 = ct{374};
t3703 = ct{375};
t3704 = ct{376};
t3707 = ct{377};
t3708 = ct{378};
t3712 = ct{379};
t3716 = ct{380};
t3717 = ct{381};
t3739 = ct{382};
t3746 = ct{383};
t3755 = ct{384};
t3765 = ct{385};
t3766 = ct{386};
t3770 = ct{387};
t38 = ct{388};
t3805 = ct{389};
t3808 = ct{390};
t3809 = ct{391};
t3810 = ct{392};
t3817 = ct{393};
t3818 = ct{394};
t3820 = ct{395};
t3821 = ct{396};
t3823 = ct{397};
t3840 = ct{398};
t3846 = ct{399};
t3856 = ct{400};
t3862 = ct{401};
t3863 = ct{402};
t3876 = ct{403};
t3877 = ct{404};
t3878 = ct{405};
t3879 = ct{406};
t3880 = ct{407};
t3890 = ct{408};
t3891 = ct{409};
t3893 = ct{410};
t3895 = ct{411};
t3896 = ct{412};
t3897 = ct{413};
t3898 = ct{414};
t39 = ct{415};
t3901 = ct{416};
t3902 = ct{417};
t3903 = ct{418};
t3906 = ct{419};
t3910 = ct{420};
t3913 = ct{421};
t3915 = ct{422};
t3924 = ct{423};
t3925 = ct{424};
t3931 = ct{425};
t3934 = ct{426};
t3937 = ct{427};
t3943 = ct{428};
t3951 = ct{429};
t3961 = ct{430};
t3967 = ct{431};
t3968 = ct{432};
t3974 = ct{433};
t3975 = ct{434};
t3976 = ct{435};
t3980 = ct{436};
t3985 = ct{437};
t3991 = ct{438};
t3993 = ct{439};
t4001 = ct{440};
t4006 = ct{441};
t4008 = ct{442};
t4018 = ct{443};
t4019 = ct{444};
t4026 = ct{445};
t4030 = ct{446};
t4031 = ct{447};
t4032 = ct{448};
t4035 = ct{449};
t4039 = ct{450};
t4041 = ct{451};
t4045 = ct{452};
t4047 = ct{453};
t4049 = ct{454};
t4051 = ct{455};
t4053 = ct{456};
t4054 = ct{457};
t4065 = ct{458};
t410 = ct{459};
t4100 = ct{460};
t4109 = ct{461};
t4110 = ct{462};
t4114 = ct{463};
t4115 = ct{464};
t4118 = ct{465};
t4146 = ct{466};
t4147 = ct{467};
t4153 = ct{468};
t4154 = ct{469};
t4157 = ct{470};
t4158 = ct{471};
t4165 = ct{472};
t4172 = ct{473};
t4187 = ct{474};
t4198 = ct{475};
t42 = ct{476};
t4201 = ct{477};
t4205 = ct{478};
t4208 = ct{479};
t4213 = ct{480};
t4215 = ct{481};
t4236 = ct{482};
t4240 = ct{483};
t4244 = ct{484};
t4260 = ct{485};
t4261 = ct{486};
t4263 = ct{487};
t4270 = ct{488};
t4272 = ct{489};
t4273 = ct{490};
t4274 = ct{491};
t4275 = ct{492};
t4281 = ct{493};
t4282 = ct{494};
t4286 = ct{495};
t4287 = ct{496};
t4288 = ct{497};
t4299 = ct{498};
t43 = ct{499};
t4300 = ct{500};
t4301 = ct{501};
t4303 = ct{502};
t4308 = ct{503};
t4310 = ct{504};
t4313 = ct{505};
t4314 = ct{506};
t4318 = ct{507};
t4324 = ct{508};
t4325 = ct{509};
t4326 = ct{510};
t4330 = ct{511};
t4332 = ct{512};
t4334 = ct{513};
t4337 = ct{514};
t4339 = ct{515};
t4341 = ct{516};
t4342 = ct{517};
t4343 = ct{518};
t4346 = ct{519};
t4352 = ct{520};
t4359 = ct{521};
t4371 = ct{522};
t4372 = ct{523};
t4373 = ct{524};
t4375 = ct{525};
t4413 = ct{526};
t4415 = ct{527};
t4416 = ct{528};
t4417 = ct{529};
t4458 = ct{530};
t4461 = ct{531};
t4464 = ct{532};
t4468 = ct{533};
t4470 = ct{534};
t4476 = ct{535};
t4486 = ct{536};
t4488 = ct{537};
t4489 = ct{538};
t4494 = ct{539};
t4495 = ct{540};
t4501 = ct{541};
t4502 = ct{542};
t4504 = ct{543};
t4515 = ct{544};
t4518 = ct{545};
t4553 = ct{546};
t4559 = ct{547};
t4562 = ct{548};
t4563 = ct{549};
t4567 = ct{550};
t4570 = ct{551};
t4573 = ct{552};
t4576 = ct{553};
t4577 = ct{554};
t4582 = ct{555};
t4583 = ct{556};
t4594 = ct{557};
t46 = ct{558};
t4603 = ct{559};
t4604 = ct{560};
t4606 = ct{561};
t4615 = ct{562};
t4617 = ct{563};
t4618 = ct{564};
t4619 = ct{565};
t4623 = ct{566};
t4634 = ct{567};
t4635 = ct{568};
t4639 = ct{569};
t4644 = ct{570};
t4645 = ct{571};
t4652 = ct{572};
t4658 = ct{573};
t4663 = ct{574};
t4665 = ct{575};
t4673 = ct{576};
t4675 = ct{577};
t4677 = ct{578};
t4678 = ct{579};
t4680 = ct{580};
t4683 = ct{581};
t47 = ct{582};
t4703 = ct{583};
t4704 = ct{584};
t4705 = ct{585};
t4708 = ct{586};
t4709 = ct{587};
t4713 = ct{588};
t4716 = ct{589};
t4719 = ct{590};
t4722 = ct{591};
t4724 = ct{592};
t4725 = ct{593};
t4728 = ct{594};
t4730 = ct{595};
t4741 = ct{596};
t4744 = ct{597};
t4746 = ct{598};
t4751 = ct{599};
t4757 = ct{600};
t4760 = ct{601};
t4761 = ct{602};
t4762 = ct{603};
t4763 = ct{604};
t4795 = ct{605};
t4799 = ct{606};
t4801 = ct{607};
t4808 = ct{608};
t4809 = ct{609};
t4814 = ct{610};
t4823 = ct{611};
t4828 = ct{612};
t4833 = ct{613};
t4835 = ct{614};
t4838 = ct{615};
t4843 = ct{616};
t4844 = ct{617};
t4847 = ct{618};
t4850 = ct{619};
t4853 = ct{620};
t4872 = ct{621};
t4874 = ct{622};
t4876 = ct{623};
t4879 = ct{624};
t4880 = ct{625};
t4887 = ct{626};
t4895 = ct{627};
t4902 = ct{628};
t4903 = ct{629};
t4904 = ct{630};
t4905 = ct{631};
t4906 = ct{632};
t4911 = ct{633};
t4912 = ct{634};
t4915 = ct{635};
t4920 = ct{636};
t4923 = ct{637};
t4924 = ct{638};
t4925 = ct{639};
t4927 = ct{640};
t4950 = ct{641};
t50 = ct{642};
t5014 = ct{643};
t5016 = ct{644};
t5025 = ct{645};
t5026 = ct{646};
t5027 = ct{647};
t5028 = ct{648};
t5034 = ct{649};
t5036 = ct{650};
t5037 = ct{651};
t5038 = ct{652};
t5041 = ct{653};
t5042 = ct{654};
t5043 = ct{655};
t5080 = ct{656};
t5082 = ct{657};
t5083 = ct{658};
t5084 = ct{659};
t5085 = ct{660};
t5086 = ct{661};
t5087 = ct{662};
t5088 = ct{663};
t5089 = ct{664};
t5090 = ct{665};
t5091 = ct{666};
t5093 = ct{667};
t5096 = ct{668};
t5097 = ct{669};
t5098 = ct{670};
t5103 = ct{671};
t5105 = ct{672};
t5106 = ct{673};
t5108 = ct{674};
t5119 = ct{675};
t5141 = ct{676};
t5142 = ct{677};
t5153 = ct{678};
t5154 = ct{679};
t5155 = ct{680};
t5161 = ct{681};
t5164 = ct{682};
t5167 = ct{683};
t5169 = ct{684};
t5183 = ct{685};
t5184 = ct{686};
t5185 = ct{687};
t5186 = ct{688};
t5189 = ct{689};
t5190 = ct{690};
t5194 = ct{691};
t5198 = ct{692};
t5200 = ct{693};
t5201 = ct{694};
t5202 = ct{695};
t5205 = ct{696};
t5213 = ct{697};
t5214 = ct{698};
t5234 = ct{699};
t5236 = ct{700};
t5240 = ct{701};
t5243 = ct{702};
t5246 = ct{703};
t5247 = ct{704};
t5248 = ct{705};
t5249 = ct{706};
t5251 = ct{707};
t5256 = ct{708};
t5257 = ct{709};
t5258 = ct{710};
t5259 = ct{711};
t5262 = ct{712};
t5264 = ct{713};
t5265 = ct{714};
t5278 = ct{715};
t5279 = ct{716};
t5280 = ct{717};
t5283 = ct{718};
t5286 = ct{719};
t5287 = ct{720};
t5291 = ct{721};
t5296 = ct{722};
t5297 = ct{723};
t5301 = ct{724};
t5302 = ct{725};
t5303 = ct{726};
t5304 = ct{727};
t5305 = ct{728};
t5306 = ct{729};
t5308 = ct{730};
t5309 = ct{731};
t5313 = ct{732};
t5328 = ct{733};
t5331 = ct{734};
t5332 = ct{735};
t5333 = ct{736};
t5336 = ct{737};
t5337 = ct{738};
t5340 = ct{739};
t5341 = ct{740};
t5343 = ct{741};
t5344 = ct{742};
t5345 = ct{743};
t5346 = ct{744};
t5352 = ct{745};
t5353 = ct{746};
t5356 = ct{747};
t5358 = ct{748};
t5359 = ct{749};
t5361 = ct{750};
t5362 = ct{751};
t5363 = ct{752};
t5370 = ct{753};
t5372 = ct{754};
t5374 = ct{755};
t5376 = ct{756};
t5381 = ct{757};
t5382 = ct{758};
t5383 = ct{759};
t5384 = ct{760};
t5385 = ct{761};
t5386 = ct{762};
t5387 = ct{763};
t5389 = ct{764};
t5390 = ct{765};
t5391 = ct{766};
t5392 = ct{767};
t5393 = ct{768};
t5395 = ct{769};
t5399 = ct{770};
t5400 = ct{771};
t5401 = ct{772};
t5402 = ct{773};
t5403 = ct{774};
t5404 = ct{775};
t5405 = ct{776};
t5410 = ct{777};
t5411 = ct{778};
t5412 = ct{779};
t5415 = ct{780};
t5416 = ct{781};
t5419 = ct{782};
t5421 = ct{783};
t5422 = ct{784};
t5425 = ct{785};
t5430 = ct{786};
t5433 = ct{787};
t5434 = ct{788};
t5436 = ct{789};
t5437 = ct{790};
t5438 = ct{791};
t5439 = ct{792};
t5449 = ct{793};
t5451 = ct{794};
t5452 = ct{795};
t5453 = ct{796};
t5454 = ct{797};
t5455 = ct{798};
t5456 = ct{799};
t5457 = ct{800};
t5458 = ct{801};
t5459 = ct{802};
t5460 = ct{803};
t5464 = ct{804};
t5465 = ct{805};
t5466 = ct{806};
t5467 = ct{807};
t5468 = ct{808};
t5480 = ct{809};
t5481 = ct{810};
t5483 = ct{811};
t5486 = ct{812};
t5487 = ct{813};
t5488 = ct{814};
t5490 = ct{815};
t5491 = ct{816};
t5493 = ct{817};
t5494 = ct{818};
t5495 = ct{819};
t5496 = ct{820};
t5497 = ct{821};
t5499 = ct{822};
t5508 = ct{823};
t5515 = ct{824};
t5523 = ct{825};
t5535 = ct{826};
t5536 = ct{827};
t5537 = ct{828};
t5538 = ct{829};
t5539 = ct{830};
t5542 = ct{831};
t5543 = ct{832};
t5544 = ct{833};
t5545 = ct{834};
t5547 = ct{835};
t5548 = ct{836};
t5549 = ct{837};
t5550 = ct{838};
t5553 = ct{839};
t5554 = ct{840};
t5555 = ct{841};
t5556 = ct{842};
t5557 = ct{843};
t5558 = ct{844};
t5560 = ct{845};
t5563 = ct{846};
t5564 = ct{847};
t5565 = ct{848};
t5567 = ct{849};
t5568 = ct{850};
t5569 = ct{851};
t5570 = ct{852};
t5572 = ct{853};
t5573 = ct{854};
t5574 = ct{855};
t5575 = ct{856};
t5576 = ct{857};
t5577 = ct{858};
t5578 = ct{859};
t5579 = ct{860};
t5580 = ct{861};
t5581 = ct{862};
t5584 = ct{863};
t5585 = ct{864};
t5586 = ct{865};
t5587 = ct{866};
t5589 = ct{867};
t5590 = ct{868};
t5592 = ct{869};
t5593 = ct{870};
t5594 = ct{871};
t5598 = ct{872};
t5599 = ct{873};
t56 = ct{874};
t5603 = ct{875};
t5604 = ct{876};
t5605 = ct{877};
t5607 = ct{878};
t5611 = ct{879};
t5612 = ct{880};
t5613 = ct{881};
t5614 = ct{882};
t5615 = ct{883};
t5616 = ct{884};
t5618 = ct{885};
t5624 = ct{886};
t5626 = ct{887};
t5628 = ct{888};
t5631 = ct{889};
t5632 = ct{890};
t5636 = ct{891};
t5637 = ct{892};
t5638 = ct{893};
t5641 = ct{894};
t5642 = ct{895};
t5643 = ct{896};
t5645 = ct{897};
t5646 = ct{898};
t5647 = ct{899};
t5649 = ct{900};
t5650 = ct{901};
t5651 = ct{902};
t5652 = ct{903};
t5653 = ct{904};
t5658 = ct{905};
t5669 = ct{906};
t5673 = ct{907};
t5675 = ct{908};
t5677 = ct{909};
t5678 = ct{910};
t5679 = ct{911};
t5680 = ct{912};
t5682 = ct{913};
t5684 = ct{914};
t5685 = ct{915};
t5686 = ct{916};
t5687 = ct{917};
t5688 = ct{918};
t5689 = ct{919};
t5690 = ct{920};
t5691 = ct{921};
t5694 = ct{922};
t5695 = ct{923};
t5698 = ct{924};
t5699 = ct{925};
t5713 = ct{926};
t5714 = ct{927};
t5717 = ct{928};
t5718 = ct{929};
t5720 = ct{930};
t5721 = ct{931};
t5722 = ct{932};
t5723 = ct{933};
t5724 = ct{934};
t5725 = ct{935};
t5730 = ct{936};
t5731 = ct{937};
t5734 = ct{938};
t5735 = ct{939};
t5738 = ct{940};
t5739 = ct{941};
t5741 = ct{942};
t5742 = ct{943};
t5745 = ct{944};
t5747 = ct{945};
t5751 = ct{946};
t5753 = ct{947};
t5758 = ct{948};
t5759 = ct{949};
t5760 = ct{950};
t5761 = ct{951};
t5762 = ct{952};
t5763 = ct{953};
t5764 = ct{954};
t5765 = ct{955};
t5766 = ct{956};
t5767 = ct{957};
t5768 = ct{958};
t5769 = ct{959};
t5770 = ct{960};
t5771 = ct{961};
t5772 = ct{962};
t5773 = ct{963};
t5774 = ct{964};
t5775 = ct{965};
t5777 = ct{966};
t5779 = ct{967};
t5781 = ct{968};
t5782 = ct{969};
t5783 = ct{970};
t5784 = ct{971};
t5787 = ct{972};
t5788 = ct{973};
t5790 = ct{974};
t5791 = ct{975};
t5792 = ct{976};
t5793 = ct{977};
t5796 = ct{978};
t5798 = ct{979};
t5802 = ct{980};
t5804 = ct{981};
t5809 = ct{982};
t5813 = ct{983};
t5814 = ct{984};
t5816 = ct{985};
t5817 = ct{986};
t5819 = ct{987};
t5820 = ct{988};
t5821 = ct{989};
t5825 = ct{990};
t5826 = ct{991};
t5827 = ct{992};
t5828 = ct{993};
t5829 = ct{994};
t5835 = ct{995};
t5836 = ct{996};
t5839 = ct{997};
t5840 = ct{998};
t5842 = ct{999};
t5844 = ct{1000};
t5846 = ct{1001};
t5848 = ct{1002};
t5849 = ct{1003};
t5851 = ct{1004};
t5853 = ct{1005};
t5855 = ct{1006};
t5856 = ct{1007};
t5857 = ct{1008};
t5858 = ct{1009};
t5859 = ct{1010};
t5860 = ct{1011};
t5867 = ct{1012};
t5868 = ct{1013};
t5869 = ct{1014};
t5870 = ct{1015};
t5871 = ct{1016};
t5872 = ct{1017};
t5874 = ct{1018};
t5875 = ct{1019};
t5876 = ct{1020};
t5877 = ct{1021};
t5878 = ct{1022};
t5879 = ct{1023};
t5880 = ct{1024};
t5881 = ct{1025};
t5882 = ct{1026};
t5884 = ct{1027};
t5886 = ct{1028};
t5890 = ct{1029};
t5891 = ct{1030};
t5892 = ct{1031};
t5893 = ct{1032};
t5894 = ct{1033};
t5896 = ct{1034};
t5897 = ct{1035};
t5898 = ct{1036};
t5899 = ct{1037};
t5900 = ct{1038};
t5901 = ct{1039};
t5902 = ct{1040};
t5904 = ct{1041};
t5905 = ct{1042};
t5907 = ct{1043};
t5908 = ct{1044};
t5909 = ct{1045};
t5910 = ct{1046};
t5911 = ct{1047};
t5913 = ct{1048};
t5914 = ct{1049};
t5915 = ct{1050};
t5916 = ct{1051};
t5917 = ct{1052};
t5918 = ct{1053};
t5919 = ct{1054};
t5920 = ct{1055};
t5922 = ct{1056};
t5924 = ct{1057};
t5925 = ct{1058};
t5926 = ct{1059};
t5927 = ct{1060};
t5928 = ct{1061};
t5930 = ct{1062};
t5931 = ct{1063};
t5933 = ct{1064};
t5934 = ct{1065};
t5937 = ct{1066};
t5938 = ct{1067};
t5939 = ct{1068};
t5941 = ct{1069};
t5945 = ct{1070};
t5946 = ct{1071};
t5947 = ct{1072};
t5949 = ct{1073};
t5950 = ct{1074};
t5951 = ct{1075};
t5954 = ct{1076};
t5955 = ct{1077};
t5956 = ct{1078};
t5957 = ct{1079};
t5958 = ct{1080};
t5959 = ct{1081};
t5960 = ct{1082};
t5962 = ct{1083};
t5966 = ct{1084};
t5967 = ct{1085};
t5968 = ct{1086};
t5969 = ct{1087};
t5970 = ct{1088};
t5974 = ct{1089};
t5975 = ct{1090};
t5976 = ct{1091};
t5977 = ct{1092};
t5978 = ct{1093};
t5979 = ct{1094};
t5980 = ct{1095};
t5981 = ct{1096};
t5982 = ct{1097};
t5986 = ct{1098};
t5988 = ct{1099};
t5990 = ct{1100};
t5993 = ct{1101};
t5995 = ct{1102};
t5997 = ct{1103};
t5999 = ct{1104};
t60 = ct{1105};
t6000 = ct{1106};
t6001 = ct{1107};
t6004 = ct{1108};
t6005 = ct{1109};
t6006 = ct{1110};
t6007 = ct{1111};
t6008 = ct{1112};
t6009 = ct{1113};
t6010 = ct{1114};
t6011 = ct{1115};
t6013 = ct{1116};
t6014 = ct{1117};
t6015 = ct{1118};
t6019 = ct{1119};
t6020 = ct{1120};
t6022 = ct{1121};
t6023 = ct{1122};
t6024 = ct{1123};
t6026 = ct{1124};
t6028 = ct{1125};
t6031 = ct{1126};
t6032 = ct{1127};
t6039 = ct{1128};
t6041 = ct{1129};
t6043 = ct{1130};
t6045 = ct{1131};
t6046 = ct{1132};
t6047 = ct{1133};
t6050 = ct{1134};
t6053 = ct{1135};
t6054 = ct{1136};
t6055 = ct{1137};
t6058 = ct{1138};
t6059 = ct{1139};
t6060 = ct{1140};
t6062 = ct{1141};
t6064 = ct{1142};
t6065 = ct{1143};
t6066 = ct{1144};
t6067 = ct{1145};
t6074 = ct{1146};
t6076 = ct{1147};
t6080 = ct{1148};
t6081 = ct{1149};
t6083 = ct{1150};
t6086 = ct{1151};
t6087 = ct{1152};
t6088 = ct{1153};
t6091 = ct{1154};
t6093 = ct{1155};
t6094 = ct{1156};
t6095 = ct{1157};
t6096 = ct{1158};
t6098 = ct{1159};
t6100 = ct{1160};
t6102 = ct{1161};
t6110 = ct{1162};
t6111 = ct{1163};
t6112 = ct{1164};
t6115 = ct{1165};
t6116 = ct{1166};
t6119 = ct{1167};
t6121 = ct{1168};
t6125 = ct{1169};
t6129 = ct{1170};
t6131 = ct{1171};
t6133 = ct{1172};
t6134 = ct{1173};
t6135 = ct{1174};
t6137 = ct{1175};
t6141 = ct{1176};
t6143 = ct{1177};
t6144 = ct{1178};
t6149 = ct{1179};
t6151 = ct{1180};
t6152 = ct{1181};
t6153 = ct{1182};
t6156 = ct{1183};
t6157 = ct{1184};
t6159 = ct{1185};
t6160 = ct{1186};
t6162 = ct{1187};
t6164 = ct{1188};
t6166 = ct{1189};
t6168 = ct{1190};
t6169 = ct{1191};
t6170 = ct{1192};
t6171 = ct{1193};
t6172 = ct{1194};
t6173 = ct{1195};
t6174 = ct{1196};
t6175 = ct{1197};
t6177 = ct{1198};
t6178 = ct{1199};
t6179 = ct{1200};
t6180 = ct{1201};
t6182 = ct{1202};
t6183 = ct{1203};
t6184 = ct{1204};
t6185 = ct{1205};
t6186 = ct{1206};
t6187 = ct{1207};
t6188 = ct{1208};
t6189 = ct{1209};
t6190 = ct{1210};
t6192 = ct{1211};
t6193 = ct{1212};
t6194 = ct{1213};
t6195 = ct{1214};
t6196 = ct{1215};
t6200 = ct{1216};
t6201 = ct{1217};
t6202 = ct{1218};
t6205 = ct{1219};
t6206 = ct{1220};
t6207 = ct{1221};
t6208 = ct{1222};
t6209 = ct{1223};
t6210 = ct{1224};
t6217 = ct{1225};
t6219 = ct{1226};
t6223 = ct{1227};
t6225 = ct{1228};
t6226 = ct{1229};
t6227 = ct{1230};
t6228 = ct{1231};
t6230 = ct{1232};
t6231 = ct{1233};
t6233 = ct{1234};
t6234 = ct{1235};
t6237 = ct{1236};
t6238 = ct{1237};
t6239 = ct{1238};
t6240 = ct{1239};
t6241 = ct{1240};
t6244 = ct{1241};
t6250 = ct{1242};
t6251 = ct{1243};
t6255 = ct{1244};
t6256 = ct{1245};
t6257 = ct{1246};
t6261 = ct{1247};
t6262 = ct{1248};
t6263 = ct{1249};
t6266 = ct{1250};
t6270 = ct{1251};
t6271 = ct{1252};
t6272 = ct{1253};
t6275 = ct{1254};
t6281 = ct{1255};
t6283 = ct{1256};
t6284 = ct{1257};
t6287 = ct{1258};
t6290 = ct{1259};
t6291 = ct{1260};
t6292 = ct{1261};
t6295 = ct{1262};
t6296 = ct{1263};
t6297 = ct{1264};
t6299 = ct{1265};
t6300 = ct{1266};
t6302 = ct{1267};
t6303 = ct{1268};
t6304 = ct{1269};
t6305 = ct{1270};
t6306 = ct{1271};
t6307 = ct{1272};
t6308 = ct{1273};
t6309 = ct{1274};
t6311 = ct{1275};
t6312 = ct{1276};
t6314 = ct{1277};
t6316 = ct{1278};
t6319 = ct{1279};
t6323 = ct{1280};
t6324 = ct{1281};
t6326 = ct{1282};
t6341 = ct{1283};
t6342 = ct{1284};
t6343 = ct{1285};
t6346 = ct{1286};
t6347 = ct{1287};
t6354 = ct{1288};
t6355 = ct{1289};
t6357 = ct{1290};
t6358 = ct{1291};
t6360 = ct{1292};
t6361 = ct{1293};
t6362 = ct{1294};
t6364 = ct{1295};
t6366 = ct{1296};
t6367 = ct{1297};
t6368 = ct{1298};
t6369 = ct{1299};
t6371 = ct{1300};
t6372 = ct{1301};
t6373 = ct{1302};
t6376 = ct{1303};
t6377 = ct{1304};
t6379 = ct{1305};
t6384 = ct{1306};
t6392 = ct{1307};
t6394 = ct{1308};
t6395 = ct{1309};
t6396 = ct{1310};
t6398 = ct{1311};
t6402 = ct{1312};
t6407 = ct{1313};
t6409 = ct{1314};
t6413 = ct{1315};
t6418 = ct{1316};
t6419 = ct{1317};
t642 = ct{1318};
t6421 = ct{1319};
t6423 = ct{1320};
t6425 = ct{1321};
t6428 = ct{1322};
t6429 = ct{1323};
t643 = ct{1324};
t6431 = ct{1325};
t6432 = ct{1326};
t6433 = ct{1327};
t6435 = ct{1328};
t6436 = ct{1329};
t6437 = ct{1330};
t6438 = ct{1331};
t6440 = ct{1332};
t6442 = ct{1333};
t6443 = ct{1334};
t6445 = ct{1335};
t6447 = ct{1336};
t6450 = ct{1337};
t6452 = ct{1338};
t6453 = ct{1339};
t6455 = ct{1340};
t6457 = ct{1341};
t6458 = ct{1342};
t6459 = ct{1343};
t6460 = ct{1344};
t6461 = ct{1345};
t6462 = ct{1346};
t6464 = ct{1347};
t6465 = ct{1348};
t6466 = ct{1349};
t6467 = ct{1350};
t6468 = ct{1351};
t6469 = ct{1352};
t6476 = ct{1353};
t6478 = ct{1354};
t6480 = ct{1355};
t6481 = ct{1356};
t6482 = ct{1357};
t6483 = ct{1358};
t6484 = ct{1359};
t649 = ct{1360};
t6490 = ct{1361};
t6491 = ct{1362};
t6493 = ct{1363};
t6501 = ct{1364};
t6502 = ct{1365};
t6503 = ct{1366};
t6504 = ct{1367};
t6505 = ct{1368};
t6507 = ct{1369};
t6508 = ct{1370};
t6509 = ct{1371};
t6510 = ct{1372};
t6512 = ct{1373};
t6513 = ct{1374};
t6514 = ct{1375};
t6515 = ct{1376};
t6517 = ct{1377};
t6518 = ct{1378};
t6519 = ct{1379};
t6520 = ct{1380};
t6521 = ct{1381};
t6522 = ct{1382};
t6523 = ct{1383};
t6524 = ct{1384};
t6525 = ct{1385};
t6526 = ct{1386};
t6527 = ct{1387};
t6528 = ct{1388};
t6539 = ct{1389};
t6540 = ct{1390};
t6547 = ct{1391};
t6548 = ct{1392};
t6549 = ct{1393};
t6550 = ct{1394};
t6551 = ct{1395};
t6552 = ct{1396};
t6554 = ct{1397};
t6555 = ct{1398};
t6556 = ct{1399};
t6557 = ct{1400};
t6558 = ct{1401};
t6561 = ct{1402};
t6562 = ct{1403};
t6564 = ct{1404};
t6565 = ct{1405};
t6568 = ct{1406};
t6569 = ct{1407};
t6570 = ct{1408};
t6571 = ct{1409};
t6572 = ct{1410};
t6574 = ct{1411};
t6575 = ct{1412};
t6576 = ct{1413};
t6580 = ct{1414};
t6582 = ct{1415};
t6584 = ct{1416};
t6585 = ct{1417};
t6589 = ct{1418};
t6593 = ct{1419};
t6594 = ct{1420};
t6595 = ct{1421};
t6596 = ct{1422};
t6601 = ct{1423};
t6602 = ct{1424};
t6607 = ct{1425};
t6608 = ct{1426};
t6609 = ct{1427};
t6610 = ct{1428};
t6611 = ct{1429};
t6612 = ct{1430};
t6613 = ct{1431};
t6614 = ct{1432};
t6616 = ct{1433};
t6617 = ct{1434};
t6618 = ct{1435};
t6619 = ct{1436};
t6620 = ct{1437};
t6622 = ct{1438};
t6623 = ct{1439};
t6625 = ct{1440};
t6626 = ct{1441};
t6627 = ct{1442};
t6628 = ct{1443};
t6629 = ct{1444};
t6632 = ct{1445};
t6633 = ct{1446};
t6634 = ct{1447};
t6635 = ct{1448};
t6636 = ct{1449};
t6637 = ct{1450};
t6638 = ct{1451};
t6639 = ct{1452};
t6640 = ct{1453};
t6641 = ct{1454};
t6642 = ct{1455};
t6643 = ct{1456};
t6645 = ct{1457};
t6646 = ct{1458};
t6647 = ct{1459};
t6648 = ct{1460};
t6649 = ct{1461};
t6650 = ct{1462};
t6651 = ct{1463};
t6654 = ct{1464};
t6656 = ct{1465};
t6657 = ct{1466};
t6658 = ct{1467};
t6663 = ct{1468};
t6664 = ct{1469};
t6665 = ct{1470};
t667 = ct{1471};
t6671 = ct{1472};
t6672 = ct{1473};
t6673 = ct{1474};
t6674 = ct{1475};
t6675 = ct{1476};
t6678 = ct{1477};
t6679 = ct{1478};
t6680 = ct{1479};
t6681 = ct{1480};
t6682 = ct{1481};
t6683 = ct{1482};
t6684 = ct{1483};
t6685 = ct{1484};
t6686 = ct{1485};
t6687 = ct{1486};
t6688 = ct{1487};
t6689 = ct{1488};
t6690 = ct{1489};
t6691 = ct{1490};
t6692 = ct{1491};
t6693 = ct{1492};
t6694 = ct{1493};
t6695 = ct{1494};
t6696 = ct{1495};
t6699 = ct{1496};
t670 = ct{1497};
t6700 = ct{1498};
t6701 = ct{1499};
t6702 = ct{1500};
t6703 = ct{1501};
t6704 = ct{1502};
t6705 = ct{1503};
t6706 = ct{1504};
t6707 = ct{1505};
t6708 = ct{1506};
t6709 = ct{1507};
t6711 = ct{1508};
t6717 = ct{1509};
t6719 = ct{1510};
